simulink model "A_CT_ur10v"  (R2021b)
(part 5 of 11)

t2994 = ct{1294};
t2995 = ct{1295};
t2996 = ct{1296};
t2997 = ct{1297};
t2998 = ct{1298};
t2999 = ct{1299};
t2d = ct{1300};
t2dd = ct{1301};
t30 = ct{1302};
t3004 = ct{1303};
t3005 = ct{1304};
t3007 = ct{1305};
t3008 = ct{1306};
t3009 = ct{1307};
t301 = ct{1308};
t3010 = ct{1309};
t3011 = ct{1310};
t3012 = ct{1311};
t3013 = ct{1312};
t3014 = ct{1313};
t3016 = ct{1314};
t3017 = ct{1315};
t3018 = ct{1316};
t3019 = ct{1317};
t3020 = ct{1318};
t3021 = ct{1319};
t3024 = ct{1320};
t3025 = ct{1321};
t3027 = ct{1322};
t3028 = ct{1323};
t3029 = ct{1324};
t3031 = ct{1325};
t3032 = ct{1326};
t3035 = ct{1327};
t3036 = ct{1328};
t3037 = ct{1329};
t3040 = ct{1330};
t3041 = ct{1331};
t3042 = ct{1332};
t3043 = ct{1333};
t3044 = ct{1334};
t3047 = ct{1335};
t3049 = ct{1336};
t3055 = ct{1337};
t3056 = ct{1338};
t3058 = ct{1339};
t3059 = ct{1340};
t3061 = ct{1341};
t3064 = ct{1342};
t3065 = ct{1343};
t3066 = ct{1344};
t3067 = ct{1345};
t3068 = ct{1346};
t3069 = ct{1347};
t3073 = ct{1348};
t3074 = ct{1349};
t3076 = ct{1350};
t3078 = ct{1351};
t3079 = ct{1352};
t308 = ct{1353};
t3080 = ct{1354};
t3081 = ct{1355};
t3082 = ct{1356};
t3083 = ct{1357};
t3086 = ct{1358};
t3087 = ct{1359};
t3088 = ct{1360};
t3090 = ct{1361};
t3091 = ct{1362};
t3095 = ct{1363};
t3096 = ct{1364};
t3097 = ct{1365};
t3098 = ct{1366};
t3099 = ct{1367};
t31 = ct{1368};
t3100 = ct{1369};
t3101 = ct{1370};
t3104 = ct{1371};
t3106 = ct{1372};
t3107 = ct{1373};
t3110 = ct{1374};
t3111 = ct{1375};
t3112 = ct{1376};
t3121 = ct{1377};
t3123 = ct{1378};
t3124 = ct{1379};
t3125 = ct{1380};
t3129 = ct{1381};
t3130 = ct{1382};
t3134 = ct{1383};
t3136 = ct{1384};
t3137 = ct{1385};
t3140 = ct{1386};
t3143 = ct{1387};
t3146 = ct{1388};
t315 = ct{1389};
t3150 = ct{1390};
t3151 = ct{1391};
t3152 = ct{1392};
t3153 = ct{1393};
t3156 = ct{1394};
t3158 = ct{1395};
t3159 = ct{1396};
t3162 = ct{1397};
t3163 = ct{1398};
t3165 = ct{1399};
t3166 = ct{1400};
t3168 = ct{1401};
t3169 = ct{1402};
t317 = ct{1403};
t3174 = ct{1404};
t3175 = ct{1405};
t3176 = ct{1406};
t3177 = ct{1407};
t3179 = ct{1408};
t318 = ct{1409};
t3182 = ct{1410};
t3183 = ct{1411};
t3185 = ct{1412};
t3187 = ct{1413};
t319 = ct{1414};
t3204 = ct{1415};
t321 = ct{1416};
t3214 = ct{1417};
t3220 = ct{1418};
t3230 = ct{1419};
t3231 = ct{1420};
t3232 = ct{1421};
t3234 = ct{1422};
t3235 = ct{1423};
t3236 = ct{1424};
t3237 = ct{1425};
t3238 = ct{1426};
t3240 = ct{1427};
t3246 = ct{1428};
t325 = ct{1429};
t3250 = ct{1430};
t3251 = ct{1431};
t3259 = ct{1432};
t3260 = ct{1433};
t3272 = ct{1434};
t3283 = ct{1435};
t3285 = ct{1436};
t3288 = ct{1437};
t3289 = ct{1438};
t329 = ct{1439};
t3291 = ct{1440};
t3292 = ct{1441};
t3298 = ct{1442};
t330 = ct{1443};
t3306 = ct{1444};
t3308 = ct{1445};
t331 = ct{1446};
t3318 = ct{1447};
t332 = ct{1448};
t3321 = ct{1449};
t3326 = ct{1450};
t333 = ct{1451};
t3330 = ct{1452};
t3331 = ct{1453};
t3332 = ct{1454};
t3335 = ct{1455};
t3340 = ct{1456};
t3348 = ct{1457};
t3349 = ct{1458};
t3351 = ct{1459};
t3354 = ct{1460};
t3355 = ct{1461};
t3357 = ct{1462};
t3358 = ct{1463};
t3359 = ct{1464};
t3360 = ct{1465};
t3377 = ct{1466};
t3380 = ct{1467};
t3381 = ct{1468};
t3383 = ct{1469};
t3384 = ct{1470};
t3388 = ct{1471};
t3390 = ct{1472};
t3391 = ct{1473};
t3399 = ct{1474};
t34 = ct{1475};
t3400 = ct{1476};
t3401 = ct{1477};
t3404 = ct{1478};
t3405 = ct{1479};
t341 = ct{1480};
t3414 = ct{1481};
t3415 = ct{1482};
t3416 = ct{1483};
t342 = ct{1484};
t3421 = ct{1485};
t3428 = ct{1486};
t3429 = ct{1487};
t343 = ct{1488};
t3431 = ct{1489};
t3432 = ct{1490};
t3439 = ct{1491};
t344 = ct{1492};
t3440 = ct{1493};
t3445 = ct{1494};
t345 = ct{1495};
t3452 = ct{1496};
t3456 = ct{1497};
t3457 = ct{1498};
t3458 = ct{1499};
t3459 = ct{1500};
t346 = ct{1501};
t3460 = ct{1502};
t3461 = ct{1503};
t3464 = ct{1504};
t3468 = ct{1505};
t3469 = ct{1506};
t347 = ct{1507};
t3472 = ct{1508};
t3473 = ct{1509};
t3477 = ct{1510};
t3478 = ct{1511};
t3483 = ct{1512};
t3487 = ct{1513};
t3488 = ct{1514};
t35 = ct{1515};
t3504 = ct{1516};
t3509 = ct{1517};
t3510 = ct{1518};
t3516 = ct{1519};
t3517 = ct{1520};
t3521 = ct{1521};
t3522 = ct{1522};
t3523 = ct{1523};
t3532 = ct{1524};
t354 = ct{1525};
t3543 = ct{1526};
t3544 = ct{1527};
t3546 = ct{1528};
t3555 = ct{1529};
t3556 = ct{1530};
t3557 = ct{1531};
t3562 = ct{1532};
t3567 = ct{1533};
t3568 = ct{1534};
t3574 = ct{1535};
t3575 = ct{1536};
t3577 = ct{1537};
t3578 = ct{1538};
t3579 = ct{1539};
t3580 = ct{1540};
t3582 = ct{1541};
t3590 = ct{1542};
t3598 = ct{1543};
t36 = ct{1544};
t3600 = ct{1545};
t3601 = ct{1546};
t3602 = ct{1547};
t3606 = ct{1548};
t3607 = ct{1549};
t3612 = ct{1550};
t3613 = ct{1551};
t3614 = ct{1552};
t3617 = ct{1553};
t3622 = ct{1554};
t3623 = ct{1555};
t3625 = ct{1556};
t3628 = ct{1557};
t3630 = ct{1558};
t3634 = ct{1559};
t364 = ct{1560};
t3649 = ct{1561};
t365 = ct{1562};
t3651 = ct{1563};
t3674 = ct{1564};
t3678 = ct{1565};
t368 = ct{1566};
t3683 = ct{1567};
t3685 = ct{1568};
t3686 = ct{1569};
t3687 = ct{1570};
t3688 = ct{1571};
t3697 = ct{1572};
t37 = ct{1573};
t3701 = ct{1574};
t3704 = ct{1575};
t3712 = ct{1576};
t3716 = ct{1577};
t3722 = ct{1578};
t3724 = ct{1579};
t3732 = ct{1580};
t3734 = ct{1581};
t3741 = ct{1582};
t3743 = ct{1583};
t3744 = ct{1584};
t3745 = ct{1585};
t3747 = ct{1586};
t3750 = ct{1587};
t3751 = ct{1588};
t3754 = ct{1589};
t3755 = ct{1590};
t3756 = ct{1591};
t3757 = ct{1592};
t3758 = ct{1593};
t3761 = ct{1594};
t3762 = ct{1595};
t3767 = ct{1596};
t3768 = ct{1597};
t3769 = ct{1598};
t3770 = ct{1599};
t3771 = ct{1600};
t3781 = ct{1601};
t3784 = ct{1602};
t3785 = ct{1603};
t3789 = ct{1604};
t3792 = ct{1605};
t3796 = ct{1606};
t38 = ct{1607};
t3804 = ct{1608};
t3812 = ct{1609};
t3813 = ct{1610};
t3817 = ct{1611};
t3821 = ct{1612};
t3822 = ct{1613};
t3826 = ct{1614};
t3828 = ct{1615};
t3830 = ct{1616};
t3833 = ct{1617};
t384 = ct{1618};
t3840 = ct{1619};
t3843 = ct{1620};
t3845 = ct{1621};
t3846 = ct{1622};
t3848 = ct{1623};
t3852 = ct{1624};
t3853 = ct{1625};
t3871 = ct{1626};
t3872 = ct{1627};
t3874 = ct{1628};
t3875 = ct{1629};
t3877 = ct{1630};
t3878 = ct{1631};
t3887 = ct{1632};
t3888 = ct{1633};
t3897 = ct{1634};
t39 = ct{1635};
t3903 = ct{1636};
t3906 = ct{1637};
t3917 = ct{1638};
t392 = ct{1639};
t3923 = ct{1640};
t393 = ct{1641};
t3936 = ct{1642};
t3941 = ct{1643};
t3943 = ct{1644};
t3948 = ct{1645};
t3949 = ct{1646};
t3956 = ct{1647};
t3965 = ct{1648};
t3967 = ct{1649};
t3972 = ct{1650};
t3974 = ct{1651};
t3976 = ct{1652};
t3982 = ct{1653};
t3997 = ct{1654};
t3d = ct{1655};
t3dd = ct{1656};
t4003 = ct{1657};
t4004 = ct{1658};
t4006 = ct{1659};
t4007 = ct{1660};
t401 = ct{1661};
t4012 = ct{1662};
t4018 = ct{1663};
t402 = ct{1664};
t4024 = ct{1665};
t4025 = ct{1666};
t4027 = ct{1667};
t4028 = ct{1668};
t403 = ct{1669};
t404 = ct{1670};
t4042 = ct{1671};
t4048 = ct{1672};
t4049 = ct{1673};
t4050 = ct{1674};
t4055 = ct{1675};
t4058 = ct{1676};
t4059 = ct{1677};
t4069 = ct{1678};
t4071 = ct{1679};
t4076 = ct{1680};
t4077 = ct{1681};
t4084 = ct{1682};
t4085 = ct{1683};
t4086 = ct{1684};
t4096 = ct{1685};
t4098 = ct{1686};
t41 = ct{1687};
t4102 = ct{1688};
t4109 = ct{1689};
t4112 = ct{1690};
t4115 = ct{1691};
t4118 = ct{1692};
t4125 = ct{1693};
t4126 = ct{1694};
t4128 = ct{1695};
t4129 = ct{1696};
t4130 = ct{1697};
t4131 = ct{1698};
t4133 = ct{1699};
t4134 = ct{1700};
t4136 = ct{1701};
t4139 = ct{1702};
t4140 = ct{1703};
t4142 = ct{1704};
t4143 = ct{1705};
t4144 = ct{1706};
t4146 = ct{1707};
t4147 = ct{1708};
t4149 = ct{1709};
t4150 = ct{1710};
t4151 = ct{1711};
t4152 = ct{1712};
t4157 = ct{1713};
t4158 = ct{1714};
t4159 = ct{1715};
t4160 = ct{1716};
t4162 = ct{1717};
t4164 = ct{1718};
t4166 = ct{1719};
t4170 = ct{1720};
t4171 = ct{1721};
t4172 = ct{1722};
t4173 = ct{1723};
t4175 = ct{1724};
t4176 = ct{1725};
t4178 = ct{1726};
t4179 = ct{1727};
t418 = ct{1728};
t4183 = ct{1729};
t4185 = ct{1730};
t4186 = ct{1731};
t4188 = ct{1732};
t419 = ct{1733};
t42 = ct{1734};
t420 = ct{1735};
t4203 = ct{1736};
t4204 = ct{1737};
t4212 = ct{1738};
t4221 = ct{1739};
t4226 = ct{1740};
t4230 = ct{1741};
t4231 = ct{1742};
t4233 = ct{1743};
t4236 = ct{1744};
t4237 = ct{1745};
t425 = ct{1746};
t4252 = ct{1747};
t4256 = ct{1748};
t4268 = ct{1749};
t4273 = ct{1750};
t4290 = ct{1751};
t4296 = ct{1752};
t4299 = ct{1753};
t4304 = ct{1754};
t4309 = ct{1755};
t431 = ct{1756};
t4321 = ct{1757};
t4324 = ct{1758};
t4325 = ct{1759};
t4326 = ct{1760};
t4327 = ct{1761};
t4332 = ct{1762};
t4333 = ct{1763};
t4334 = ct{1764};
t4335 = ct{1765};
t434 = ct{1766};
t4342 = ct{1767};
t4348 = ct{1768};
t4353 = ct{1769};
t4361 = ct{1770};
t4367 = ct{1771};
t437 = ct{1772};
t4381 = ct{1773};
t4386 = ct{1774};
t4394 = ct{1775};
t4395 = ct{1776};
t4397 = ct{1777};
t4403 = ct{1778};
t4406 = ct{1779};
t441 = ct{1780};
t4413 = ct{1781};
t442 = ct{1782};
t4421 = ct{1783};
t4424 = ct{1784};
t4429 = ct{1785};
t443 = ct{1786};
t4430 = ct{1787};
t4442 = ct{1788};
t4443 = ct{1789};
t4451 = ct{1790};
t446 = ct{1791};
t4468 = ct{1792};
t4469 = ct{1793};
t4470 = ct{1794};
t4471 = ct{1795};
t4475 = ct{1796};
t4483 = ct{1797};
t4486 = ct{1798};
t4487 = ct{1799};
t4491 = ct{1800};
t4494 = ct{1801};
t4499 = ct{1802};
t4513 = ct{1803};
t4528 = ct{1804};
t453 = ct{1805};
t4534 = ct{1806};
t4538 = ct{1807};
t4539 = ct{1808};
t454 = ct{1809};
t4540 = ct{1810};
t4541 = ct{1811};
t4547 = ct{1812};
t4548 = ct{1813};
t4551 = ct{1814};
t4556 = ct{1815};
t4560 = ct{1816};
t4573 = ct{1817};
t4579 = ct{1818};
t4582 = ct{1819};
t4584 = ct{1820};
t459 = ct{1821};
t4591 = ct{1822};
t4595 = ct{1823};
t4596 = ct{1824};
t4604 = ct{1825};
t4627 = ct{1826};
t4648 = ct{1827};
t4665 = ct{1828};
t4668 = ct{1829};
t4669 = ct{1830};
t4678 = ct{1831};
t4695 = ct{1832};
t470 = ct{1833};
t4704 = ct{1834};
t4705 = ct{1835};
t4707 = ct{1836};
t4747 = ct{1837};
t4759 = ct{1838};
t4776 = ct{1839};
t478 = ct{1840};
t4785 = ct{1841};
t4787 = ct{1842};
t4789 = ct{1843};
t4798 = ct{1844};
t48 = ct{1845};
t4800 = ct{1846};
t4801 = ct{1847};
t483 = ct{1848};
t4831 = ct{1849};
t4837 = ct{1850};
t4838 = ct{1851};
t484 = ct{1852};
t4853 = ct{1853};
t4856 = ct{1854};
t4858 = ct{1855};
t486 = ct{1856};
t4862 = ct{1857};
t4863 = ct{1858};
t4867 = ct{1859};
t487 = ct{1860};
t4870 = ct{1861};
t488 = ct{1862};
t4881 = ct{1863};
t4887 = ct{1864};
t4889 = ct{1865};
t4893 = ct{1866};
t4907 = ct{1867};
t4908 = ct{1868};
t4917 = ct{1869};
t492 = ct{1870};
t4921 = ct{1871};
t4923 = ct{1872};
t4924 = ct{1873};
t493 = ct{1874};
t4930 = ct{1875};
t4931 = ct{1876};
t494 = ct{1877};
t4940 = ct{1878};
t4941 = ct{1879};
t4944 = ct{1880};
t4949 = ct{1881};
t495 = ct{1882};
t4950 = ct{1883};
t4955 = ct{1884};
t4957 = ct{1885};
t496 = ct{1886};
t497 = ct{1887};
t4979 = ct{1888};
t498 = ct{1889};
t4985 = ct{1890};
t4990 = ct{1891};
t4992 = ct{1892};
t4d = ct{1893};
t4dd = ct{1894};
t50 = ct{1895};
t5006 = ct{1896};
t501 = ct{1897};
t5010 = ct{1898};
t5012 = ct{1899};
t5018 = ct{1900};
t5020 = ct{1901};
t503 = ct{1902};
t5047 = ct{1903};
t5051 = ct{1904};
t5056 = ct{1905};
t5074 = ct{1906};
t508 = ct{1907};
t5093 = ct{1908};
t51 = ct{1909};
t5106 = ct{1910};
t5114 = ct{1911};
t514 = ct{1912};
t515 = ct{1913};
t516 = ct{1914};
t519 = ct{1915};
t523 = ct{1916};
t524 = ct{1917};
t5283 = ct{1918};
t529 = ct{1919};
t5292 = ct{1920};
t53 = ct{1921};
t530 = ct{1922};
t532 = ct{1923};
t537 = ct{1924};
t543 = ct{1925};
t544 = ct{1926};
t546 = ct{1927};
t5465 = ct{1928};
t547 = ct{1929};
t548 = ct{1930};
t549 = ct{1931};
t55 = ct{1932};
t552 = ct{1933};
t553 = ct{1934};
t554 = ct{1935};
t56 = ct{1936};
t562 = ct{1937};
t569 = ct{1938};
t57 = ct{1939};
t570 = ct{1940};
t58 = ct{1941};
t582 = ct{1942};
t588 = ct{1943};
t589 = ct{1944};
t591 = ct{1945};
t593 = ct{1946};
t596 = ct{1947};
t598 = ct{1948};
t5d = ct{1949};
t5dd = ct{1950};
t601 = ct{1951};
t602 = ct{1952};
t604 = ct{1953};
t608 = ct{1954};
t609 = ct{1955};
t61 = ct{1956};
t612 = ct{1957};
t614 = ct{1958};
t615 = ct{1959};
t616 = ct{1960};
t617 = ct{1961};
t623 = ct{1962};
t627 = ct{1963};
t63 = ct{1964};
t632 = ct{1965};
t633 = ct{1966};
t634 = ct{1967};
t635 = ct{1968};
t636 = ct{1969};
t637 = ct{1970};
t639 = ct{1971};
t641 = ct{1972};
t642 = ct{1973};
t643 = ct{1974};
t644 = ct{1975};
t645 = ct{1976};
t646 = ct{1977};
t647 = ct{1978};
t648 = ct{1979};
t649 = ct{1980};
t650 = ct{1981};
t652 = ct{1982};
t653 = ct{1983};
t655 = ct{1984};
t659 = ct{1985};
t664 = ct{1986};
t665 = ct{1987};
t667 = ct{1988};
t668 = ct{1989};
t670 = ct{1990};
t671 = ct{1991};
t675 = ct{1992};
t680 = ct{1993};
t681 = ct{1994};
t682 = ct{1995};
t684 = ct{1996};
t685 = ct{1997};
t687 = ct{1998};
t689 = ct{1999};
t69 = ct{2000};
t690 = ct{2001};
t691 = ct{2002};
t694 = ct{2003};
t695 = ct{2004};
t696 = ct{2005};
t698 = ct{2006};
t699 = ct{2007};
t6d = ct{2008};
t6dd = ct{2009};
t701 = ct{2010};
t702 = ct{2011};
t703 = ct{2012};
t705 = ct{2013};
t706 = ct{2014};
t71 = ct{2015};
t711 = ct{2016};
t712 = ct{2017};
t713 = ct{2018};
t714 = ct{2019};
t720 = ct{2020};
t721 = ct{2021};
t723 = ct{2022};
t725 = ct{2023};
t726 = ct{2024};
t729 = ct{2025};
t731 = ct{2026};
t732 = ct{2027};
t733 = ct{2028};
t735 = ct{2029};
t736 = ct{2030};
t738 = ct{2031};
t739 = ct{2032};
t745 = ct{2033};
t746 = ct{2034};
t747 = ct{2035};
t748 = ct{2036};
t75 = ct{2037};
t752 = ct{2038};
t755 = ct{2039};
t759 = ct{2040};
t760 = ct{2041};
t761 = ct{2042};
t763 = ct{2043};
t764 = ct{2044};
t772 = ct{2045};
t774 = ct{2046};
t775 = ct{2047};
t776 = ct{2048};
t781 = ct{2049};
t785 = ct{2050};
t788 = ct{2051};
t789 = ct{2052};
t793 = ct{2053};
t8 = ct{2054};
t802 = ct{2055};
t806 = ct{2056};
t82 = ct{2057};
t820 = ct{2058};
t823 = ct{2059};
t824 = ct{2060};
t825 = ct{2061};
t826 = ct{2062};
t827 = ct{2063};
t828 = ct{2064};
t831 = ct{2065};
t832 = ct{2066};
t833 = ct{2067};
t838 = ct{2068};
t842 = ct{2069};
t843 = ct{2070};
t844 = ct{2071};
t846 = ct{2072};
t848 = ct{2073};
t849 = ct{2074};
t850 = ct{2075};
t851 = ct{2076};
t852 = ct{2077};
t853 = ct{2078};
t854 = ct{2079};
t855 = ct{2080};
t859 = ct{2081};
t861 = ct{2082};
t865 = ct{2083};
t870 = ct{2084};
t871 = ct{2085};
t873 = ct{2086};
t879 = ct{2087};
t880 = ct{2088};
t884 = ct{2089};
t885 = ct{2090};
t890 = ct{2091};
t892 = ct{2092};
t896 = ct{2093};
t897 = ct{2094};
t898 = ct{2095};
t899 = ct{2096};
t9 = ct{2097};
t900 = ct{2098};
t907 = ct{2099};
t908 = ct{2100};
t909 = ct{2101};
t910 = ct{2102};
t915 = ct{2103};
t917 = ct{2104};
t919 = ct{2105};
t922 = ct{2106};
t923 = ct{2107};
t927 = ct{2108};
t928 = ct{2109};
t930 = ct{2110};
t932 = ct{2111};
t937 = ct{2112};
t943 = ct{2113};
t944 = ct{2114};
t945 = ct{2115};
t949 = ct{2116};
t952 = ct{2117};
t959 = ct{2118};
t961 = ct{2119};
t962 = ct{2120};
t963 = ct{2121};
t964 = ct{2122};
t965 = ct{2123};
t966 = ct{2124};
t967 = ct{2125};
t969 = ct{2126};
t970 = ct{2127};
t972 = ct{2128};
t973 = ct{2129};
t976 = ct{2130};
t978 = ct{2131};
t979 = ct{2132};
t981 = ct{2133};
t982 = ct{2134};
t983 = ct{2135};
t986 = ct{2136};
t987 = ct{2137};
t989 = ct{2138};
t992 = ct{2139};
t996 = ct{2140};
t999 = ct{2141};
t3192 = t3165.*(-1.0./2.0);
t3194 = t1798+t1828;
t3195 = t3152.*t2dd;
t3196 = t3152.*t3dd;
t3197 = t3152.*t4dd;
t3244 = t14.*t39.*(t1853-t908.*(t101-t401));
t3253 = t256.*t3027;
t3258 = (t1265.*t2361)./2.0;
t3267 = t3235./2.0;
t3268 = t3238./2.0;
t3275 = t330.*t3027;
t3278 = t255.*t3036;
t3302 = t329.*t3036;
t3305 = t1825+t1997;
t3313 = t1894+t1947;
t3319 = t1556+t2257;
t3322 = t1565+t2265;
t3323 = t1865+t1991;
t3339 = t255.*(t1853-t908.*(t101-t401));
t3367 = t1974+t2032;
t3378 = -t3357;
t3387 = t3359./2.0;
t3403 = t1206+t1471+t1474;
t3417 = t14.*(t1864-t2028).*(-1.0./2.0);
t3441 = -t8.*t39.*(t1864-t2028);
t3444 = t132+t345+t614+t684+t1022+t1072;
t3451 = t1602+t2440;
t3453 = t3428.*t2d;
t3454 = t3428.*t3d;
t3455 = t3428.*t4d;
t3463 = t1603+t2448;
t3474 = t8.*t39.*(t1864-t2028);
t3475 = t18.*t39.*t3377;
t3479 = t3464.*t2d;
t3480 = t3464.*t3d;
t3481 = t3464.*t4d;
t3490 = -t14.*(t1597-t2409);
t3493 = -t8.*(t1609-t2416);
t3495 = -t3478;
t3499 = t1799+t2358;
t3502 = t321+t642+t644+t1300+t1304;
t3503 = t3478./2.0;
t3506 = t8.*t3487;
t3508 = t2096+t2114;
t3515 = t14.*(t1597-t2409).*(-1.0./2.0);
t3518 = t8.*(t1609-t2416).*(-1.0./2.0);
t3527 = t1371+t1374+t1656;
t3530 = -t8.*t39.*(t1597-t2409);
t3534 = t2111+t2138;
t3536 = t3522.*t2d;
t3537 = t3522.*t3d;
t3538 = t3522.*t4d;
t3539 = -t14.*t39.*(t1609-t2416);
t3540 = -t3521;
t3547 = t3521./2.0;
t3549 = -t330.*(t1864-t2028);
t3551 = t255.*t3377;
t3558 = t14.*t39.*t3487;
t3559 = t8.*t39.*(t1597-t2409);
t3563 = t1935.*t2361;
t3565 = t1325+t1449+t1697;
t3569 = t2121+t2165;
t3571 = t14.*t39.*(t1609-t2416).*(-1.0./2.0);
t3573 = t330.*t3377;
t3586 = t3562.*t2d;
t3587 = t3562.*t3d;
t3588 = t3562.*t4d;
t3589 = t2139+t2166;
t3591 = t1916+t2376;
t3596 = t330.*(t1864-t2028).*(-1.0./2.0);
t3603 = t1536+t2681;
t3604 = t341.*t3377;
t3609 = t37.*t3532;
t3610 = (t330.*(t1864-t2028))./2.0;
t3611 = t39.*t3532;
t3615 = t2163+t2164;
t3620 = t689+t1816+t1887;
t3624 = t402.*t3377;
t3626 = -t3607;
t3627 = t2152+t2202;
t3635 = t3614.*t2dd;
t3637 = t3614.*t3dd;
t3639 = t3614.*t4dd;
t3650 = -t255.*(t1609-t2416);
t3668 = t37.*t3602;
t3670 = t39.*t3602;
t3675 = t255.*t3487;
t3682 = t255.*(t1609-t2416).*(-1.0./2.0);
t3684 = t3651./2.0;
t3690 = t2226+t2227;
t3733 = t1436+t1554+t1689;
t3739 = t609.*t3377;
t3753 = t641.*t3377;
t3763 = t2241+t2324;
t3764 = t1445+t1598+t1693;
t3766 = -t3377.*(t100-t364);
t3780 = -t3377.*(t101-t401);
t3783 = t2268+t2345;
t3787 = t3762.*t6d;
t3791 = t2095+t2488;
t3800 = t2092+t2526;
t3809 = t3781./2.0;
t3810 = -t8.*(t2068-t2488);
t3811 = t14.*t3789;
t3832 = t1723+t2823;
t3838 = t8.*(t2068-t2488).*(-1.0./2.0);
t3851 = t1801+t2782;
t3858 = t3828./2.0;
t3860 = t8.*t37.*t3789;
t3861 = t8.*t39.*t3789;
t3863 = -t14.*t37.*(t2068-t2488);
t3864 = -t14.*t39.*(t2068-t2488);
t3866 = t2135+t2590;
t3867 = t8.*t3833;
t3880 = t35.*t39.*t3789;
t3886 = -t38.*t39.*(t2068-t2488);
t3889 = t14.*t39.*(t2068-t2488);
t3890 = t3848./2.0;
t3892 = t18.*t39.*t3804;
t3893 = t2183+t2550;
t3894 = -t3874;
t3896 = t8.*(t2782-t1070.*(t101-t401));
t3900 = t14.*t37.*(t2068-t2488).*(-1.0./2.0);
t3919 = -t3888;
t3927 = t14.*t37.*t3833;
t3931 = t14.*t39.*t3833;
t3932 = t38.*t39.*(t2068-t2488).*(-1.0./2.0);
t3933 = t3887./2.0;
t3937 = t8.*(t2550-t1535.*(t101-t401));
t3950 = t18.*t39.*t3845;
t3958 = t38.*t39.*t3833;
t3959 = t14.*t37.*(t2782-t1070.*(t101-t401));
t3962 = t14.*t39.*(t2782-t1070.*(t101-t401));
t3963 = t3917./2.0;
t3978 = t3936./2.0;
t3980 = -t3965;
t3983 = t38.*t39.*(t2782-t1070.*(t101-t401));
t3989 = -t255.*(t2068-t2488);
t3990 = -t3982;
t3993 = t2451+t2452;
t3994 = t1059+t1111+t1323+t1658;
t4001 = t255.*t3804;
t4002 = t3972./2.0;
t4005 = t330.*t3789;
t4014 = t330.*t3804;
t4017 = t341.*t3804;
t4019 = t255.*t3845;
t4023 = t402.*t3804;
t4026 = -t3081.*(t745-t747);
t4030 = t330.*t3845;
t4038 = t341.*t3845;
t4041 = t3081.*(t745-t747).*(-1.0./2.0);
t4045 = t402.*t3845;
t4046 = t37.*t4018;
t4047 = (t3081.*(t745-t747))./2.0;
t4053 = t18.*t39.*t4018;
t4066 = t1173+t1212+t1448+t1718;
t4067 = t609.*t3804;
t4068 = t2580+t2582;
t4073 = -t3804.*(t100-t364);
t4074 = t641.*t3804;
t4078 = t2558+t2636;
t4081 = t609.*t3845;
t4082 = -t3804.*(t101-t401);
t4087 = t4077.*t5dd;
t4088 = -t3845.*(t100-t364);
t4090 = t641.*t3845;
t4091 = t3804.*(t101-t401);
t4095 = -t4085;
t4097 = t3845.*(t100-t364);
t4099 = -t3845.*(t101-t401);
t4101 = t4085./2.0;
t4113 = t3845.*(t101-t401);
t4117 = -t4109;
t4121 = t4109./2.0;
t4122 = -t4118;
t4137 = t4128./2.0;
t4138 = -t4136;
t4145 = t772+t1164+t1569+t2221;
t4148 = t774+t1166+t1571+t2228;
t4155 = t2687+t2713;
t4156 = t2270.*t3081;
t4167 = t2684+t2750;
t4168 = t2715+t2716;
t4174 = t4164.*t6d;
t4180 = -t4171;
t4182 = t2738+t2740;
t4187 = -t4173;
t4189 = -t4175;
t4192 = t4173./2.0;
t4193 = -t4188;
t4194 = t4175./2.0;
t4195 = t2727+t2751;
t4196 = t2717+t2768;
t4202 = t2720+t2799;
t4208 = t1343+t1389+t1546+t1859;
t4215 = t826+t1414+t1558+t2260;
t4217 = t825+t1415+t1557+t2262;
t4220 = t827+t1416+t1562+t2264;
t4222 = t1294+t1339+t1637+t1917;
t4225 = t823+t1417+t1555+t2256;
t4251 = t2529.*t3081;
t4255 = t1437+t1447+t1690+t1696;
t4267 = -t4252;
t4283 = t4252./2.0;
t4294 = t4273.*t5d;
t4302 = t4268.*t5d;
t4330 = t2836+t2916;
t4331 = t2863+t2895;
t4337 = t4324.*t6d;
t4351 = t243+t283+t685+t701+t1019+t1064+t1078+t1100;
t4371 = -t4367;
t4393 = t2020+t2250+t2291;
t4398 = t3008+t3021;
t4399 = t4397.*t5dd;
t4402 = t3016+t3041;
t4404 = t3024+t3042;
t4408 = t3020+t3061;
t4410 = t3031+t3064;
t4426 = t4421.*(-1.0./2.0);
t4428 = t3056+t3097;
t4431 = t4421./2.0;
t4440 = t4429.*(-1.0./2.0);
t4444 = t4429./2.0;
t4450 = -t4049.*(t745-t747);
t4454 = -t4442;
t4457 = -t4443;
t4459 = t4442./2.0;
t4460 = t4443./2.0;
t4461 = t3081.*(t503.*1.383e-1+t731+t981+t999);
t4467 = t4049.*(t745-t747).*(-1.0./2.0);
t4472 = t2083+t2429+t2459;
t4479 = t4471.*t6dd;
t4480 = -t6dd.*(t2057-t2429+t1858.*(t100-t364));
t4493 = (t1874.*t4049)./2.0;
t4500 = t2583+t3704;
t4503 = t1735+t1880+t1881+t1882;
t4508 = t2703+t3625;
t4512 = t3235+t3238;
t4526 = t1641+t1708+t1797+t2356;
t4529 = t2621+t3813;
t4531 = t37.*t4513;
t4533 = t3081.*t3404;
t4542 = t18.*t39.*t4513;
t4549 = t2607+t3852;
t4553 = t4534./2.0;
t4561 = t2270.*t4049;
t4563 = t2609+t3878;
t4566 = t1560+t1561+t2261+t2263;
t4592 = t14.*t4573;
t4599 = t4582./2.0;
t4607 = t8.*t4584;
t4608 = -t14.*(t3377.*(t100-t364)+t13.*t330.*(t544-t1021+t330.*(t100-t364)));
t4613 = t14.*(t1794-t1990+t2029+t1274.*(t100-t364)).*(-1.0./2.0);
t4615 = (t14.*(t1794-t1990+t2029+t1274.*(t100-t364)))./2.0;
t4620 = t8.*t39.*t4573;
t4623 = t14.*(t3377.*(t100-t364)+t13.*t330.*(t544-t1021+t330.*(t100-t364))).*(-1.0./2.0);
t4624 = -t8.*t39.*(t1794-t1990+t2029+t1274.*(t100-t364));
t4626 = t2529.*t4049;
t4629 = t8.*(t1929-t1996+t2033+t1187.*(t101-t401)).*(-1.0./2.0);
t4632 = t14.*t39.*t4584;
t4633 = t8.*t39.*(t1794-t1990+t2029+t1274.*(t100-t364));
t4642 = -t4627;
t4643 = -t14.*t39.*(t1929-t1996+t2033+t1187.*(t101-t401));
t4647 = t4627./2.0;
t4655 = t14.*t39.*(t1929-t1996+t2033+t1187.*(t101-t401));
t4664 = (t3081.*t3686)./2.0;
t4666 = t4648./2.0;
t4670 = t330.*t4573;
t4672 = t4668./2.0;
t4673 = t255.*t4584;
t4675 = -t330.*(t1794-t1990+t2029+t1274.*(t100-t364));
t4676 = (t3081.*t3734)./2.0;
t4677 = -t255.*(t1929-t1996+t2033+t1187.*(t101-t401));
t4681 = t330.*(t1794-t1990+t2029+t1274.*(t100-t364));
t4683 = t1604+t1605+t2442+t2447;
t4688 = t1600+t1601+t2441+t2449;
t4693 = t255.*(t1929-t1996+t2033+t1187.*(t101-t401)).*(-1.0./2.0);
t4694 = t4678./2.0;
t4699 = (t255.*(t1929-t1996+t2033+t1187.*(t101-t401)))./2.0;
t4703 = t3081.*t3821;
t4708 = t1779+t1845+t2067+t2525;
t4714 = t4704./2.0;
t4715 = t1806+t1907+t2064+t2489;
t4716 = t4705./2.0;
t4720 = t4707./2.0;
t4722 = t1809+t1886+t2027+t2555;
t4727 = t1781+t1834+t2091+t2592;
t4749 = t552+t961+t1283+t1314+t2200+t2208;
t4757 = t4747./2.0;
t4765 = t4759./2.0;
t4771 = t2270.*t4333;
t4775 = -t14.*(t3804.*(t100-t364)+t453.*(t544-t1021+t330.*(t100-t364)));
t4779 = t598+t962+t1329+t1360+t2207+t2271;
t4786 = t14.*(t3804.*(t100-t364)+t453.*(t544-t1021+t330.*(t100-t364)));
t4792 = t4776./2.0;
t4795 = -t8.*t39.*(t3804.*(t100-t364)+t453.*(t544-t1021+t330.*(t100-t364)));
t4799 = t3081.*t4049;
t4802 = t4789./2.0;
t4812 = t8.*t39.*(t3804.*(t100-t364)+t453.*(t544-t1021+t330.*(t100-t364))).*(-1.0./2.0);
t4813 = t4798./2.0;
t4815 = t4049.*(t503.*1.383e-1+t731+t981+t999);
t4817 = (t8.*t39.*(t3804.*(t100-t364)+t453.*(t544-t1021+t330.*(t100-t364))))./2.0;
t4836 = t14.*t1807.*t4469;
t4840 = -t4838;
t4842 = -t330.*(t3804.*(t100-t364)+t453.*(t544-t1021+t330.*(t100-t364)));
t4845 = t330.*(t3804.*(t100-t364)+t453.*(t544-t1021+t330.*(t100-t364)));
t4846 = t596+t1039+t1307+t1376+t2365+t2370;
t4855 = t3081.*t4130;
t4859 = t4853./2.0;
t4861 = t4856./2.0;
t4865 = t14.*t2113.*t4469;
t4869 = t665+t1007+t1377+t1396+t2397+t2402;
t4871 = t4863./2.0;
t4874 = -t4870;
t4878 = t3767+t3769;
t4883 = t14.*t2279.*t4469;
t4891 = -t4889;
t4896 = t4893.*t5d;
t4909 = -t4907;
t4920 = t1089+t1092+t4560;
t4922 = t3081.*t4333;
t4926 = t4923.*2.0;
t4929 = (t3686.*t4049)./2.0;
t4932 = t2654.*t4469;
t4935 = t3734.*t4049;
t4945 = -t4941;
t4946 = t3948+t3949;
t4951 = -t4949;
t4952 = t4949./2.0;
t4956 = (t3821.*t4049)./2.0;
t4958 = -t4955;
t4959 = t4955./2.0;
t4967 = t4024+t4028;
t4981 = t1316+t2245+t2679+t3477;
t4993 = -t4469.*(t910-t2473);
t4997 = t4469.*(t910-t2473);
t5001 = t1330+t1352+t4669;
t5011 = t3251.*t4469;
t5013 = -t5010;
t5019 = t4049.*t4130;
t5026 = t5020./2.0;
t5036 = t1800+t2418+t2535+t3612;
t5038 = -t37.*(t1873+t2355+t2471+t3579);
t5040 = -t18.*t39.*(t1873+t2355+t2471+t3579);
t5041 = t37.*(t1873+t2355+t2471+t3579).*(-1.0./2.0);
t5043 = t18.*t39.*(t1873+t2355+t2471+t3579).*(-1.0./2.0);
t5070 = -t1d.*(-t1842+t2432+t2548+(t18.*t39.*(-t495-t548+t650+t659+t739+t14.*t37.*(t101-t401)))./2.0);
t5081 = t2109+t2118+t3231+t3237;
t5091 = t1871+t2377+t2653+t3674;
t5092 = t4049.*t4333;
t5098 = t5093./2.0;
t5104 = -t14.*(t1862+t2375+t330.*(-t496-t547+t615+t623+t755+t8.*t37.*(t100-t364))+t2124.*(t100-t364));
t5115 = t14.*(t1862+t2375+t330.*(-t496-t547+t615+t623+t755+t8.*t37.*(t100-t364))+t2124.*(t100-t364)).*(-1.0./2.0);
t5116 = t14.*t5106;
t5117 = (t14.*(t1862+t2375+t330.*(-t496-t547+t615+t623+t755+t8.*t37.*(t100-t364))+t2124.*(t100-t364)))./2.0;
t5119 = -t8.*t39.*(t1862+t2375+t330.*(-t496-t547+t615+t623+t755+t8.*t37.*(t100-t364))+t2124.*(t100-t364));
t5123 = t8.*t5114;
t5131 = t8.*t39.*(t1862+t2375+t330.*(-t496-t547+t615+t623+t755+t8.*t37.*(t100-t364))+t2124.*(t100-t364)).*(-1.0./2.0);
t5136 = t8.*t39.*t5106;
t5140 = t668+t1429+t1815+t1884+t2857+t2891;
t5141 = t14.*t39.*t5114;
t5163 = -t330.*(t1862+t2375+t330.*(-t496-t547+t615+t623+t755+t8.*t37.*(t100-t364))+t2124.*(t100-t364));
t5171 = t330.*(t1862+t2375+t330.*(-t496-t547+t615+t623+t755+t8.*t37.*(t100-t364))+t2124.*(t100-t364)).*(-1.0./2.0);
t5175 = t330.*t5106;
t5176 = t255.*t5114;
t5212 = t4326+t4342;
t5219 = t4381+t4386;
t5223 = t643+t1038+t1383+t1411+t1948+t1951+t2420+t2424;
t5255 = t2839+t2849+t3380+t3381;
t5258 = t2543+t2611+t3724+t3758;
t5278 = t2628+t2629+t3853+t3906;
t5281 = t2631+t2632+t3877+t3941;
t5351 = t3250+t3259+t4800;
t5401 = t3678+t3688+t3974+t4004;
t5403 = t3743+t3761+t4055+t4058;
t5463 = t4179+t4921+t4940;
t5476 = t3546+t3567+t4787+t4789;
t5501 = t3796+t3846+t4853+t4863;
t5513 = t4076+t4098+t4853+t4863;
t5516 = t4129+t4150+t4853+t4863;
t1397 = -t1385;
t1479 = t1428./2.0;
t1489 = -t1464;
t1513 = t1464./2.0;
t1748 = -t1721;
t1787 = -t1764;
t1789 = t1725./2.0;
t1833 = -t1802;
t1836 = -t1803;
t1838 = t1796./2.0;
t1850 = t1802./2.0;
t1939 = t1849./2.0;
t1956 = t1883.*t2d;
t1957 = t1883.*t3d;
t1958 = t1883.*t4d;
t2002 = -t1980;
t2005 = -t1982;
t2036 = -t2014;
t2088 = -t2071;
t2115 = -t2098;
t2129 = -t2102;
t2130 = t2107.*t1dd;
t2176 = t1088+t1132;
t2182 = t1091+t1136;
t2186 = t37.*t2105;
t2187 = t37.*t2107;
t2188 = t37.*t2108;
t2191 = t39.*t2107;
t2266 = (t14.*t2154)./2.0;
t2269 = (t8.*t2157)./2.0;
t2290 = t14.*t39.*t2157;
t2310 = t8.*t39.*t2154;
t2328 = t2296.*t5d;
t2364 = -t2351;
t2386 = -t2369;
t2419 = -t2396;
t2430 = -t2392;
t2431 = -t2394;
t2445 = t2392./2.0;
t2446 = t2394./2.0;
t2510 = t1003+t1608;
t2514 = t1002+t1612;
t2528 = -t2494;
t2544 = t2492./2.0;
t2545 = t2494./2.0;
t2552 = -t2522;
t2563 = t8.*t2512;
t2568 = t14.*t2513;
t2570 = t2521.*t1d;
t2575 = -t2541;
t2591 = -t2551;
t2596 = -t2584;
t2602 = -t2588;
t2605 = -t2574;
t2614 = -t2587;
t2617 = -t2589;
t2626 = t2587./2.0;
t2627 = t2589./2.0;
t2640 = t8.*t37.*t2513;
t2641 = t14.*t37.*t2512;
t2665 = -t2656;
t2691 = -t2675;
t2732 = t331+t1313+t1363;
t2733 = t1324+t1700;
t2763 = t976+t996+t1012;
t2773 = -t2757;
t2791 = t2752.*t2d;
t2792 = t2752.*t3d;
t2793 = t2752.*t4d;
t2811 = t1402+t1744;
t2832 = t2804.*t1d;
t2845 = t18.*t2810;
t2847 = t12.*t2815;
t2851 = t18.*t2815;
t2861 = t2827.*t1d;
t2864 = t2806./2.0;
t2870 = t2810./2.0;
t2873 = t2815./2.0;
t2875 = -t2858;
t2898 = t2840./2.0;
t2902 = -t2885;
t2918 = -t2893;
t2926 = t39.*t2828;
t2930 = t1623+t1624;
t2950 = -t2933;
t2957 = t2928.*t1d;
t2972 = (t37.*t2828)./2.0;
t2981 = t2935./2.0;
t3000 = t2961./2.0;
t3003 = t2968./2.0;
t3006 = t2975./2.0;
t3048 = t8.*t3019;
t3050 = -t3040;
t3052 = t3025./2.0;
t3057 = t1725+t1775;
t3075 = t14.*t3047;
t3085 = t3049./2.0;
t3089 = t1633+t1852;
t3092 = t3067.*t5d;
t3093 = t3068.*t5d;
t3108 = t3074./2.0;
t3113 = t14.*t37.*t3019;
t3115 = t14.*t39.*t3019;
t3116 = t1646+t1913;
t3120 = -t3095;
t3126 = -t3111;
t3135 = t14.*t3091;
t3138 = t8.*t37.*t3047;
t3139 = -t3110;
t3141 = t8.*t39.*t3047;
t3142 = t38.*t39.*t3019;
t3155 = t8.*t3104;
t3157 = t3110./2.0;
t3161 = t3112./2.0;
t3170 = t3134.*t2d;
t3171 = t3134.*t3d;
t3172 = t3134.*t4d;
t3173 = t14.*(t1913-t898.*(t100-t364));
t3180 = t35.*t39.*t3047;
Y = ft_8({t100,t1004,t1007,t1009,t101,t1015,t1016,t1017,t1019,t1021,t1026,t1028,t1031,t1035,t1036,t104,t1044,t1045,t1046,t1047,t1048,t1049,t1053,t1054,t1055,t106,t1064,t1066,t1068,t1069,t107,t1070,t1071,t1079,t108,t1080,t1081,t1082,t1083,t1084,t1085,t1086,t1087,t1093,t1094,t1096,t1097,t1098,t1099,t1101,t1106,t1108,t1109,t111,t1110,t112,t1121,t1122,t1123,t1125,t1126,t1128,t1129,t113,t1133,t1134,t1135,t1137,t1138,t1139,t1140,t1143,t1147,t1148,t1152,t1155,t1156,t1158,t1160,t1162,t1171,t1172,t1174,t1181,t1182,t1183,t1184,t1185,t1186,t1187,t1189,t1191,t1193,t1196,t12,t1203,t1207,t1208,t1209,t1210,t1211,t1222,t1224,t1225,t1226,t1227,t1229,t1230,t1235,t1236,t1237,t1238,t124,t1245,t1246,t1247,t1248,t1249,t1250,t1251,t1252,t1255,t1264,t1265,t1266,t1268,t127,t1271,t1272,t1273,t128,t1281,t1282,t1284,t1285,t1286,t1287,t1288,t1289,t1292,t1297,t1298,t13,t1302,t1306,t131,t1311,t1312,t1316,t1317,t132,t1321,t1328,t1331,t1332,t1333,t1334,t1335,t1336,t1337,t134,t1341,t1346,t1347,t1348,t1350,t1353,t1355,t1356,t1357,t1358,t1359,t136,t1361,t1366,t1367,t1368,t1369,t137,t1375,t1378,t1379,t138,t1382,t1387,t1388,t1391,t1392,t1393,t1395,t1397,t1398,t1399,t14,t1400,t1403,t1406,t1408,t1410,t1412,t1413,t1418,t1419,t1420,t1423,t1425,t1427,t1428,t1430,t1434,t1435,t1438,t1440,t1451,t1457,t1458,t1461,t1464,t1465,t1468,t1470,t1472,t1473,t1475,t1476,t1477,t1478,t1479,t1480,t1483,t1484,t1485,t1486,t1489,t1491,t1492,t1493,t1496,t1497,t1499,t15,t150,t1500,t1501,t1503,t1504,t1507,t1513,t1514,t1516,t1517,t1518,t1519,t152,t1520,t1521,t1524,t1525,t1527,t1528,t1529,t1531,t1532,t1534,t1535,t1536,t1537,t1538,t1547,t1549,t155,t1553,t156,t1569,t1571,t1572,t1574,t1577,t1578,t1579,t158,t1580,t1583,t1585,t1586,t1588,t1589,t159,t1590,t1591,t1594,t1597,t1599,t1606,t1607,t1609,t1610,t1611,t1613,t1614,t1615,t1616,t1617,t1618,t1619,t162,t1620,t1621,t1622,t1625,t1627,t1628,t163,t1630,t1631,t1632,t1634,t1635,t1636,t1638,t164,t1642,t1643,t1645,t1647,t1648,t1649,t165,t1650,t1651,t1652,t1653,t1654,t1659,t1660,t1663,t1664,t1665,t1667,t1670,t1671,t1672,t1674,t1675,t1677,t1678,t1680,t1681,t1682,t1683,t1685,t1686,t1687,t1688,t1691,t1692,t1698,t1699,t1701,t1704,t1706,t1707,t1709,t171,t1710,t1713,t1714,t1715,t1717,t1719,t1722,t1724,t173,t1733,t1736,t1738,t174,t1740,t1741,t1742,t1743,t1746,t1747,t1748,t175,t1751,t1754,t1755,t1758,t1759,t1760,t1763,t1766,t1767,t177,t1776,t1780,t1782,t1783,t1784,t1786,t1787,t1789,t1790,t1792,t1796,t1797,t1799,t18,t1800,t1803,t1807,t1813,t1814,t1815,t1816,t1818,t1824,t1826,t1827,t1829,t1830,t1832,t1833,t1835,t1836,t1837,t1838,t1840,t1841,t1842,t1844,t1846,t1848,t1849,t1850,t1851,t1854,t1860,t1862,t1863,t1864,t1866,t1867,t1868,t1869,t187,t1873,t1874,t1875,t1876,t1877,t1878,t1879,t1888,t1889,t1890,t1891,t1892,t1893,t1899,t19,t1900,t1901,t1902,t1903,t1904,t1905,t191,t1911,t1912,t1913,t1915,t1916,t1918,t1919,t1920,t1921,t1923,t1925,t1926,t1927,t1929,t1930,t1933,t1934,t1935,t1936,t1938,t1939,t1940,t1941,t1944,t1945,t1948,t1949,t1951,t1952,t1956,t1957,t1958,t1959,t1960,t1961,t1962,t1963,t1964,t1965,t1966,t1967,t1968,t1969,t1970,t1971,t1972,t1973,t1975,t1976,t1977,t1978,t1979,t1981,t1983,t1984,t1985,t1988,t199,t1990,t1992,t1993,t1995,t1996,t1999,t1d,t1dd,t200,t2000,t2001,t2002,t2004,t2005,t2009,t201,t2010,t2012,t2013,t2015,t2016,t2018,t202,t2021,t2022,t2023,t2024,t2026,t2028,t2031,t2033,t2036,t2042,t2044,t2053,t2054,t2059,t206,t2060,t2061,t2062,t2065,t2068,t2069,t2070,t2072,t2074,t2075,t2079,t2080,t2081,t2085,t2086,t2087,t2088,t2090,t2093,t2098,t2099,t21,t2100,t2101,t2104,t2105,t2107,t2108,t2112,t2113,t2115,t2117,t2119,t2122,t2123,t2124,t2126,t2128,t2129,t2130,t2132,t2136,t2140,t2141,t2142,t2143,t2144,t2145,t2146,t2147,t215,t2150,t2153,t2155,t2156,t2159,t2160,t2162,t2167,t2168,t2169,t2170,t2171,t2173,t2174,t2176,t2178,t2180,t2181,t2182,t2184,t2186,t2187,t2188,t2189,t219,t2190,t2191,t2193,t2194,t2196,t2198,t22,t220,t2204,t2206,t221,t2210,t2213,t2216,t2219,t2220,t2222,t2223,t2224,t2225,t2229,t2230,t2233,t2235,t2242,t2243,t2244,t2246,t2247,t2249,t2259,t226,t2266,t2267,t2269,t2270,t2278,t2279,t2281,t2282,t2283,t2284,t2286,t2289,t229,t2290,t2292,t2293,t2294,t2295,t2296,t23,t2300,t2304,t2305,t2306,t2307,t2308,t2310,t2311,t2314,t2317,t2319,t232,t2320,t2321,t2322,t2325,t2326,t2327,t2328,t2329,t233,t2330,t2331,t2332,t2339,t2340,t2344,t2346,t2348,t2349,t2351,t2352,t2353,t2354,t2355,t2356,t2357,t2358,t2359,t2361,t2363,t2364,t2366,t2367,t2368,t2369,t2371,t2372,t2373,t2374,t2375,t2376,t2378,t2379,t2380,t2381,t2382,t2384,t2385,t2386,t2387,t2388,t2393,t2395,t2396,t2398,t2399,t24,t2400,t2401,t2402,t2403,t2405,t2406,t2407,t2409,t2411,t2412,t2414,t2415,t2416,t2419,t2421,t2423,t2427,t2428,t2430,t2431,t2433,t2434,t2438,t244,t2445,t2446,t245,t2450,t2453,t2454,t2455,t2457,t2460,t2463,t2467,t247,t2471,t2472,t2473,t2475,t2476,t2477,t2478,t2479,t248,t2484,t2486,t2488,t249,t2490,t2491,t2492,t2493,t2497,t2498,t2499,t25,t2500,t2501,t2502,t2503,t2504,t2506,t2507,t2508,t2509,t2510,t2511,t2512,t2513,t2514,t2517,t2520,t2523,t2526,t2527,t2528,t2529,t2530,t2532,t2533,t2534,t2536,t2544,t2545,t2546,t2549,t255,t2550,t2552,t2557,t2559,t256,t2562,t2563,t2566,t2568,t2569,t2570,t2573,t2574,t2575,t2576,t2578,t2583,t2585,t2586,t2587,t2588,t2589,t2591,t2593,t2595,t2596,t2599,t26,t2602,t2604,t2605,t2606,t2608,t2610,t2614,t2617,t2619,t2620,t2622,t2624,t2625,t2626,t2627,t2630,t2640,t2641,t2642,t2644,t2645,t2646,t2647,t2648,t2651,t2652,t2654,t2655,t2658,t2659,t2661,t2664,t2665,t2666,t2673,t2675,t2677,t2678,t2679,t2680,t2681,t2682,t2686,t2689,t2690,t2691,t2696,t2697,t2699,t27,t2701,t2702,t2703,t2704,t2705,t2707,t2708,t2709,t2710,t2711,t2712,t2718,t2719,t2721,t2722,t2723,t2724,t2725,t2731,t2733,t2734,t2737,t2743,t2744,t2745,t2747,t2749,t2754,t2755,t2759,t2760,t2761,t2762,t2763,t2764,t2765,t2766,t2769,t2772,t2773,t2775,t2776,t2777,t2779,t2780,t2781,t2782,t2789,t279,t2790,t2791,t2792,t2793,t2795,t2796,t2797,t2798,t2800,t2801,t2802,t2806,t2807,t2808,t2810,t2811,t2812,t2813,t2815,t2816,t2817,t2818,t2819,t2820,t2825,t2826,t2828,t2829,t2830,t2832,t2833,t2835,t2837,t2838,t2840,t2841,t2842,t2843,t2845,t2847,t2848,t2851,t2853,t2854,t2855,t2856,t2857,t2859,t2860,t2861,t2862,t2864,t2865,t2867,t2868,t2870,t2871,t2873,t2875,t2876,t2877,t2878,t2879,t2880,t2881,t2882,t2883,t2884,t2885,t2891,t2892,t2893,t2894,t2895,t2897,t2898,t2899,t29,t2900,t2901,t2902,t2910,t2911,t2912,t2913,t2914,t2915,t2917,t2918,t2919,t2925,t2926,t2927,t2929,t2930,t2933,t2934,t2935,t2936,t2937,t2940,t2942,t2944,t2946,t2947,t2948,t2949,t2950,t2951,t2953,t2954,t2956,t2957,t2959,t2961,t2966,t2967,t2968,t2970,t2971,t2972,t2974,t2975,t2978,t2979,t2981,t2982,t2983,t2985,t2988,t2989,t299,t2991,t2992,t2994,t2995,t2996,t2997,t2998,t2999,t2d,t2dd,t30,t3000,t3003,t3004,t3005,t3006,t3007,t3009,t301,t3010,t3011,t3012,t3013,t3014,t3017,t3018,t3019,t3025,t3028,t3029,t3032,t3035,t3037,t3043,t3044,t3047,t3048,t3049,t3050,t3052,t3055,t3057,t3058,t3059,t3065,t3066,t3069,t3073,t3074,t3075,t3076,t3078,t3079,t308,t3080,t3081,t3082,t3083,t3085,t3086,t3087,t3088,t3089,t3090,t3091,t3092,t3093,t3096,t3098,t3099,t31,t3100,t3101,t3104,t3106,t3107,t3108,t3112,t3113,t3115,t3120,t3121,t3123,t3124,t3125,t3126,t3129,t3130,t3135,t3136,t3137,t3138,t3139,t3140,t3141,t3142,t3143,t3146,t315,t3150,t3151,t3153,t3155,t3156,t3157,t3158,t3159,t3161,t3162,t3163,t3165,t3166,t3168,t3169,t317,t3170,t3171,t3172,t3173,t3174,t3175,t3176,t3177,t3179,t318,t3180,t3182,t3183,t3185,t3187,t319,t3192,t3194,t3195,t3196,t3197,t3204,t3214,t3220,t3230,t3231,t3232,t3234,t3236,t3237,t3240,t3244,t3246,t325,t3251,t3253,t3258,t3260,t3267,t3268,t3272,t3275,t3278,t3283,t3285,t3288,t3289,t329,t3291,t3292,t3298,t330,t3302,t3305,t3306,t3308,t3313,t3318,t3319,t332,t3321,t3322,t3323,t3326,t333,t3330,t3331,t3332,t3335,t3339,t3340,t3348,t3349,t3351,t3354,t3355,t3358,t3359,t3360,t3367,t3377,t3378,t3380,t3381,t3383,t3384,t3387,t3388,t3390,t3391,t3399,t34,t3400,t3401,t3403,t3404,t3405,t341,t3414,t3415,t3416,t3417,t342,t3421,t3429,t343,t3431,t3432,t3439,t344,t3440,t3445,t3451,t3452,t3453,t3454,t3455,t3456,t3457,t3458,t3459,t346,t3460,t3461,t3463,t3468,t3469,t347,t3472,t3473,t3474,t3475,t3477,t3478,t3479,t3480,t3481,t3483,t3488,t3490,t3493,t3495,t3499,t35,t3502,t3503,t3504,t3506,t3508,t3509,t3510,t3515,t3516,t3517,t3518,t3521,t3523,t3527,t3532,t3534,t3536,t3537,t3538,t3539,t354,t3540,t3543,t3544,t3547,t3549,t3551,t3555,t3556,t3557,t3558,t3559,t3563,t3565,t3568,t3569,t3571,t3573,t3574,t3575,t3577,t3578,t3579,t3580,t3582,t3586,t3587,t3588,t3589,t3590,t3591,t3598,t36,t3600,t3601,t3602,t3603,t3604,t3606,t3607,t3609,t3610,t3611,t3613,t3615,t3617,t3620,t3622,t3623,t3624,t3625,t3626,t3627,t3628,t3630,t3634,t3635,t3637,t3639,t364,t3649,t365,t3650,t3651,t3668,t3670,t3675,t368,t3682,t3683,t3684,t3685,t3686,t3687,t3690,t3697,t37,t3701,t3712,t3716,t3722,t3732,t3733,t3734,t3739,t3741,t3744,t3745,t3747,t3750,t3751,t3753,t3754,t3755,t3756,t3757,t3762,t3763,t3764,t3766,t3768,t3770,t3771,t3780,t3781,t3783,t3784,t3785,t3787,t3789,t3792,t38,t3800,t3804,t3809,t3810,t3811,t3812,t3817,t3821,t3822,t3826,t3828,t3830,t3832,t3833,t3838,t384,t3840,t3843,t3848,t3858,t3860,t3861,t3863,t3866,t3867,t3871,t3872,t3874,t3875,t3880,t3886,t3887,t3888,t3889,t3890,t3892,t3894,t3896,t3897,t39,t3900,t3903,t3917,t3919,t392,t3923,t3927,t393,t3931,t3932,t3933,t3936,t3937,t3943,t3950,t3956,t3958,t3959,t3962,t3963,t3965,t3967,t3972,t3976,t3978,t3982,t3983,t3989,t3990,t3993,t3994,t3997,t3d,t3dd,t4001,t4002,t4003,t4005,t4006,t4007,t401,t4012,t4014,t4017,t4018,t4019,t402,t4023,t4025,t4026,t4027,t403,t4030,t4038,t404,t4041,t4042,t4045,t4046,t4047,t4048,t4049,t4050,t4053,t4059,t4066,t4067,t4068,t4069,t4071,t4073,t4074,t4078,t4081,t4084,t4086,t4087,t4090,t4091,t4095,t4096,t4097,t41,t4101,t4102,t4112,t4113,t4115,t4117,t4118,t4121,t4122,t4125,t4126,t4128,t4130,t4131,t4133,t4134,t4136,t4137,t4139,t4140,t4142,t4143,t4144,t4145,t4146,t4147,t4148,t4149,t4151,t4152,t4155,t4156,t4157,t4158,t4159,t4160,t4162,t4164,t4166,t4167,t4168,t4170,t4171,t4172,t4174,t4176,t4178,t418,t4180,t4182,t4183,t4185,t4186,t4187,t4188,t4189,t419,t4192,t4193,t4194,t4195,t4196,t42,t420,t4202,t4203,t4204,t4208,t4212,t4215,t4217,t4220,t4221,t4222,t4225,t4226,t4230,t4231,t4233,t4236,t4237,t425,t4251,t4252,t4255,t4256,t4267,t4283,t4290,t4294,t4296,t4299,t4302,t4304,t4309,t431,t4321,t4324,t4325,t4327,t4330,t4331,t4332,t4333,t4334,t4335,t4337,t434,t4348,t4351,t4353,t4361,t4367,t437,t4371,t4393,t4394,t4395,t4399,t4402,t4403,t4404,t4406,t4408,t441,t4410,t4413,t442,t4421,t4424,t4428,t4429,t443,t4430,t4431,t4444,t4450,t4451,t4454,t4457,t4459,t446,t4460,t4461,t4467,t4468,t4470,t4475,t4479,t4480,t4483,t4486,t4487,t4491,t4493,t4494,t4499,t4500,t4503,t4508,t4512,t4513,t4526,t4528,t4529,t453,t4531,t4533,t4534,t4538,t4539,t454,t4540,t4541,t4542,t4547,t4548,t4549,t4551,t4553,t4556,t4561,t4563,t4566,t4579,t4582,t459,t4591,t4592,t4595,t4596,t4599,t4604,t4607,t4608,t4615,t4620,t4623,t4626,t4627,t4629,t4632,t4633,t4642,t4647,t4648,t4655,t4664,t4665,t4666,t4668,t4670,t4672,t4673,t4675,t4676,t4677,t4678,t4681,t4683,t4688,t4694,t4695,t4699,t470,t4703,t4704,t4705,t4707,t4708,t4714,t4715,t4716,t4720,t4722,t4727,t4747,t4757,t4759,t4765,t4771,t4776,t478,t4785,t4786,t4792,t4795,t4798,t4799,t48,t4801,t4802,t4813,t4815,t4817,t483,t4831,t4836,t4837,t4838,t484,t4840,t4845,t4846,t4855,t4856,t4858,t4859,t486,t4861,t4862,t4865,t4867,t487,t4870,t4871,t4874,t4878,t488,t4881,t4883,t4887,t4889,t4891,t4896,t4908,t4909,t4917,t492,t4920,t4922,t4923,t4924,t4926,t4929,t493,t4930,t4931,t4932,t4935,t494,t4941,t4944,t4946,t4949,t495,t4950,t4951,t4952,t4955,t4956,t4957,t4958,t4959,t496,t4967,t497,t4979,t498,t4981,t4985,t4990,t4992,t4993,t4997,t4d,t4dd,t50,t5001,t5006,t501,t5010,t5011,t5012,t5013,t5018,t5019,t5020,t5026,t503,t5036,t5038,t5040,t5041,t5043,t5047,t5051,t5056,t5070,t5074,t508,t5081,t5091,t5092,t5093,t5098,t51,t5104,t5116,t5117,t5119,t5123,t5131,t5136,t514,t5141,t515,t516,t5163,t5171,t5175,t5176,t519,t5219,t5223,t523,t524,t5255,t5258,t5278,t5281,t5283,t529,t5292,t53,t530,t532,t5351,t537,t5401,t5403,t543,t544,t546,t5465,t547,t5476,t548,t549,t55,t5501,t5513,t5516,t552,t553,t554,t56,t562,t569,t57,t570,t58,t582,t588,t589,t591,t593,t598,t5d,t5dd,t601,t602,t604,t608,t609,t61,t612,t614,t615,t616,t617,t623,t627,t63,t632,t633,t634,t635,t636,t637,t639,t641,t645,t646,t647,t648,t649,t650,t652,t653,t655,t659,t664,t667,t670,t671,t675,t680,t681,t682,t687,t69,t690,t691,t694,t695,t696,t698,t699,t6d,t6dd,t702,t703,t705,t706,t71,t711,t712,t713,t714,t720,t721,t723,t725,t726,t729,t731,t732,t733,t735,t736,t738,t739,t745,t746,t747,t748,t75,t752,t755,t759,t760,t761,t763,t764,t775,t776,t781,t785,t788,t789,t793,t8,t802,t806,t82,t820,t824,t828,t831,t832,t833,t838,t842,t843,t844,t846,t848,t849,t850,t851,t852,t853,t854,t855,t859,t861,t865,t870,t871,t873,t879,t880,t884,t885,t890,t892,t896,t897,t898,t899,t9,t900,t907,t909,t910,t915,t917,t919,t922,t923,t927,t928,t930,t932,t937,t943,t944,t945,t949,t952,t959,t961,t962,t963,t964,t965,t966,t967,t969,t970,t972,t973,t978,t979,t981,t982,t983,t986,t987,t989,t992,t999});
end
function Y = ft_8(ct)
t100 = ct{1};
t1004 = ct{2};
t1007 = ct{3};
t1009 = ct{4};
t101 = ct{5};
t1015 = ct{6};
t1016 = ct{7};
t1017 = ct{8};
t1019 = ct{9};
t1021 = ct{10};
t1026 = ct{11};
t1028 = ct{12};
t1031 = ct{13};
t1035 = ct{14};
t1036 = ct{15};
t104 = ct{16};
t1044 = ct{17};
t1045 = ct{18};
t1046 = ct{19};
t1047 = ct{20};
t1048 = ct{21};
t1049 = ct{22};
t1053 = ct{23};
t1054 = ct{24};
t1055 = ct{25};
t106 = ct{26};
t1064 = ct{27};
t1066 = ct{28};
t1068 = ct{29};
t1069 = ct{30};
t107 = ct{31};
t1070 = ct{32};
t1071 = ct{33};
t1079 = ct{34};
t108 = ct{35};
t1080 = ct{36};
t1081 = ct{37};
t1082 = ct{38};
t1083 = ct{39};
t1084 = ct{40};
t1085 = ct{41};
t1086 = ct{42};
t1087 = ct{43};
t1093 = ct{44};
t1094 = ct{45};
t1096 = ct{46};
t1097 = ct{47};
t1098 = ct{48};
t1099 = ct{49};
t1101 = ct{50};
t1106 = ct{51};
t1108 = ct{52};
t1109 = ct{53};
t111 = ct{54};
t1110 = ct{55};
t112 = ct{56};
t1121 = ct{57};
t1122 = ct{58};
t1123 = ct{59};
t1125 = ct{60};
t1126 = ct{61};
t1128 = ct{62};
t1129 = ct{63};
t113 = ct{64};
t1133 = ct{65};
t1134 = ct{66};
t1135 = ct{67};
t1137 = ct{68};
t1138 = ct{69};
t1139 = ct{70};
t1140 = ct{71};
t1143 = ct{72};
t1147 = ct{73};
t1148 = ct{74};
t1152 = ct{75};
t1155 = ct{76};
t1156 = ct{77};
t1158 = ct{78};
t1160 = ct{79};
t1162 = ct{80};
t1171 = ct{81};
t1172 = ct{82};
t1174 = ct{83};
t1181 = ct{84};
t1182 = ct{85};
t1183 = ct{86};
t1184 = ct{87};
t1185 = ct{88};
t1186 = ct{89};
t1187 = ct{90};
t1189 = ct{91};
t1191 = ct{92};
t1193 = ct{93};
t1196 = ct{94};
t12 = ct{95};
t1203 = ct{96};
t1207 = ct{97};
t1208 = ct{98};
t1209 = ct{99};
t1210 = ct{100};
t1211 = ct{101};
t1222 = ct{102};
t1224 = ct{103};
t1225 = ct{104};
t1226 = ct{105};
t1227 = ct{106};
t1229 = ct{107};
t1230 = ct{108};
t1235 = ct{109};
t1236 = ct{110};
t1237 = ct{111};
t1238 = ct{112};
t124 = ct{113};
t1245 = ct{114};
t1246 = ct{115};
t1247 = ct{116};
t1248 = ct{117};
t1249 = ct{118};
t1250 = ct{119};
t1251 = ct{120};
t1252 = ct{121};
t1255 = ct{122};
t1264 = ct{123};
t1265 = ct{124};
t1266 = ct{125};
t1268 = ct{126};
t127 = ct{127};
t1271 = ct{128};
t1272 = ct{129};
t1273 = ct{130};
t128 = ct{131};
t1281 = ct{132};
t1282 = ct{133};
t1284 = ct{134};
t1285 = ct{135};
t1286 = ct{136};
t1287 = ct{137};
t1288 = ct{138};
t1289 = ct{139};
t1292 = ct{140};
t1297 = ct{141};
t1298 = ct{142};
t13 = ct{143};
t1302 = ct{144};
t1306 = ct{145};
t131 = ct{146};
t1311 = ct{147};
t1312 = ct{148};
t1316 = ct{149};
t1317 = ct{150};
t132 = ct{151};
t1321 = ct{152};
t1328 = ct{153};
t1331 = ct{154};
t1332 = ct{155};
t1333 = ct{156};
t1334 = ct{157};
t1335 = ct{158};
t1336 = ct{159};
t1337 = ct{160};
t134 = ct{161};
t1341 = ct{162};
t1346 = ct{163};
t1347 = ct{164};
t1348 = ct{165};
t1350 = ct{166};
t1353 = ct{167};
t1355 = ct{168};
t1356 = ct{169};
t1357 = ct{170};
t1358 = ct{171};
t1359 = ct{172};
t136 = ct{173};
t1361 = ct{174};
t1366 = ct{175};
t1367 = ct{176};
t1368 = ct{177};
t1369 = ct{178};
t137 = ct{179};
t1375 = ct{180};
t1378 = ct{181};
t1379 = ct{182};
t138 = ct{183};
t1382 = ct{184};
t1387 = ct{185};
t1388 = ct{186};
t1391 = ct{187};
t1392 = ct{188};
t1393 = ct{189};
t1395 = ct{190};
t1397 = ct{191};
t1398 = ct{192};
t1399 = ct{193};
t14 = ct{194};
t1400 = ct{195};
t1403 = ct{196};
t1406 = ct{197};
t1408 = ct{198};
t1410 = ct{199};
t1412 = ct{200};
t1413 = ct{201};
t1418 = ct{202};
t1419 = ct{203};
t1420 = ct{204};
t1423 = ct{205};
t1425 = ct{206};
t1427 = ct{207};
t1428 = ct{208};
t1430 = ct{209};
t1434 = ct{210};
t1435 = ct{211};
t1438 = ct{212};
t1440 = ct{213};
t1451 = ct{214};
t1457 = ct{215};
t1458 = ct{216};
t1461 = ct{217};
t1464 = ct{218};
t1465 = ct{219};
t1468 = ct{220};
t1470 = ct{221};
t1472 = ct{222};
t1473 = ct{223};
t1475 = ct{224};
t1476 = ct{225};
t1477 = ct{226};
t1478 = ct{227};
t1479 = ct{228};
t1480 = ct{229};
t1483 = ct{230};
t1484 = ct{231};
t1485 = ct{232};
t1486 = ct{233};
t1489 = ct{234};
t1491 = ct{235};
t1492 = ct{236};
t1493 = ct{237};
t1496 = ct{238};
t1497 = ct{239};
t1499 = ct{240};
t15 = ct{241};
t150 = ct{242};
t1500 = ct{243};
t1501 = ct{244};
t1503 = ct{245};
t1504 = ct{246};
t1507 = ct{247};
t1513 = ct{248};
t1514 = ct{249};
t1516 = ct{250};
t1517 = ct{251};
t1518 = ct{252};
t1519 = ct{253};
t152 = ct{254};
t1520 = ct{255};
t1521 = ct{256};
t1524 = ct{257};
t1525 = ct{258};
t1527 = ct{259};
t1528 = ct{260};
t1529 = ct{261};
t1531 = ct{262};
t1532 = ct{263};
t1534 = ct{264};
t1535 = ct{265};
t1536 = ct{266};
t1537 = ct{267};
t1538 = ct{268};
t1547 = ct{269};
t1549 = ct{270};
t155 = ct{271};
t1553 = ct{272};
t156 = ct{273};
t1569 = ct{274};
t1571 = ct{275};
t1572 = ct{276};
t1574 = ct{277};
t1577 = ct{278};
t1578 = ct{279};
t1579 = ct{280};
t158 = ct{281};
t1580 = ct{282};
t1583 = ct{283};
t1585 = ct{284};
t1586 = ct{285};
t1588 = ct{286};
t1589 = ct{287};
t159 = ct{288};
t1590 = ct{289};
t1591 = ct{290};
t1594 = ct{291};
t1597 = ct{292};
t1599 = ct{293};
t1606 = ct{294};
t1607 = ct{295};
t1609 = ct{296};
t1610 = ct{297};
t1611 = ct{298};
t1613 = ct{299};
t1614 = ct{300};
t1615 = ct{301};
t1616 = ct{302};
t1617 = ct{303};
t1618 = ct{304};
t1619 = ct{305};
t162 = ct{306};
t1620 = ct{307};
t1621 = ct{308};
t1622 = ct{309};
t1625 = ct{310};
t1627 = ct{311};
t1628 = ct{312};
t163 = ct{313};
t1630 = ct{314};
t1631 = ct{315};
t1632 = ct{316};
t1634 = ct{317};
t1635 = ct{318};
t1636 = ct{319};
t1638 = ct{320};
t164 = ct{321};
t1642 = ct{322};
t1643 = ct{323};
t1645 = ct{324};
t1647 = ct{325};
t1648 = ct{326};
t1649 = ct{327};
t165 = ct{328};
t1650 = ct{329};
t1651 = ct{330};
t1652 = ct{331};
t1653 = ct{332};
t1654 = ct{333};
t1659 = ct{334};
t1660 = ct{335};
t1663 = ct{336};
t1664 = ct{337};
t1665 = ct{338};
t1667 = ct{339};
t1670 = ct{340};
t1671 = ct{341};
t1672 = ct{342};
t1674 = ct{343};
t1675 = ct{344};
t1677 = ct{345};
t1678 = ct{346};
t1680 = ct{347};
t1681 = ct{348};
t1682 = ct{349};
t1683 = ct{350};
t1685 = ct{351};
t1686 = ct{352};
t1687 = ct{353};
t1688 = ct{354};
t1691 = ct{355};
t1692 = ct{356};
t1698 = ct{357};
t1699 = ct{358};
t1701 = ct{359};
t1704 = ct{360};
t1706 = ct{361};
t1707 = ct{362};
t1709 = ct{363};
t171 = ct{364};
t1710 = ct{365};
t1713 = ct{366};
t1714 = ct{367};
t1715 = ct{368};
t1717 = ct{369};
t1719 = ct{370};
t1722 = ct{371};
t1724 = ct{372};
t173 = ct{373};
t1733 = ct{374};
t1736 = ct{375};
t1738 = ct{376};
t174 = ct{377};
t1740 = ct{378};
t1741 = ct{379};
t1742 = ct{380};
t1743 = ct{381};
t1746 = ct{382};
t1747 = ct{383};
t1748 = ct{384};
t175 = ct{385};
t1751 = ct{386};
t1754 = ct{387};
t1755 = ct{388};
t1758 = ct{389};
t1759 = ct{390};
t1760 = ct{391};
t1763 = ct{392};
t1766 = ct{393};
t1767 = ct{394};
t177 = ct{395};
t1776 = ct{396};
t1780 = ct{397};
t1782 = ct{398};
t1783 = ct{399};
t1784 = ct{400};
t1786 = ct{401};
t1787 = ct{402};
t1789 = ct{403};
t1790 = ct{404};
t1792 = ct{405};
t1796 = ct{406};
t1797 = ct{407};
t1799 = ct{408};
t18 = ct{409};
t1800 = ct{410};
t1803 = ct{411};
t1807 = ct{412};
t1813 = ct{413};
t1814 = ct{414};
t1815 = ct{415};
t1816 = ct{416};
t1818 = ct{417};
t1824 = ct{418};
t1826 = ct{419};
t1827 = ct{420};
t1829 = ct{421};
t1830 = ct{422};
t1832 = ct{423};
t1833 = ct{424};
t1835 = ct{425};
t1836 = ct{426};
t1837 = ct{427};
t1838 = ct{428};
t1840 = ct{429};
t1841 = ct{430};
t1842 = ct{431};
t1844 = ct{432};
t1846 = ct{433};
t1848 = ct{434};
t1849 = ct{435};
t1850 = ct{436};
t1851 = ct{437};
t1854 = ct{438};
t1860 = ct{439};
t1862 = ct{440};
t1863 = ct{441};
t1864 = ct{442};
t1866 = ct{443};
t1867 = ct{444};
t1868 = ct{445};
t1869 = ct{446};
t187 = ct{447};
t1873 = ct{448};
t1874 = ct{449};
t1875 = ct{450};
t1876 = ct{451};
t1877 = ct{452};
t1878 = ct{453};
t1879 = ct{454};
t1888 = ct{455};
t1889 = ct{456};
t1890 = ct{457};
t1891 = ct{458};
t1892 = ct{459};
t1893 = ct{460};
t1899 = ct{461};
t19 = ct{462};
t1900 = ct{463};
t1901 = ct{464};
t1902 = ct{465};
t1903 = ct{466};
t1904 = ct{467};
t1905 = ct{468};
t191 = ct{469};
t1911 = ct{470};
t1912 = ct{471};
t1913 = ct{472};
t1915 = ct{473};
t1916 = ct{474};
t1918 = ct{475};
t1919 = ct{476};
t1920 = ct{477};
t1921 = ct{478};
t1923 = ct{479};
t1925 = ct{480};
t1926 = ct{481};
t1927 = ct{482};
t1929 = ct{483};
t1930 = ct{484};
t1933 = ct{485};
t1934 = ct{486};
t1935 = ct{487};
t1936 = ct{488};
t1938 = ct{489};
t1939 = ct{490};
t1940 = ct{491};
t1941 = ct{492};
t1944 = ct{493};
t1945 = ct{494};
t1948 = ct{495};
t1949 = ct{496};
t1951 = ct{497};
t1952 = ct{498};
t1956 = ct{499};
t1957 = ct{500};
t1958 = ct{501};
t1959 = ct{502};
t1960 = ct{503};
t1961 = ct{504};
t1962 = ct{505};
t1963 = ct{506};
t1964 = ct{507};
t1965 = ct{508};
t1966 = ct{509};
t1967 = ct{510};
t1968 = ct{511};
t1969 = ct{512};
t1970 = ct{513};
t1971 = ct{514};
t1972 = ct{515};
t1973 = ct{516};
t1975 = ct{517};
t1976 = ct{518};
t1977 = ct{519};
t1978 = ct{520};
t1979 = ct{521};
t1981 = ct{522};
t1983 = ct{523};
t1984 = ct{524};
t1985 = ct{525};
t1988 = ct{526};
t199 = ct{527};
t1990 = ct{528};
t1992 = ct{529};
t1993 = ct{530};
t1995 = ct{531};
t1996 = ct{532};
t1999 = ct{533};
t1d = ct{534};
t1dd = ct{535};
t200 = ct{536};
t2000 = ct{537};
t2001 = ct{538};
t2002 = ct{539};
t2004 = ct{540};
t2005 = ct{541};
t2009 = ct{542};
t201 = ct{543};
t2010 = ct{544};
t2012 = ct{545};
t2013 = ct{546};
t2015 = ct{547};
t2016 = ct{548};
t2018 = ct{549};
t202 = ct{550};
t2021 = ct{551};
t2022 = ct{552};
t2023 = ct{553};
t2024 = ct{554};
t2026 = ct{555};
t2028 = ct{556};
t2031 = ct{557};
t2033 = ct{558};
t2036 = ct{559};
t2042 = ct{560};
t2044 = ct{561};
t2053 = ct{562};
t2054 = ct{563};
t2059 = ct{564};
t206 = ct{565};
t2060 = ct{566};
t2061 = ct{567};
t2062 = ct{568};
t2065 = ct{569};
t2068 = ct{570};
t2069 = ct{571};
t2070 = ct{572};
t2072 = ct{573};
t2074 = ct{574};
t2075 = ct{575};
t2079 = ct{576};
t2080 = ct{577};
t2081 = ct{578};
t2085 = ct{579};
t2086 = ct{580};
t2087 = ct{581};
t2088 = ct{582};
t2090 = ct{583};
t2093 = ct{584};
t2098 = ct{585};
t2099 = ct{586};
t21 = ct{587};
t2100 = ct{588};
t2101 = ct{589};
t2104 = ct{590};
t2105 = ct{591};
t2107 = ct{592};
t2108 = ct{593};
t2112 = ct{594};
t2113 = ct{595};
t2115 = ct{596};
t2117 = ct{597};
t2119 = ct{598};
t2122 = ct{599};
t2123 = ct{600};
t2124 = ct{601};
t2126 = ct{602};
t2128 = ct{603};
t2129 = ct{604};
t2130 = ct{605};
t2132 = ct{606};
t2136 = ct{607};
t2140 = ct{608};
t2141 = ct{609};
t2142 = ct{610};
t2143 = ct{611};
t2144 = ct{612};
t2145 = ct{613};
t2146 = ct{614};
t2147 = ct{615};
t215 = ct{616};
t2150 = ct{617};
t2153 = ct{618};
t2155 = ct{619};
t2156 = ct{620};
t2159 = ct{621};
t2160 = ct{622};
t2162 = ct{623};
t2167 = ct{624};
t2168 = ct{625};
t2169 = ct{626};
t2170 = ct{627};
t2171 = ct{628};
t2173 = ct{629};
t2174 = ct{630};
t2176 = ct{631};
t2178 = ct{632};
t2180 = ct{633};
t2181 = ct{634};
t2182 = ct{635};
t2184 = ct{636};
t2186 = ct{637};
t2187 = ct{638};
t2188 = ct{639};
t2189 = ct{640};
t219 = ct{641};
t2190 = ct{642};
t2191 = ct{643};
t2193 = ct{644};
t2194 = ct{645};
t2196 = ct{646};
t2198 = ct{647};
t22 = ct{648};
t220 = ct{649};
t2204 = ct{650};
t2206 = ct{651};
t221 = ct{652};
t2210 = ct{653};
t2213 = ct{654};
t2216 = ct{655};
t2219 = ct{656};
t2220 = ct{657};
t2222 = ct{658};
t2223 = ct{659};
t2224 = ct{660};
t2225 = ct{661};
t2229 = ct{662};
t2230 = ct{663};
t2233 = ct{664};
t2235 = ct{665};
t2242 = ct{666};
t2243 = ct{667};
t2244 = ct{668};
t2246 = ct{669};
t2247 = ct{670};
t2249 = ct{671};
t2259 = ct{672};
t226 = ct{673};
t2266 = ct{674};
t2267 = ct{675};
t2269 = ct{676};
t2270 = ct{677};
t2278 = ct{678};
t2279 = ct{679};
t2281 = ct{680};
t2282 = ct{681};
t2283 = ct{682};
t2284 = ct{683};
t2286 = ct{684};
t2289 = ct{685};
t229 = ct{686};
t2290 = ct{687};
t2292 = ct{688};
t2293 = ct{689};
t2294 = ct{690};
t2295 = ct{691};
t2296 = ct{692};
t23 = ct{693};
t2300 = ct{694};
t2304 = ct{695};
t2305 = ct{696};
t2306 = ct{697};
t2307 = ct{698};
t2308 = ct{699};
t2310 = ct{700};
t2311 = ct{701};
t2314 = ct{702};
t2317 = ct{703};
t2319 = ct{704};
t232 = ct{705};
t2320 = ct{706};
t2321 = ct{707};
t2322 = ct{708};
t2325 = ct{709};
t2326 = ct{710};
t2327 = ct{711};
t2328 = ct{712};
t2329 = ct{713};
t233 = ct{714};
t2330 = ct{715};
t2331 = ct{716};
t2332 = ct{717};
t2339 = ct{718};
t2340 = ct{719};
t2344 = ct{720};
t2346 = ct{721};
t2348 = ct{722};
t2349 = ct{723};
t2351 = ct{724};
t2352 = ct{725};
t2353 = ct{726};
t2354 = ct{727};
t2355 = ct{728};
t2356 = ct{729};
t2357 = ct{730};
t2358 = ct{731};
t2359 = ct{732};
t2361 = ct{733};
t2363 = ct{734};
t2364 = ct{735};
t2366 = ct{736};
t2367 = ct{737};
t2368 = ct{738};
t2369 = ct{739};
t2371 = ct{740};
t2372 = ct{741};
t2373 = ct{742};
t2374 = ct{743};
t2375 = ct{744};
t2376 = ct{745};
t2378 = ct{746};
t2379 = ct{747};
t2380 = ct{748};
t2381 = ct{749};
t2382 = ct{750};
t2384 = ct{751};
t2385 = ct{752};
t2386 = ct{753};
t2387 = ct{754};
t2388 = ct{755};
t2393 = ct{756};
t2395 = ct{757};
t2396 = ct{758};
t2398 = ct{759};
t2399 = ct{760};
t24 = ct{761};
t2400 = ct{762};
t2401 = ct{763};
t2402 = ct{764};
t2403 = ct{765};
t2405 = ct{766};
t2406 = ct{767};
t2407 = ct{768};
t2409 = ct{769};
t2411 = ct{770};
t2412 = ct{771};
t2414 = ct{772};
t2415 = ct{773};
t2416 = ct{774};
t2419 = ct{775};
t2421 = ct{776};
t2423 = ct{777};
t2427 = ct{778};
t2428 = ct{779};
t2430 = ct{780};
t2431 = ct{781};
t2433 = ct{782};
t2434 = ct{783};
t2438 = ct{784};
t244 = ct{785};
t2445 = ct{786};
t2446 = ct{787};
t245 = ct{788};
t2450 = ct{789};
t2453 = ct{790};
t2454 = ct{791};
t2455 = ct{792};
t2457 = ct{793};
t2460 = ct{794};
t2463 = ct{795};
t2467 = ct{796};
t247 = ct{797};
t2471 = ct{798};
t2472 = ct{799};
t2473 = ct{800};
t2475 = ct{801};
t2476 = ct{802};
t2477 = ct{803};
t2478 = ct{804};
t2479 = ct{805};
t248 = ct{806};
t2484 = ct{807};
t2486 = ct{808};
t2488 = ct{809};
t249 = ct{810};
t2490 = ct{811};
t2491 = ct{812};
t2492 = ct{813};
t2493 = ct{814};
t2497 = ct{815};
t2498 = ct{816};
t2499 = ct{817};
t25 = ct{818};
t2500 = ct{819};
t2501 = ct{820};
t2502 = ct{821};
t2503 = ct{822};
t2504 = ct{823};
t2506 = ct{824};
t2507 = ct{825};
t2508 = ct{826};
t2509 = ct{827};
t2510 = ct{828};
t2511 = ct{829};
t2512 = ct{830};
t2513 = ct{831};
t2514 = ct{832};
t2517 = ct{833};
t2520 = ct{834};
t2523 = ct{835};
t2526 = ct{836};
t2527 = ct{837};
t2528 = ct{838};
t2529 = ct{839};
t2530 = ct{840};
t2532 = ct{841};
t2533 = ct{842};
t2534 = ct{843};
t2536 = ct{844};
t2544 = ct{845};
t2545 = ct{846};
t2546 = ct{847};
t2549 = ct{848};
t255 = ct{849};
t2550 = ct{850};
t2552 = ct{851};
t2557 = ct{852};
t2559 = ct{853};
t256 = ct{854};
t2562 = ct{855};
t2563 = ct{856};
t2566 = ct{857};
t2568 = ct{858};
t2569 = ct{859};
t2570 = ct{860};
t2573 = ct{861};
t2574 = ct{862};
t2575 = ct{863};
t2576 = ct{864};
t2578 = ct{865};
t2583 = ct{866};
t2585 = ct{867};
t2586 = ct{868};
t2587 = ct{869};
t2588 = ct{870};
t2589 = ct{871};
t2591 = ct{872};
t2593 = ct{873};
t2595 = ct{874};
t2596 = ct{875};
t2599 = ct{876};
t26 = ct{877};
t2602 = ct{878};
t2604 = ct{879};
t2605 = ct{880};
t2606 = ct{881};
t2608 = ct{882};
t2610 = ct{883};
t2614 = ct{884};
t2617 = ct{885};
t2619 = ct{886};
t2620 = ct{887};
t2622 = ct{888};
t2624 = ct{889};
t2625 = ct{890};
t2626 = ct{891};
t2627 = ct{892};
t2630 = ct{893};
t2640 = ct{894};
t2641 = ct{895};
t2642 = ct{896};
t2644 = ct{897};
t2645 = ct{898};
t2646 = ct{899};
t2647 = ct{900};
t2648 = ct{901};
t2651 = ct{902};
t2652 = ct{903};
t2654 = ct{904};
t2655 = ct{905};
t2658 = ct{906};
t2659 = ct{907};
t2661 = ct{908};
t2664 = ct{909};
t2665 = ct{910};
t2666 = ct{911};
t2673 = ct{912};
t2675 = ct{913};
t2677 = ct{914};
t2678 = ct{915};
t2679 = ct{916};
t2680 = ct{917};
t2681 = ct{918};
t2682 = ct{919};
t2686 = ct{920};
t2689 = ct{921};
t2690 = ct{922};
t2691 = ct{923};
t2696 = ct{924};
t2697 = ct{925};
t2699 = ct{926};
t27 = ct{927};
t2701 = ct{928};
t2702 = ct{929};
t2703 = ct{930};
t2704 = ct{931};
t2705 = ct{932};
t2707 = ct{933};
t2708 = ct{934};
t2709 = ct{935};
t2710 = ct{936};
t2711 = ct{937};
t2712 = ct{938};
t2718 = ct{939};
t2719 = ct{940};
t2721 = ct{941};
t2722 = ct{942};
t2723 = ct{943};
t2724 = ct{944};
t2725 = ct{945};
t2731 = ct{946};
t2733 = ct{947};
t2734 = ct{948};
t2737 = ct{949};
t2743 = ct{950};
t2744 = ct{951};
t2745 = ct{952};
t2747 = ct{953};
t2749 = ct{954};
t2754 = ct{955};
t2755 = ct{956};
t2759 = ct{957};
t2760 = ct{958};
t2761 = ct{959};
t2762 = ct{960};
t2763 = ct{961};
t2764 = ct{962};
t2765 = ct{963};
t2766 = ct{964};
t2769 = ct{965};
t2772 = ct{966};
t2773 = ct{967};
t2775 = ct{968};
t2776 = ct{969};
t2777 = ct{970};
t2779 = ct{971};
t2780 = ct{972};
t2781 = ct{973};
t2782 = ct{974};
t2789 = ct{975};
t279 = ct{976};
t2790 = ct{977};
t2791 = ct{978};
t2792 = ct{979};
t2793 = ct{980};
t2795 = ct{981};
t2796 = ct{982};
t2797 = ct{983};
t2798 = ct{984};
t2800 = ct{985};
t2801 = ct{986};
t2802 = ct{987};
t2806 = ct{988};
t2807 = ct{989};
t2808 = ct{990};
t2810 = ct{991};
t2811 = ct{992};
t2812 = ct{993};
t2813 = ct{994};
t2815 = ct{995};
t2816 = ct{996};
t2817 = ct{997};
t2818 = ct{998};
t2819 = ct{999};
t2820 = ct{1000};
t2825 = ct{1001};
t2826 = ct{1002};
t2828 = ct{1003};
t2829 = ct{1004};
t2830 = ct{1005};
t2832 = ct{1006};
t2833 = ct{1007};
t2835 = ct{1008};
t2837 = ct{1009};
t2838 = ct{1010};
t2840 = ct{1011};
t2841 = ct{1012};
t2842 = ct{1013};
t2843 = ct{1014};
t2845 = ct{1015};
t2847 = ct{1016};
t2848 = ct{1017};
t2851 = ct{1018};
t2853 = ct{1019};
t2854 = ct{1020};
t2855 = ct{1021};
t2856 = ct{1022};
t2857 = ct{1023};
t2859 = ct{1024};
t2860 = ct{1025};
t2861 = ct{1026};
t2862 = ct{1027};
t2864 = ct{1028};
t2865 = ct{1029};
t2867 = ct{1030};
t2868 = ct{1031};
t2870 = ct{1032};
t2871 = ct{1033};
t2873 = ct{1034};
t2875 = ct{1035};
t2876 = ct{1036};
t2877 = ct{1037};
t2878 = ct{1038};
t2879 = ct{1039};
t2880 = ct{1040};
t2881 = ct{1041};
t2882 = ct{1042};
t2883 = ct{1043};
t2884 = ct{1044};
t2885 = ct{1045};
t2891 = ct{1046};
t2892 = ct{1047};
t2893 = ct{1048};
t2894 = ct{1049};
t2895 = ct{1050};
t2897 = ct{1051};
t2898 = ct{1052};
t2899 = ct{1053};
t29 = ct{1054};
t2900 = ct{1055};
t2901 = ct{1056};
t2902 = ct{1057};
t2910 = ct{1058};
t2911 = ct{1059};
t2912 = ct{1060};
t2913 = ct{1061};
t2914 = ct{1062};
t2915 = ct{1063};
t2917 = ct{1064};
t2918 = ct{1065};
t2919 = ct{1066};
t2925 = ct{1067};
t2926 = ct{1068};
t2927 = ct{1069};
t2929 = ct{1070};
t2930 = ct{1071};
t2933 = ct{1072};
t2934 = ct{1073};
t2935 = ct{1074};
t2936 = ct{1075};
t2937 = ct{1076};
t2940 = ct{1077};
t2942 = ct{1078};
t2944 = ct{1079};
t2946 = ct{1080};
t2947 = ct{1081};
t2948 = ct{1082};
t2949 = ct{1083};
t2950 = ct{1084};
t2951 = ct{1085};
t2953 = ct{1086};
t2954 = ct{1087};
t2956 = ct{1088};
t2957 = ct{1089};
t2959 = ct{1090};
t2961 = ct{1091};
t2966 = ct{1092};
t2967 = ct{1093};
t2968 = ct{1094};
t2970 = ct{1095};
t2971 = ct{1096};
t2972 = ct{1097};
t2974 = ct{1098};
t2975 = ct{1099};
t2978 = ct{1100};
t2979 = ct{1101};
t2981 = ct{1102};
t2982 = ct{1103};
t2983 = ct{1104};
t2985 = ct{1105};
t2988 = ct{1106};
t2989 = ct{1107};
t299 = ct{1108};
t2991 = ct{1109};
t2992 = ct{1110};
t2994 = ct{1111};
t2995 = ct{1112};
t2996 = ct{1113};
t2997 = ct{1114};
t2998 = ct{1115};
t2999 = ct{1116};
t2d = ct{1117};
t2dd = ct{1118};
t30 = ct{1119};
t3000 = ct{1120};
t3003 = ct{1121};
t3004 = ct{1122};
t3005 = ct{1123};
t3006 = ct{1124};
t3007 = ct{1125};
t3009 = ct{1126};
t301 = ct{1127};
t3010 = ct{1128};
t3011 = ct{1129};
t3012 = ct{1130};
t3013 = ct{1131};
t3014 = ct{1132};
t3017 = ct{1133};
t3018 = ct{1134};
t3019 = ct{1135};
t3025 = ct{1136};
t3028 = ct{1137};
t3029 = ct{1138};
t3032 = ct{1139};
t3035 = ct{1140};
t3037 = ct{1141};
t3043 = ct{1142};
t3044 = ct{1143};
t3047 = ct{1144};
t3048 = ct{1145};
t3049 = ct{1146};
t3050 = ct{1147};
t3052 = ct{1148};
t3055 = ct{1149};
t3057 = ct{1150};
t3058 = ct{1151};
t3059 = ct{1152};
t3065 = ct{1153};
t3066 = ct{1154};
t3069 = ct{1155};
t3073 = ct{1156};
t3074 = ct{1157};
t3075 = ct{1158};
t3076 = ct{1159};
t3078 = ct{1160};
t3079 = ct{1161};
t308 = ct{1162};
t3080 = ct{1163};
t3081 = ct{1164};
t3082 = ct{1165};
t3083 = ct{1166};
t3085 = ct{1167};
t3086 = ct{1168};
t3087 = ct{1169};
t3088 = ct{1170};
t3089 = ct{1171};
t3090 = ct{1172};
t3091 = ct{1173};
t3092 = ct{1174};
t3093 = ct{1175};
t3096 = ct{1176};
t3098 = ct{1177};
t3099 = ct{1178};
t31 = ct{1179};
t3100 = ct{1180};
t3101 = ct{1181};
t3104 = ct{1182};
t3106 = ct{1183};
t3107 = ct{1184};
t3108 = ct{1185};
t3112 = ct{1186};
t3113 = ct{1187};
t3115 = ct{1188};
t3120 = ct{1189};
t3121 = ct{1190};
t3123 = ct{1191};
t3124 = ct{1192};
t3125 = ct{1193};
t3126 = ct{1194};
t3129 = ct{1195};
t3130 = ct{1196};
t3135 = ct{1197};
t3136 = ct{1198};
t3137 = ct{1199};
t3138 = ct{1200};
t3139 = ct{1201};
t3140 = ct{1202};
t3141 = ct{1203};
t3142 = ct{1204};
t3143 = ct{1205};
t3146 = ct{1206};
t315 = ct{1207};
t3150 = ct{1208};
t3151 = ct{1209};
t3153 = ct{1210};
t3155 = ct{1211};
t3156 = ct{1212};
t3157 = ct{1213};
t3158 = ct{1214};
t3159 = ct{1215};
t3161 = ct{1216};
t3162 = ct{1217};
t3163 = ct{1218};
t3165 = ct{1219};
t3166 = ct{1220};
t3168 = ct{1221};
t3169 = ct{1222};
t317 = ct{1223};
t3170 = ct{1224};
t3171 = ct{1225};
t3172 = ct{1226};
t3173 = ct{1227};
t3174 = ct{1228};
t3175 = ct{1229};
t3176 = ct{1230};
t3177 = ct{1231};
t3179 = ct{1232};
t318 = ct{1233};
t3180 = ct{1234};
t3182 = ct{1235};
t3183 = ct{1236};
t3185 = ct{1237};
t3187 = ct{1238};
t319 = ct{1239};
t3192 = ct{1240};
t3194 = ct{1241};
t3195 = ct{1242};
t3196 = ct{1243};
t3197 = ct{1244};
t3204 = ct{1245};
t3214 = ct{1246};
t3220 = ct{1247};
t3230 = ct{1248};
t3231 = ct{1249};
t3232 = ct{1250};
t3234 = ct{1251};
t3236 = ct{1252};
t3237 = ct{1253};
t3240 = ct{1254};
t3244 = ct{1255};
t3246 = ct{1256};
t325 = ct{1257};
t3251 = ct{1258};
t3253 = ct{1259};
t3258 = ct{1260};
t3260 = ct{1261};
t3267 = ct{1262};
t3268 = ct{1263};
t3272 = ct{1264};
t3275 = ct{1265};
t3278 = ct{1266};
t3283 = ct{1267};
t3285 = ct{1268};
t3288 = ct{1269};
t3289 = ct{1270};
t329 = ct{1271};
t3291 = ct{1272};
t3292 = ct{1273};
t3298 = ct{1274};
t330 = ct{1275};
t3302 = ct{1276};
t3305 = ct{1277};
t3306 = ct{1278};
t3308 = ct{1279};
t3313 = ct{1280};
t3318 = ct{1281};
t3319 = ct{1282};
t332 = ct{1283};
t3321 = ct{1284};
t3322 = ct{1285};
t3323 = ct{1286};
t3326 = ct{1287};
t333 = ct{1288};
t3330 = ct{1289};
t3331 = ct{1290};
t3332 = ct{1291};
t3335 = ct{1292};
t3339 = ct{1293};
t3340 = ct{1294};
t3348 = ct{1295};
t3349 = ct{1296};
t3351 = ct{1297};
t3354 = ct{1298};
t3355 = ct{1299};
t3358 = ct{1300};
t3359 = ct{1301};
t3360 = ct{1302};
t3367 = ct{1303};
t3377 = ct{1304};
t3378 = ct{1305};
t3380 = ct{1306};
t3381 = ct{1307};
t3383 = ct{1308};
t3384 = ct{1309};
t3387 = ct{1310};
t3388 = ct{1311};
t3390 = ct{1312};
t3391 = ct{1313};
t3399 = ct{1314};
t34 = ct{1315};
t3400 = ct{1316};
t3401 = ct{1317};
t3403 = ct{1318};
t3404 = ct{1319};
t3405 = ct{1320};
t341 = ct{1321};
t3414 = ct{1322};
t3415 = ct{1323};
t3416 = ct{1324};
t3417 = ct{1325};
t342 = ct{1326};
t3421 = ct{1327};
t3429 = ct{1328};
t343 = ct{1329};
t3431 = ct{1330};
t3432 = ct{1331};
t3439 = ct{1332};
t344 = ct{1333};
t3440 = ct{1334};
t3445 = ct{1335};
t3451 = ct{1336};
t3452 = ct{1337};
t3453 = ct{1338};
t3454 = ct{1339};
t3455 = ct{1340};
t3456 = ct{1341};
t3457 = ct{1342};
t3458 = ct{1343};
t3459 = ct{1344};
t346 = ct{1345};
t3460 = ct{1346};
t3461 = ct{1347};
t3463 = ct{1348};
t3468 = ct{1349};
t3469 = ct{1350};
t347 = ct{1351};
t3472 = ct{1352};
t3473 = ct{1353};
t3474 = ct{1354};
t3475 = ct{1355};
t3477 = ct{1356};
t3478 = ct{1357};
t3479 = ct{1358};
t3480 = ct{1359};
t3481 = ct{1360};
t3483 = ct{1361};
t3488 = ct{1362};
t3490 = ct{1363};
t3493 = ct{1364};
t3495 = ct{1365};
t3499 = ct{1366};
t35 = ct{1367};
t3502 = ct{1368};
t3503 = ct{1369};
t3504 = ct{1370};
t3506 = ct{1371};
t3508 = ct{1372};
t3509 = ct{1373};
t3510 = ct{1374};
t3515 = ct{1375};
t3516 = ct{1376};
t3517 = ct{1377};
t3518 = ct{1378};
t3521 = ct{1379};
t3523 = ct{1380};
t3527 = ct{1381};
t3532 = ct{1382};
t3534 = ct{1383};
t3536 = ct{1384};
t3537 = ct{1385};
t3538 = ct{1386};
t3539 = ct{1387};
t354 = ct{1388};
t3540 = ct{1389};
t3543 = ct{1390};
t3544 = ct{1391};
t3547 = ct{1392};
t3549 = ct{1393};
t3551 = ct{1394};
t3555 = ct{1395};
t3556 = ct{1396};
t3557 = ct{1397};
t3558 = ct{1398};
t3559 = ct{1399};
t3563 = ct{1400};
t3565 = ct{1401};
t3568 = ct{1402};
t3569 = ct{1403};
t3571 = ct{1404};
t3573 = ct{1405};
t3574 = ct{1406};
t3575 = ct{1407};
t3577 = ct{1408};
t3578 = ct{1409};
t3579 = ct{1410};
t3580 = ct{1411};
t3582 = ct{1412};
t3586 = ct{1413};
t3587 = ct{1414};
t3588 = ct{1415};
t3589 = ct{1416};
t3590 = ct{1417};
t3591 = ct{1418};
t3598 = ct{1419};
t36 = ct{1420};
t3600 = ct{1421};
t3601 = ct{1422};
t3602 = ct{1423};
t3603 = ct{1424};
t3604 = ct{1425};
t3606 = ct{1426};
t3607 = ct{1427};
t3609 = ct{1428};
t3610 = ct{1429};
t3611 = ct{1430};
t3613 = ct{1431};
t3615 = ct{1432};
t3617 = ct{1433};
t3620 = ct{1434};
t3622 = ct{1435};
t3623 = ct{1436};
t3624 = ct{1437};
t3625 = ct{1438};
t3626 = ct{1439};
t3627 = ct{1440};
t3628 = ct{1441};
t3630 = ct{1442};
t3634 = ct{1443};
t3635 = ct{1444};
t3637 = ct{1445};
t3639 = ct{1446};
t364 = ct{1447};
t3649 = ct{1448};
t365 = ct{1449};
t3650 = ct{1450};
t3651 = ct{1451};
t3668 = ct{1452};
t3670 = ct{1453};
t3675 = ct{1454};
t368 = ct{1455};
t3682 = ct{1456};
t3683 = ct{1457};
t3684 = ct{1458};
t3685 = ct{1459};
t3686 = ct{1460};
t3687 = ct{1461};
t3690 = ct{1462};
t3697 = ct{1463};
t37 = ct{1464};
t3701 = ct{1465};
t3712 = ct{1466};
t3716 = ct{1467};
t3722 = ct{1468};
t3732 = ct{1469};
t3733 = ct{1470};
t3734 = ct{1471};
t3739 = ct{1472};
t3741 = ct{1473};
t3744 = ct{1474};
t3745 = ct{1475};
t3747 = ct{1476};
t3750 = ct{1477};
t3751 = ct{1478};
t3753 = ct{1479};
t3754 = ct{1480};
t3755 = ct{1481};
t3756 = ct{1482};
t3757 = ct{1483};
t3762 = ct{1484};
t3763 = ct{1485};
t3764 = ct{1486};
t3766 = ct{1487};
t3768 = ct{1488};
t3770 = ct{1489};
t3771 = ct{1490};
t3780 = ct{1491};
t3781 = ct{1492};
t3783 = ct{1493};
t3784 = ct{1494};
t3785 = ct{1495};
t3787 = ct{1496};
t3789 = ct{1497};
t3792 = ct{1498};
t38 = ct{1499};
t3800 = ct{1500};
t3804 = ct{1501};
t3809 = ct{1502};
t3810 = ct{1503};
t3811 = ct{1504};
t3812 = ct{1505};
t3817 = ct{1506};
t3821 = ct{1507};
t3822 = ct{1508};
t3826 = ct{1509};
t3828 = ct{1510};
t3830 = ct{1511};
t3832 = ct{1512};
t3833 = ct{1513};
t3838 = ct{1514};
t384 = ct{1515};
t3840 = ct{1516};
t3843 = ct{1517};
t3848 = ct{1518};
t3858 = ct{1519};
t3860 = ct{1520};
t3861 = ct{1521};
t3863 = ct{1522};
t3866 = ct{1523};
t3867 = ct{1524};
t3871 = ct{1525};
t3872 = ct{1526};
t3874 = ct{1527};
t3875 = ct{1528};
t3880 = ct{1529};
t3886 = ct{1530};
t3887 = ct{1531};
t3888 = ct{1532};
t3889 = ct{1533};
t3890 = ct{1534};
t3892 = ct{1535};
t3894 = ct{1536};
t3896 = ct{1537};
t3897 = ct{1538};
t39 = ct{1539};
t3900 = ct{1540};
t3903 = ct{1541};
t3917 = ct{1542};
t3919 = ct{1543};
t392 = ct{1544};
t3923 = ct{1545};
t3927 = ct{1546};
t393 = ct{1547};
t3931 = ct{1548};
t3932 = ct{1549};
t3933 = ct{1550};
t3936 = ct{1551};
t3937 = ct{1552};
t3943 = ct{1553};
t3950 = ct{1554};
t3956 = ct{1555};
t3958 = ct{1556};
t3959 = ct{1557};
t3962 = ct{1558};
t3963 = ct{1559};
t3965 = ct{1560};
t3967 = ct{1561};
t3972 = ct{1562};
t3976 = ct{1563};
t3978 = ct{1564};
t3982 = ct{1565};
t3983 = ct{1566};
t3989 = ct{1567};
t3990 = ct{1568};
t3993 = ct{1569};
t3994 = ct{1570};
t3997 = ct{1571};
t3d = ct{1572};
t3dd = ct{1573};
t4001 = ct{1574};
t4002 = ct{1575};
t4003 = ct{1576};
t4005 = ct{1577};
t4006 = ct{1578};
t4007 = ct{1579};
t401 = ct{1580};
t4012 = ct{1581};
t4014 = ct{1582};
t4017 = ct{1583};
t4018 = ct{1584};
t4019 = ct{1585};
t402 = ct{1586};
t4023 = ct{1587};
t4025 = ct{1588};
t4026 = ct{1589};
t4027 = ct{1590};
t403 = ct{1591};
t4030 = ct{1592};
t4038 = ct{1593};
t404 = ct{1594};
t4041 = ct{1595};
t4042 = ct{1596};
t4045 = ct{1597};
t4046 = ct{1598};
t4047 = ct{1599};
t4048 = ct{1600};
t4049 = ct{1601};
t4050 = ct{1602};
t4053 = ct{1603};
t4059 = ct{1604};
t4066 = ct{1605};
t4067 = ct{1606};
t4068 = ct{1607};
t4069 = ct{1608};
t4071 = ct{1609};
t4073 = ct{1610};
t4074 = ct{1611};
t4078 = ct{1612};
t4081 = ct{1613};
t4084 = ct{1614};
t4086 = ct{1615};
t4087 = ct{1616};
t4090 = ct{1617};
t4091 = ct{1618};
t4095 = ct{1619};
t4096 = ct{1620};
t4097 = ct{1621};
t41 = ct{1622};
t4101 = ct{1623};
t4102 = ct{1624};
t4112 = ct{1625};
t4113 = ct{1626};
t4115 = ct{1627};
t4117 = ct{1628};
t4118 = ct{1629};
t4121 = ct{1630};
t4122 = ct{1631};
t4125 = ct{1632};
t4126 = ct{1633};
t4128 = ct{1634};
t4130 = ct{1635};
t4131 = ct{1636};
t4133 = ct{1637};
t4134 = ct{1638};
t4136 = ct{1639};
t4137 = ct{1640};
t4139 = ct{1641};
t4140 = ct{1642};
t4142 = ct{1643};
t4143 = ct{1644};
t4144 = ct{1645};
t4145 = ct{1646};
t4146 = ct{1647};
t4147 = ct{1648};
t4148 = ct{1649};
t4149 = ct{1650};
t4151 = ct{1651};
t4152 = ct{1652};
t4155 = ct{1653};
t4156 = ct{1654};
t4157 = ct{1655};
t4158 = ct{1656};
t4159 = ct{1657};
t4160 = ct{1658};
t4162 = ct{1659};
t4164 = ct{1660};
t4166 = ct{1661};
t4167 = ct{1662};
t4168 = ct{1663};
t4170 = ct{1664};
t4171 = ct{1665};
t4172 = ct{1666};
t4174 = ct{1667};
t4176 = ct{1668};
t4178 = ct{1669};
t418 = ct{1670};
t4180 = ct{1671};
t4182 = ct{1672};
t4183 = ct{1673};
t4185 = ct{1674};
t4186 = ct{1675};
t4187 = ct{1676};
t4188 = ct{1677};
t4189 = ct{1678};
t419 = ct{1679};
t4192 = ct{1680};
t4193 = ct{1681};
t4194 = ct{1682};
t4195 = ct{1683};
t4196 = ct{1684};
t42 = ct{1685};
t420 = ct{1686};
t4202 = ct{1687};
t4203 = ct{1688};
t4204 = ct{1689};
t4208 = ct{1690};
t4212 = ct{1691};
t4215 = ct{1692};
t4217 = ct{1693};
t4220 = ct{1694};
t4221 = ct{1695};
t4222 = ct{1696};
t4225 = ct{1697};
t4226 = ct{1698};
t4230 = ct{1699};
t4231 = ct{1700};
t4233 = ct{1701};
t4236 = ct{1702};
t4237 = ct{1703};
t425 = ct{1704};
t4251 = ct{1705};
t4252 = ct{1706};
t4255 = ct{1707};
t4256 = ct{1708};
t4267 = ct{1709};
t4283 = ct{1710};
t4290 = ct{1711};
t4294 = ct{1712};
t4296 = ct{1713};
t4299 = ct{1714};
t4302 = ct{1715};
t4304 = ct{1716};
t4309 = ct{1717};
t431 = ct{1718};
t4321 = ct{1719};
t4324 = ct{1720};
t4325 = ct{1721};
t4327 = ct{1722};
t4330 = ct{1723};
t4331 = ct{1724};
t4332 = ct{1725};
t4333 = ct{1726};
t4334 = ct{1727};
t4335 = ct{1728};
t4337 = ct{1729};
t434 = ct{1730};
t4348 = ct{1731};
t4351 = ct{1732};
t4353 = ct{1733};
t4361 = ct{1734};
t4367 = ct{1735};
t437 = ct{1736};
t4371 = ct{1737};
t4393 = ct{1738};
t4394 = ct{1739};
t4395 = ct{1740};
t4399 = ct{1741};
t4402 = ct{1742};
t4403 = ct{1743};
t4404 = ct{1744};
t4406 = ct{1745};
t4408 = ct{1746};
t441 = ct{1747};
t4410 = ct{1748};
t4413 = ct{1749};
t442 = ct{1750};
t4421 = ct{1751};
t4424 = ct{1752};
t4428 = ct{1753};
t4429 = ct{1754};
t443 = ct{1755};
t4430 = ct{1756};
t4431 = ct{1757};
t4444 = ct{1758};
t4450 = ct{1759};
t4451 = ct{1760};
t4454 = ct{1761};
t4457 = ct{1762};
t4459 = ct{1763};
t446 = ct{1764};
t4460 = ct{1765};
t4461 = ct{1766};
t4467 = ct{1767};
t4468 = ct{1768};
t4470 = ct{1769};
t4475 = ct{1770};
t4479 = ct{1771};
t4480 = ct{1772};
t4483 = ct{1773};
t4486 = ct{1774};
t4487 = ct{1775};
t4491 = ct{1776};
t4493 = ct{1777};
t4494 = ct{1778};
t4499 = ct{1779};
t4500 = ct{1780};
t4503 = ct{1781};
t4508 = ct{1782};
t4512 = ct{1783};
t4513 = ct{1784};
t4526 = ct{1785};
t4528 = ct{1786};
t4529 = ct{1787};
t453 = ct{1788};
t4531 = ct{1789};
t4533 = ct{1790};
t4534 = ct{1791};
t4538 = ct{1792};
t4539 = ct{1793};
t454 = ct{1794};
t4540 = ct{1795};
t4541 = ct{1796};
t4542 = ct{1797};
t4547 = ct{1798};
t4548 = ct{1799};
t4549 = ct{1800};
t4551 = ct{1801};
t4553 = ct{1802};
t4556 = ct{1803};
t4561 = ct{1804};
t4563 = ct{1805};
t4566 = ct{1806};
t4579 = ct{1807};
t4582 = ct{1808};
t459 = ct{1809};
t4591 = ct{1810};
t4592 = ct{1811};
t4595 = ct{1812};
t4596 = ct{1813};
t4599 = ct{1814};
t4604 = ct{1815};
t4607 = ct{1816};
t4608 = ct{1817};
t4615 = ct{1818};
t4620 = ct{1819};
t4623 = ct{1820};
t4626 = ct{1821};
t4627 = ct{1822};
t4629 = ct{1823};
t4632 = ct{1824};
t4633 = ct{1825};
t4642 = ct{1826};
t4647 = ct{1827};
t4648 = ct{1828};
t4655 = ct{1829};
t4664 = ct{1830};
t4665 = ct{1831};
t4666 = ct{1832};
t4668 = ct{1833};
t4670 = ct{1834};
t4672 = ct{1835};
t4673 = ct{1836};
t4675 = ct{1837};
t4676 = ct{1838};
t4677 = ct{1839};
t4678 = ct{1840};
t4681 = ct{1841};
t4683 = ct{1842};
t4688 = ct{1843};
t4694 = ct{1844};
t4695 = ct{1845};
t4699 = ct{1846};
t470 = ct{1847};
t4703 = ct{1848};
t4704 = ct{1849};
t4705 = ct{1850};
t4707 = ct{1851};
t4708 = ct{1852};
t4714 = ct{1853};
t4715 = ct{1854};
t4716 = ct{1855};
t4720 = ct{1856};
t4722 = ct{1857};
t4727 = ct{1858};
t4747 = ct{1859};
t4757 = ct{1860};
t4759 = ct{1861};
t4765 = ct{1862};
t4771 = ct{1863};
t4776 = ct{1864};
t478 = ct{1865};
t4785 = ct{1866};
t4786 = ct{1867};
t4792 = ct{1868};
t4795 = ct{1869};
t4798 = ct{1870};
t4799 = ct{1871};
t48 = ct{1872};
t4801 = ct{1873};
t4802 = ct{1874};
t4813 = ct{1875};
t4815 = ct{1876};
t4817 = ct{1877};
t483 = ct{1878};
t4831 = ct{1879};
t4836 = ct{1880};
t4837 = ct{1881};
t4838 = ct{1882};
t484 = ct{1883};
t4840 = ct{1884};
t4845 = ct{1885};
t4846 = ct{1886};
t4855 = ct{1887};
t4856 = ct{1888};
t4858 = ct{1889};
t4859 = ct{1890};
t486 = ct{1891};
t4861 = ct{1892};
t4862 = ct{1893};
t4865 = ct{1894};
t4867 = ct{1895};
t487 = ct{1896};
t4870 = ct{1897};
t4871 = ct{1898};
t4874 = ct{1899};
t4878 = ct{1900};
t488 = ct{1901};
t4881 = ct{1902};
t4883 = ct{1903};
t4887 = ct{1904};
t4889 = ct{1905};
t4891 = ct{1906};
t4896 = ct{1907};
t4908 = ct{1908};
t4909 = ct{1909};
t4917 = ct{1910};
t492 = ct{1911};
t4920 = ct{1912};
t4922 = ct{1913};
t4923 = ct{1914};
t4924 = ct{1915};
t4926 = ct{1916};
t4929 = ct{1917};
t493 = ct{1918};
t4930 = ct{1919};
t4931 = ct{1920};
t4932 = ct{1921};
t4935 = ct{1922};
t494 = ct{1923};
t4941 = ct{1924};
t4944 = ct{1925};
t4946 = ct{1926};
t4949 = ct{1927};
t495 = ct{1928};
t4950 = ct{1929};
t4951 = ct{1930};
t4952 = ct{1931};
t4955 = ct{1932};
t4956 = ct{1933};
t4957 = ct{1934};
t4958 = ct{1935};
t4959 = ct{1936};
t496 = ct{1937};
t4967 = ct{1938};
t497 = ct{1939};
t4979 = ct{1940};
t498 = ct{1941};
t4981 = ct{1942};
t4985 = ct{1943};
t4990 = ct{1944};
t4992 = ct{1945};
t4993 = ct{1946};
t4997 = ct{1947};
t4d = ct{1948};
t4dd = ct{1949};
t50 = ct{1950};
t5001 = ct{1951};
t5006 = ct{1952};
t501 = ct{1953};
t5010 = ct{1954};
t5011 = ct{1955};
t5012 = ct{1956};
t5013 = ct{1957};
t5018 = ct{1958};
t5019 = ct{1959};
t5020 = ct{1960};
t5026 = ct{1961};
t503 = ct{1962};
t5036 = ct{1963};
t5038 = ct{1964};
t5040 = ct{1965};
t5041 = ct{1966};
t5043 = ct{1967};
t5047 = ct{1968};
t5051 = ct{1969};
t5056 = ct{1970};
t5070 = ct{1971};
t5074 = ct{1972};
t508 = ct{1973};
t5081 = ct{1974};
t5091 = ct{1975};
t5092 = ct{1976};
t5093 = ct{1977};
t5098 = ct{1978};
t51 = ct{1979};
t5104 = ct{1980};
t5116 = ct{1981};
t5117 = ct{1982};
t5119 = ct{1983};
t5123 = ct{1984};
t5131 = ct{1985};
t5136 = ct{1986};
t514 = ct{1987};
t5141 = ct{1988};
t515 = ct{1989};
t516 = ct{1990};
t5163 = ct{1991};
t5171 = ct{1992};
t5175 = ct{1993};
t5176 = ct{1994};
t519 = ct{1995};
t5219 = ct{1996};
t5223 = ct{1997};
t523 = ct{1998};
t524 = ct{1999};
t5255 = ct{2000};
t5258 = ct{2001};
t5278 = ct{2002};
t5281 = ct{2003};
t5283 = ct{2004};
t529 = ct{2005};
t5292 = ct{2006};
t53 = ct{2007};
t530 = ct{2008};
t532 = ct{2009};
t5351 = ct{2010};
t537 = ct{2011};
t5401 = ct{2012};
t5403 = ct{2013};
t543 = ct{2014};
t544 = ct{2015};
t546 = ct{2016};
t5465 = ct{2017};
t547 = ct{2018};
t5476 = ct{2019};
t548 = ct{2020};
t549 = ct{2021};
t55 = ct{2022};
t5501 = ct{2023};
t5513 = ct{2024};
t5516 = ct{2025};
t552 = ct{2026};
t553 = ct{2027};
t554 = ct{2028};
t56 = ct{2029};
t562 = ct{2030};
t569 = ct{2031};
t57 = ct{2032};
t570 = ct{2033};
t58 = ct{2034};
t582 = ct{2035};
t588 = ct{2036};
t589 = ct{2037};
t591 = ct{2038};
t593 = ct{2039};
t598 = ct{2040};
t5d = ct{2041};
t5dd = ct{2042};
t601 = ct{2043};
t602 = ct{2044};
t604 = ct{2045};
t608 = ct{2046};
t609 = ct{2047};
t61 = ct{2048};
t612 = ct{2049};
t614 = ct{2050};
t615 = ct{2051};
t616 = ct{2052};
t617 = ct{2053};
t623 = ct{2054};
t627 = ct{2055};
t63 = ct{2056};
t632 = ct{2057};
t633 = ct{2058};
t634 = ct{2059};
t635 = ct{2060};
t636 = ct{2061};
t637 = ct{2062};
t639 = ct{2063};
t641 = ct{2064};
t645 = ct{2065};
t646 = ct{2066};
t647 = ct{2067};
t648 = ct{2068};
t649 = ct{2069};
t650 = ct{2070};
t652 = ct{2071};
t653 = ct{2072};
t655 = ct{2073};
t659 = ct{2074};
t664 = ct{2075};
t667 = ct{2076};
t670 = ct{2077};
t671 = ct{2078};
t675 = ct{2079};
t680 = ct{2080};
t681 = ct{2081};
t682 = ct{2082};
t687 = ct{2083};
t69 = ct{2084};
t690 = ct{2085};
t691 = ct{2086};
t694 = ct{2087};
t695 = ct{2088};
t696 = ct{2089};
t698 = ct{2090};
t699 = ct{2091};
t6d = ct{2092};
t6dd = ct{2093};
t702 = ct{2094};
t703 = ct{2095};
t705 = ct{2096};
t706 = ct{2097};
t71 = ct{2098};
t711 = ct{2099};
t712 = ct{2100};
t713 = ct{2101};
t714 = ct{2102};
t720 = ct{2103};
t721 = ct{2104};
t723 = ct{2105};
t725 = ct{2106};
t726 = ct{2107};
t729 = ct{2108};
t731 = ct{2109};
t732 = ct{2110};
t733 = ct{2111};
t735 = ct{2112};
t736 = ct{2113};
t738 = ct{2114};
t739 = ct{2115};
t745 = ct{2116};
t746 = ct{2117};
t747 = ct{2118};
t748 = ct{2119};
t75 = ct{2120};
t752 = ct{2121};
t755 = ct{2122};
t759 = ct{2123};
t760 = ct{2124};
t761 = ct{2125};
t763 = ct{2126};
t764 = ct{2127};
t775 = ct{2128};
t776 = ct{2129};
t781 = ct{2130};
t785 = ct{2131};
t788 = ct{2132};
t789 = ct{2133};
t793 = ct{2134};
t8 = ct{2135};
t802 = ct{2136};
t806 = ct{2137};
t82 = ct{2138};
t820 = ct{2139};
t824 = ct{2140};
t828 = ct{2141};
t831 = ct{2142};
t832 = ct{2143};
t833 = ct{2144};
t838 = ct{2145};
t842 = ct{2146};
t843 = ct{2147};
t844 = ct{2148};
t846 = ct{2149};
t848 = ct{2150};
t849 = ct{2151};
t850 = ct{2152};
t851 = ct{2153};
t852 = ct{2154};
t853 = ct{2155};
t854 = ct{2156};
t855 = ct{2157};
t859 = ct{2158};
t861 = ct{2159};
t865 = ct{2160};
t870 = ct{2161};
t871 = ct{2162};
t873 = ct{2163};
t879 = ct{2164};
t880 = ct{2165};
t884 = ct{2166};
t885 = ct{2167};
t890 = ct{2168};
t892 = ct{2169};
t896 = ct{2170};
t897 = ct{2171};
t898 = ct{2172};
t899 = ct{2173};
t9 = ct{2174};
t900 = ct{2175};
t907 = ct{2176};
t909 = ct{2177};
t910 = ct{2178};
t915 = ct{2179};
t917 = ct{2180};
t919 = ct{2181};
t922 = ct{2182};
t923 = ct{2183};
t927 = ct{2184};
t928 = ct{2185};
t930 = ct{2186};
t932 = ct{2187};
t937 = ct{2188};
t943 = ct{2189};
t944 = ct{2190};
t945 = ct{2191};
t949 = ct{2192};
t952 = ct{2193};
t959 = ct{2194};
t961 = ct{2195};
t962 = ct{2196};
t963 = ct{2197};
t964 = ct{2198};
t965 = ct{2199};
t966 = ct{2200};
t967 = ct{2201};
t969 = ct{2202};
t970 = ct{2203};
t972 = ct{2204};
t973 = ct{2205};
t978 = ct{2206};
t979 = ct{2207};
t981 = ct{2208};
t982 = ct{2209};
t983 = ct{2210};
t986 = ct{2211};
t987 = ct{2212};
t989 = ct{2213};
t992 = ct{2214};
t999 = ct{2215};
t3181 = -t3136;
t3191 = t1796+t1826;
t3193 = -t3146;
t3200 = t3136./2.0;
t3205 = t3143./2.0;
t3206 = t3146./2.0;
t3208 = t1665+t2016;
t3212 = t8.*t39.*t3091;
t3213 = t3153./2.0;
t3215 = -t37.*(t1580+t2001);
t3219 = t3156./2.0;
t3221 = t3159./2.0;
t3226 = t3194.*t5d;
t3228 = t3174./2.0;
t3239 = t3187./2.0;
t3241 = -t1d.*(t1643-t2016);
t3242 = -t18.*t39.*(t1580+t2001);
t3243 = t37.*t3150;
t3247 = t14.*t37.*t3104;
t3249 = t1767+t1979;
t3252 = t8.*t39.*(t1913-t898.*(t100-t364));
t3255 = t255.*t3019;
t3256 = t37.*(t1580+t2001).*(-1.0./2.0);
t3257 = t1d.*(t1643-t2016);
t3263 = t18.*t39.*t3150;
t3264 = t18.*t39.*(t1580+t2001);
t3265 = (t37.*(t1580+t2001))./2.0;
t3266 = -t3244;
t3271 = -t3258;
t3274 = t256.*t3047;
t3276 = -t3253;
t3277 = t329.*t3019;
t3282 = t3244./2.0;
t3286 = (t14.*t39.*t3104)./2.0;
t3290 = t3253./2.0;
t3300 = t330.*t3047;
t3310 = t3275./2.0;
t3312 = t3278./2.0;
t3316 = -t3302;
t3325 = t3302./2.0;
t3327 = t3313.*t1d;
t3328 = t1893+t2000;
t3329 = t1934+t1981;
t3338 = t330.*t3091;
t3350 = (t8.*t3305)./2.0;
t3352 = t330.*(t1913-t898.*(t100-t364));
t3356 = t1927+t2028;
t3365 = t3339./2.0;
t3369 = (t14.*t3323)./2.0;
t3370 = t37.*t3322;
t3371 = t1619+t2319;
t3374 = t14.*t39.*t3305;
t3375 = t1622+t2326;
t3376 = t37.*t3319;
t3392 = t18.*t39.*t3322;
t3395 = t8.*t39.*t3323;
t3426 = t3403.*t6d;
t3442 = (t8.*t3367)./2.0;
t3450 = t128+t1346+t1347+t1348;
t3465 = t1642+t2416;
t3471 = t1638+t2409;
t3476 = t14.*t39.*t3367;
t3482 = t255.*t3305;
t3484 = t3474.*(-1.0./2.0);
t3489 = t8.*t3451;
t3491 = t3474./2.0;
t3494 = t14.*t3463;
t3512 = t330.*t3323;
t3524 = t3508.*t2d;
t3525 = t3508.*t3d;
t3526 = t3508.*t4d;
t3529 = t3506./2.0;
t3533 = t14.*t39.*t3451;
t3535 = t8.*t39.*t3463;
t3548 = t37.*t3499;
t3552 = t39.*t3499;
t3554 = t255.*t3367;
t3564 = t3559.*(-1.0./2.0);
t3572 = t14.*t3534;
t3581 = -t3558;
t3583 = t3559./2.0;
t3605 = t3558./2.0;
t3608 = t37.*t3527;
t3619 = t14.*t3569;
t3621 = t8.*t3589;
t3631 = t18.*t39.*t3527;
t3632 = t8.*t37.*t3534;
t3633 = t8.*t39.*t3534;
t3636 = t3615.*t2dd;
t3638 = t3615.*t3dd;
t3640 = t3615.*t4dd;
t3641 = t1423+t1430+t1717;
t3642 = t384+t681+t690+t1350+t1367;
t3643 = t18.*t3609;
t3647 = t18.*t3611;
t3648 = t3611./2.0;
t3653 = t37.*t3565;
t3655 = t8.*t3627;
t3662 = t35.*t39.*t3534;
t3665 = t8.*t39.*t3569;
t3666 = t1393+t1496+t1747;
t3667 = t330.*t3463;
t3669 = t37.*t3603;
t3671 = t39.*t3603;
t3673 = t18.*t39.*t3565;
t3679 = t14.*t37.*t3589;
t3680 = t14.*t39.*t3589;
t3693 = -t3684;
t3694 = t18.*t3668;
t3699 = -t3675;
t3702 = t38.*t39.*t3589;
t3708 = t3690.*t5d;
t3709 = t1406+t1524+t1746;
t3710 = t3670./2.0;
t3715 = t3675./2.0;
t3719 = t14.*t39.*t3627;
t3749 = t256.*t3534;
t3772 = t330.*t3534;
t3788 = t3763.*t6d;
t3795 = t255.*t3589;
t3799 = t1435+t1681+t1688;
t3802 = t330.*t3569;
t3805 = t3783.*t5d;
t3807 = (t14.*t3733)./2.0;
t3808 = t636+t2022+t2086;
t3815 = t329.*t3589;
t3818 = t8.*t39.*t3733;
t3819 = (t8.*t3764)./2.0;
t3825 = t255.*t3627;
t3829 = t14.*t3800;
t3839 = t3811./2.0;
t3841 = t14.*t39.*t3764;
t3868 = t14.*t3832;
t3882 = t8.*t37.*t3800;
t3883 = -t3860;
t3885 = t8.*t39.*t3800;
t3899 = t3860./2.0;
t3901 = -t3890;
t3904 = t14.*t3866;
t3908 = t3867./2.0;
t3912 = t35.*t39.*t3800;
t3913 = -t3880;
t3921 = -t3892;
t3924 = -t3896;
t3928 = t3880./2.0;
t3934 = t3892./2.0;
t3935 = -t14.*(t2574+t1532.*(t100-t364));
t3938 = t3896./2.0;
t3942 = t8.*t37.*t3832;
t3944 = t8.*t39.*t3832;
t3960 = -t3927;
t3964 = t330.*t3733;
t3966 = t35.*t39.*t3832;
t3969 = t255.*t3764;
t3971 = t3927./2.0;
t3975 = -t3963;
t3977 = t14.*(t2574+t1532.*(t100-t364)).*(-1.0./2.0);
t3979 = t3937./2.0;
t3984 = -t3959;
t3986 = t3950./2.0;
t3991 = t3958./2.0;
t3992 = t3959./2.0;
t3999 = -t3983;
t4008 = t3983./2.0;
t4009 = t3993.*t2dd;
t4010 = t3993.*t3dd;
t4011 = t3993.*t4dd;
t4016 = t330.*t3800;
t4020 = t1549+t1577+t2105;
t4022 = t37.*t3994;
t4034 = t4017./2.0;
t4036 = t18.*t39.*t3994;
t4040 = t4023./2.0;
t4052 = t4038./2.0;
t4054 = t1171+t1207+t1391+t1719;
t4056 = t4045./2.0;
t4057 = t4046./2.0;
t4065 = t4053./2.0;
t4070 = t4066.*t1d;
t4083 = -t4074;
t4092 = t2620+t2622;
t4093 = t37.*t4068;
t4094 = t39.*t4068;
t4108 = -t4101;
t4127 = -t4121;
t4154 = t2686+t2712;
t4161 = t37.*t4145;
t4163 = t37.*t4148;
t4190 = t14.*t4167;
t4191 = t14.*t4168;
t4197 = t852+t1229+t1613+t2278;
t4198 = t854+t1235+t1614+t2284;
t4200 = -t4192;
t4201 = -t4194;
t4206 = t1292+t1337+t1594+t1918;
t4213 = t8.*t4195;
t4214 = t8.*t4196;
t4218 = t1341+t1387+t1591+t1860;
t4223 = t8.*t37.*t4167;
t4224 = t8.*t39.*t4167;
t4227 = t4202.*t2d;
t4228 = t4202.*t3d;
t4229 = t4202.*t4d;
t4235 = t14.*t4208;
t4238 = t35.*t39.*t4167;
t4241 = t14.*t4225;
t4242 = t8.*t4215;
t4243 = t14.*t4217;
t4246 = t8.*t4220;
t4249 = t8.*t4222;
t4253 = t14.*t39.*t4195;
t4254 = t2769+t2833;
t4258 = t354+t1388+t1398+t2828;
t4260 = t14.*t37.*t4195;
t4266 = -t4251;
t4282 = t4251./2.0;
t4284 = t38.*t39.*t4195;
t4285 = t8.*t39.*t4208;
t4292 = t14.*t39.*t4222;
t4293 = t8.*t39.*t4225;
t4295 = t14.*t39.*t4215;
t4298 = t8.*t39.*t4217;
t4301 = t899+t907+t3563;
t4303 = t14.*t39.*t4220;
t4311 = t37.*t4255;
t4312 = -t4302;
t4317 = t1281+t1285+t3319;
t4319 = t330.*t4167;
t4328 = t18.*t39.*t4255;
t4336 = t255.*t4195;
t4341 = t1477+t1484+t1763+t1766;
t4346 = t1281+t1285+t1611+t2307;
t4349 = t202+t333+t1306+t1359+t1599+t1607;
t4355 = -t2d.*(-t1281+t3322+(t14.*(t478-t519))./2.0);
t4356 = -t3d.*(-t1281+t3322+(t14.*(t478-t519))./2.0);
t4357 = -t4d.*(-t1281+t3322+(t14.*(t478-t519))./2.0);
t4358 = t330.*t4208;
t4359 = t255.*t4222;
t4360 = t2892+t2949;
t4362 = t221+t344+t671+t714+t1019+t1064+t1099+t1143;
t4363 = t37.*t4330;
t4364 = t39.*t4330;
t4366 = t4351.*t5d;
t4372 = -t5d.*(-t221+t279-t671+t702+t1101+t2107+(t8.*t39.*(t206-t470))./2.0);
t4388 = t2974+t2975;
t4396 = t4393.*t5dd;
t4407 = t14.*t4402;
t4411 = t8.*t4404;
t4420 = t8.*t4410;
t4423 = t3049+t3074;
t4427 = t3055+t3096;
t4432 = t14.*t37.*t4404;
t4433 = t14.*t39.*t4404;
t4445 = t38.*t39.*t4404;
t4452 = t1616+t1634+t1912+t1915;
t4453 = t1635+t1675+t1851+t1854;
t4464 = -t4459;
t4473 = -t4461;
t4474 = t1625+t1664+t1949+t1952;
t4476 = t4461./2.0;
t4488 = (t255.*t4404)./2.0;
t4506 = t2724+t3604;
t4509 = t1782+t1876+t1877+t1878;
t4514 = t2624+t3744;
t4515 = t37.*t4500;
t4517 = t4512.*t5d;
t4519 = t18.*t39.*t4500;
t4532 = t850+t851+t4145;
t4536 = -t4155.*(t746-t748);
t4537 = t848+t849+t4148;
t4543 = t4529.*t1d;
t4546 = t4155.*(t746-t748);
t4550 = t4531./2.0;
t4552 = t4533./2.0;
t4562 = t4542./2.0;
t4565 = t14.*t4549;
t4568 = t8.*t4563;
t4572 = (t1875.*t4155)./2.0;
t4574 = t1824+t1926+t1990+t2065;
t4575 = t2817+t3753;
t4576 = t8.*t39.*t4549;
t4578 = t2855+t3722;
t4583 = t37.*t4566;
t4585 = t2854+t3766;
t4587 = t2818+t3784;
t4588 = t14.*t39.*t4563;
t4600 = t1869+t1975+t1996+t2069;
t4606 = -t4592;
t4611 = t1580+t2001+t2146+t2181;
t4612 = t4592./2.0;
t4621 = t4607./2.0;
t4622 = t1620+t1621+t2320+t2325;
t4631 = -t4620;
t4634 = t330.*t4549;
t4635 = t255.*t4563;
t4636 = t4620./2.0;
t4640 = t4633.*(-1.0./2.0);
t4641 = -t4626;
t4645 = -t4632;
t4646 = t4626./2.0;
t4650 = t4632./2.0;
t4652 = -t4647;
t4654 = t2194+t2230+t3150;
t4659 = t4655.*(-1.0./2.0);
t4679 = -t4670;
t4684 = t4670./2.0;
t4685 = t4673./2.0;
t4686 = t4681.*(-1.0./2.0);
t4700 = -t4694;
t4701 = t14.*t4688;
t4702 = t8.*t4683;
t4710 = t2879+t4017;
t4713 = t4703./2.0;
t4717 = t8.*t4708;
t4721 = -t4716;
t4723 = t8.*t39.*t4688;
t4724 = t14.*t39.*t4683;
t4725 = t14.*t4715;
t4728 = t3495+t3506;
t4730 = t14.*t4722;
t4732 = t2881+t4045;
t4737 = -t2d.*(t3478-t3506);
t4738 = -t3d.*(t3478-t3506);
t4739 = -t4d.*(t3478-t3506);
t4741 = t2530.*t4155;
t4744 = t8.*t4727;
t4758 = -t37.*(t2837-t4045);
t4760 = -t4757;
t4762 = -t18.*t39.*(t2837-t4045);
t4763 = t2912+t4073;
t4764 = t37.*(t2837-t4045).*(-1.0./2.0);
t4766 = t18.*t39.*(t2837-t4045);
t4767 = (t37.*(t2837-t4045))./2.0;
t4768 = -t4765;
t4770 = -t4428.*(t746-t748);
t4777 = t2942+t4081;
t4778 = -t4771;
t4780 = -t8.*(t4074+t459.*(t544-t1021+t330.*(t100-t364)));
t4783 = t4428.*(t746-t748).*(-1.0./2.0);
t4784 = t4771./2.0;
t4790 = t4786.*(-1.0./2.0);
t4794 = t4786./2.0;
t4796 = t8.*(t4074+t459.*(t544-t1021+t330.*(t100-t364))).*(-1.0./2.0);
t4807 = -t14.*t39.*(t4074+t459.*(t544-t1021+t330.*(t100-t364)));
t4810 = t2944+t4113;
t4822 = t1963+t1972+t2412+t2415;
t4825 = (t1875.*t4428)./2.0;
t4827 = t14.*t39.*(t4074+t459.*(t544-t1021+t330.*(t100-t364))).*(-1.0./2.0);
t4828 = -t4815;
t4829 = (t14.*t39.*(t4074+t459.*(t544-t1021+t330.*(t100-t364))))./2.0;
t4830 = t4815./2.0;
t4841 = t4836./2.0;
t4843 = -t255.*(t4074+t459.*(t544-t1021+t330.*(t100-t364)));
t4848 = t4845.*(-1.0./2.0);
t4849 = t255.*(t4074+t459.*(t544-t1021+t330.*(t100-t364))).*(-1.0./2.0);
t4851 = t4845./2.0;
t4860 = t4855./2.0;
t4873 = t3082.*t4155;
t4875 = t4865./2.0;
t4888 = -t4883;
t4890 = t4883./2.0;
t4895 = t3811+t3828;
t4898 = t2530.*t4428;
t4915 = t3867+t3897;
t4925 = t4922.*2.0;
t4934 = (t3405.*t4155)./2.0;
t4938 = -t4932;
t4939 = -t4935;
t4942 = t4932./2.0;
t4943 = t4935./2.0;
t4953 = t1282+t1286+t4566;
t4954 = -t4952;
t4960 = -t4959;
t4970 = t3082.*t4428;
t4975 = t1311+t2184+t2680+t3475;
t4984 = t3822.*t4155;
t5000 = t4997.*(-1.0./2.0);
t5002 = t4997./2.0;
t5014 = t5011.*2.0;
t5022 = t3405.*t4428;
t5025 = t5019./2.0;
t5030 = t1841+t1902+t4513;
t5032 = t4050.*t4155;
t5035 = t1830+t2381+t2498+t3556;
t5039 = t1538+t2023+t2677+t3950;
t5044 = -t1d.*(-t1904+t2396+t2517+t3579./2.0);
t5045 = t1491+t2457+t2860+t3551;
t5046 = t1531+t2423+t2825+t3577;
t5048 = -t37.*(-t1537+t1983+t3892+t18.*t37.*(t544-t1021+t330.*(t100-t364)));
t5049 = t1527+t2454+t2826+t3573;
t5050 = t1493+t2484+t2859+t3555;
t5052 = -t18.*t39.*(-t1537+t1983+t3892+t18.*t37.*(t544-t1021+t330.*(t100-t364)));
t5057 = t37.*(-t1537+t1983+t3892+t18.*t37.*(t544-t1021+t330.*(t100-t364))).*(-1.0./2.0);
t5059 = t1842+t2450+t2569+t3649;
t5062 = t18.*t39.*(-t1537+t1983+t3892+t18.*t37.*(t544-t1021+t330.*(t100-t364)));
t5069 = (t3687.*t4428)./2.0;
t5078 = (t4131.*t4155)./2.0;
t5096 = t8.*t5091;
t5097 = t5092./2.0;
t5099 = t1923+t2411+t2651+t3697;
t5102 = t14.*t39.*t5091;
t5103 = t612+t944+t1353+t1361+t1438+t1691+t2242+t2244;
t5108 = t1632+t2220+t2702+t4001;
t5111 = t1583+t2216+t2723+t4014;
t5112 = t1628+t2153+t2697+t4030;
t5118 = -t8.*(t1585+t2193-t4001+t38.*t39.*(t544-t1021+t330.*(t100-t364)));
t5120 = -t5116;
t5124 = t8.*(t1585+t2193-t4001+t38.*t39.*(t544-t1021+t330.*(t100-t364)));
t5126 = t5116./2.0;
t5130 = t255.*t5091;
t5132 = -t14.*t39.*(t1585+t2193-t4001+t38.*t39.*(t544-t1021+t330.*(t100-t364)));
t5133 = t1672+t2219+t2725+t4019;
t5137 = t5123./2.0;
t5138 = t646+t945+t1379+t1418+t2267+t2314+t2820;
t5144 = -t5136;
t5148 = t14.*t39.*(t1585+t2193-t4001+t38.*t39.*(t544-t1021+t330.*(t100-t364))).*(-1.0./2.0);
t5149 = t5136./2.0;
t5150 = -t8.*(t1631+t2701-t4019+t1553.*(t101-t401));
t5151 = -t5141;
t5155 = t5141./2.0;
t5158 = t8.*(t1631+t2701-t4019+t1553.*(t101-t401));
t5165 = t4155.*t4334;
t5166 = -t14.*t39.*(t1631+t2701-t4019+t1553.*(t101-t401));
t5167 = -t255.*(t1585+t2193-t4001+t38.*t39.*(t544-t1021+t330.*(t100-t364)));
t5170 = t14.*t39.*(t1631+t2701-t4019+t1553.*(t101-t401));
t5180 = t4050.*t4428;
t5181 = t255.*(t1585+t2193-t4001+t38.*t39.*(t544-t1021+t330.*(t100-t364))).*(-1.0./2.0);
t5182 = -t5175;
t5185 = (t255.*(t1585+t2193-t4001+t38.*t39.*(t544-t1021+t330.*(t100-t364))))./2.0;
t5186 = t5175./2.0;
t5188 = t5176./2.0;
t5200 = -t255.*(t1631+t2701-t4019+t1553.*(t101-t401));
t5201 = t255.*(t1631+t2701-t4019+t1553.*(t101-t401)).*(-1.0./2.0);
t5202 = t3479+t3480+t3481;
t5203 = t1158+t1182+t1252+t1255+t1476+t1483+t3993;
t5206 = t1152+t1181+t1250+t1251+t1473+t1486+t3993;
t5210 = t987+t2559+t2599+t2877+t2880;
t5211 = t725+t1465+t1844+t1960+t3011+t3029;
t5213 = -t6d.*(-t2559+t4330+(t255.*(t1155+t341.*(t101-t401)))./2.0+t402.*t593);
t5215 = t4155.*t4428;
t5224 = t5223.*t6d;
t5226 = t4334.*t4428;
t5229 = t691+t989+t1412+t1451+t1948+t1951+t2453+t2455;
t5256 = t1366+t1627+t1630+t2806+t3025+t3044;
t5257 = t2699+t2704+t3624+t3626;
t5259 = t37.*t5258;
t5260 = t18.*t39.*t5258;
t5267 = t1425+t1667+t1670+t2840+t3121+t3153;
t5269 = t2595+t2646+t3768+t3792;
t5279 = t2754+t3453+t3454+t3455;
t5280 = t14.*t5278;
t5286 = t8.*t5281;
t5287 = t8.*t39.*t5278;
t5289 = t2853+t2856+t3739+t3755;
t5290 = t2816+t2819+t3757+t3780;
t5295 = t14.*t39.*t5281;
t5296 = t14.*(t2853+t3739+t3755-t19.*t330.*(t544-t1021+t330.*(t100-t364)));
t5297 = t8.*(t2816+t3757+t3780-t19.*t255.*(t544-t1021+t330.*(t100-t364)));
t5305 = t330.*t5278;
t5306 = t255.*t5281;
t5312 = t549+t2760+t2761+t2762+t4294;
t5315 = t1873+t2282+t2283+t2355+t2471+t3579;
t5323 = -t1d.*(-t501+t4302+t2d.*(-t917+t979+(t14.*(t248-t484))./2.0)+t3d.*(-t917+t979+(t14.*(t248-t484))./2.0)+t4d.*(-t917+t979+(t14.*(t248-t484))./2.0));
t5324 = -t1d.*(t498-t4294+t2d.*(-t915+t978+(t8.*(t249-t483))./2.0)+t3d.*(-t915+t978+(t8.*(t249-t483))./2.0)+t4d.*(-t915+t978+(t8.*(t249-t483))./2.0));
t5327 = t2897+t2919+t3809+t3812;
t5328 = t4615+t4629;
t5348 = -t1d.*(-t245+t5d.*(-t221+t279-t671+t702+t1101+t2107+(t8.*t39.*(t206-t470))./2.0)+t2d.*(-t967+t1009+(t14.*(t206-t470))./2.0)+t3d.*(-t967+t1009+(t14.*(t206-t470))./2.0)+t4d.*(-t967+t1009+(t14.*(t206-t470))./2.0));
t5349 = t1d.*(-t245+t5d.*(-t221+t279-t671+t702+t1101+t2107+(t8.*t39.*(t206-t470))./2.0)+t2d.*(-t967+t1009+(t14.*(t206-t470))./2.0)+t3d.*(-t967+t1009+(t14.*(t206-t470))./2.0)+t4d.*(-t967+t1009+(t14.*(t206-t470))./2.0));
t5350 = t2327+t2388+t5036;
t5353 = t2838+t2917+t4023+t4038;
t5354 = -t37.*(t2878-t4023-t4038+t342.*(t544-t1021+t330.*(t100-t364)));
t5355 = -t18.*t39.*(t2878-t4023-t4038+t342.*(t544-t1021+t330.*(t100-t364)));
t5356 = t37.*(t2878-t4023-t4038+t342.*(t544-t1021+t330.*(t100-t364)));
t5359 = t18.*t39.*(t2878-t4023-t4038+t342.*(t544-t1021+t330.*(t100-t364))).*(-1.0./2.0);
t5368 = t2911+t2978+t4067+t4097;
t5370 = t2913+t2979+t4090+t4091;
t5372 = t667+t1125+t1191+t1369+t1480+t1698+t1879+t1941+t2910+t2948;
t5375 = -t5d.*(t633-t1879+t1911-t2910-t2948+t4018+(t37.*(t569-t604))./2.0);
t5397 = t3488+t3504+t4002+t4003;
t5400 = t4126+t4134+t4561;
t5409 = t4156+t4486+t4499;
t5413 = t4160+t4162+t4799;
t5438 = t3168+t3169+t5258;
t5464 = t4180+t4924+t4944;
t5478 = t5476.*t5d;
t5482 = t3568+t3606+t4801+t4802;
t5503 = t5501.*t4d;
t5505 = t3830+t3871+t4859+t4871;
t5514 = t5513.*t3d;
t5515 = t4086+t4112+t4859+t4871;
t5517 = t5516.*t2d;
t5523 = t4144+t4158+t4859+t4871;
t5619 = t3523+t4140+t4142+t4676+t4908+t4909;
t1526 = -t1513;
t1872 = -t1838;
t1885 = -t1850;
t2203 = t2176.*t1d;
t2205 = t2182.*t1d;
t2214 = t18.*t2191;
t2215 = -t2191;
Y = ft_9({t100,t1004,t1007,t101,t1015,t1016,t1017,t1021,t1026,t1028,t1031,t1035,t1036,t104,t1044,t1045,t1046,t1047,t1048,t1049,t1053,t1054,t1055,t106,t1066,t1068,t1069,t107,t1070,t1071,t1079,t108,t1080,t1081,t1082,t1083,t1084,t1085,t1086,t1087,t1093,t1094,t1096,t1097,t1098,t1106,t1108,t1109,t111,t1110,t112,t1121,t1122,t1123,t1126,t1128,t1129,t113,t1133,t1134,t1135,t1137,t1138,t1139,t1140,t1147,t1148,t1155,t1156,t1160,t1162,t1172,t1174,t1183,t1184,t1185,t1186,t1187,t1189,t1193,t1196,t12,t1203,t1208,t1209,t1210,t1211,t1222,t1224,t1225,t1226,t1227,t1230,t1236,t1237,t1238,t124,t1245,t1246,t1247,t1248,t1249,t1264,t1265,t1266,t1268,t127,t1271,t1272,t1273,t128,t1281,t1284,t1287,t1288,t1289,t1297,t1298,t13,t1302,t131,t1311,t1312,t1316,t1317,t132,t1321,t1328,t1331,t1332,t1333,t1334,t1335,t1336,t134,t1355,t1356,t1357,t1358,t136,t1368,t137,t1375,t1378,t138,t1382,t1392,t1395,t1397,t1399,t14,t1400,t1403,t1408,t1410,t1413,t1419,t1420,t1427,t1428,t1434,t1440,t1457,t1458,t1461,t1464,t1465,t1468,t1470,t1472,t1475,t1478,t1479,t1485,t1489,t1492,t1497,t1499,t15,t150,t1500,t1501,t1503,t1504,t1507,t1513,t1514,t1516,t1517,t1518,t1519,t152,t1520,t1521,t1525,t1526,t1528,t1529,t1532,t1534,t1535,t1536,t1537,t1547,t155,t156,t1569,t1571,t1572,t1574,t1578,t1579,t158,t1580,t1585,t1586,t1588,t1589,t159,t1590,t1597,t1599,t1606,t1607,t1609,t1610,t1615,t1617,t1618,t162,t163,t1636,t164,t1645,t1647,t1648,t1649,t165,t1650,t1651,t1652,t1653,t1654,t1659,t1660,t1663,t1671,t1674,t1677,t1678,t1680,t1682,t1683,t1685,t1686,t1687,t1692,t1699,t1701,t1704,t1706,t1707,t1709,t171,t1710,t1713,t1714,t1715,t1722,t1724,t173,t1733,t1736,t1738,t174,t1740,t1741,t1742,t1743,t1748,t175,t1751,t1754,t1755,t1758,t1759,t1760,t177,t1776,t1780,t1783,t1784,t1786,t1787,t1789,t1790,t1792,t1797,t1799,t18,t1800,t1803,t1807,t1813,t1814,t1815,t1816,t1818,t1827,t1829,t1832,t1833,t1835,t1836,t1837,t1838,t1840,t1844,t1846,t1848,t1849,t1862,t1863,t1864,t1866,t1867,t1868,t187,t1872,t1873,t1874,t1875,t1885,t1888,t1889,t1890,t1891,t1892,t1899,t19,t1900,t1901,t1903,t1904,t1905,t191,t1916,t1919,t1920,t1921,t1925,t1929,t1930,t1933,t1935,t1936,t1938,t1939,t1940,t1944,t1945,t1956,t1957,t1958,t1959,t1960,t1961,t1962,t1963,t1964,t1965,t1966,t1967,t1968,t1969,t1970,t1971,t1973,t1976,t1977,t1978,t1983,t1984,t1985,t1988,t199,t1992,t1993,t1995,t1996,t1999,t1d,t1dd,t200,t2001,t2002,t2004,t2005,t2009,t201,t2010,t2012,t2013,t2015,t2018,t2021,t2022,t2024,t2026,t2028,t2031,t2033,t2036,t2042,t2044,t2053,t2054,t2059,t206,t2060,t2061,t2062,t2068,t2070,t2072,t2074,t2075,t2079,t2080,t2081,t2085,t2086,t2087,t2088,t2090,t2093,t2098,t2099,t21,t2100,t2101,t2104,t2108,t2112,t2113,t2115,t2117,t2119,t2122,t2123,t2124,t2126,t2128,t2129,t2130,t2132,t2136,t2140,t2141,t2142,t2143,t2144,t2145,t2147,t215,t2150,t2155,t2156,t2159,t2160,t2162,t2167,t2168,t2169,t2170,t2171,t2173,t2174,t2178,t2180,t2184,t2186,t2187,t2188,t2189,t219,t2190,t2191,t2193,t2196,t2198,t22,t220,t2203,t2204,t2205,t2206,t2210,t2213,t2214,t2215,t2222,t2223,t2224,t2225,t2229,t2233,t2235,t2243,t2246,t2247,t2249,t2259,t226,t2266,t2269,t2270,t2279,t2281,t2286,t2289,t229,t2290,t2292,t2293,t2294,t2295,t2296,t23,t2300,t2304,t2305,t2306,t2308,t2310,t2311,t2317,t232,t2321,t2322,t2327,t2328,t2329,t233,t2330,t2331,t2332,t2339,t2340,t2344,t2346,t2348,t2349,t2351,t2352,t2353,t2354,t2355,t2356,t2357,t2358,t2359,t2361,t2363,t2364,t2366,t2367,t2368,t2369,t2371,t2372,t2373,t2374,t2375,t2376,t2378,t2379,t2380,t2382,t2384,t2385,t2386,t2387,t2393,t2395,t2398,t2399,t24,t2400,t2401,t2402,t2403,t2405,t2406,t2407,t2409,t2412,t2414,t2416,t2419,t2421,t2427,t2428,t2430,t2431,t2433,t2434,t2438,t244,t2445,t2446,t245,t2455,t2460,t2463,t2467,t247,t2471,t2472,t2473,t2475,t2476,t2477,t2478,t2479,t2486,t2488,t2490,t2491,t2492,t2493,t2497,t2499,t25,t2500,t2501,t2502,t2503,t2504,t2506,t2507,t2508,t2509,t2510,t2511,t2512,t2513,t2514,t2520,t2523,t2526,t2527,t2528,t2529,t2532,t2533,t2534,t2536,t2544,t2545,t2546,t2549,t255,t2550,t2552,t2557,t256,t2562,t2563,t2566,t2568,t2570,t2573,t2574,t2575,t2576,t2578,t2583,t2585,t2586,t2587,t2588,t2589,t2591,t2593,t2596,t26,t2602,t2604,t2605,t2606,t2608,t2610,t2614,t2617,t2619,t2625,t2626,t2627,t2630,t2640,t2641,t2642,t2644,t2645,t2647,t2648,t2652,t2654,t2655,t2658,t2659,t2661,t2664,t2665,t2666,t2673,t2675,t2678,t2679,t2681,t2682,t2689,t2690,t2691,t2696,t2699,t27,t2703,t2705,t2707,t2708,t2709,t2710,t2711,t2718,t2719,t2721,t2722,t2724,t2731,t2733,t2734,t2737,t2743,t2744,t2745,t2747,t2749,t2755,t2759,t2763,t2764,t2765,t2766,t2772,t2773,t2775,t2776,t2777,t2779,t2780,t2781,t2782,t2789,t2790,t2791,t2792,t2793,t2795,t2796,t2797,t2798,t2800,t2801,t2802,t2807,t2808,t2810,t2811,t2812,t2813,t2815,t2816,t2828,t2829,t2830,t2832,t2835,t2841,t2842,t2843,t2845,t2847,t2848,t2851,t2853,t2857,t2861,t2862,t2864,t2865,t2867,t2868,t2870,t2871,t2873,t2875,t2876,t2878,t2882,t2883,t2884,t2885,t2891,t2893,t2894,t2895,t2898,t2899,t29,t2900,t2901,t2902,t2914,t2915,t2918,t2925,t2926,t2927,t2929,t2930,t2933,t2934,t2935,t2936,t2937,t2940,t2946,t2947,t2950,t2951,t2953,t2954,t2956,t2957,t2959,t2961,t2966,t2967,t2968,t2970,t2971,t2972,t2981,t2982,t2983,t2985,t2988,t2989,t299,t2991,t2992,t2994,t2995,t2996,t2997,t2998,t2999,t2d,t2dd,t30,t3000,t3003,t3004,t3005,t3006,t3007,t3009,t301,t3010,t3011,t3012,t3013,t3014,t3017,t3018,t3028,t3029,t3032,t3035,t3037,t3043,t3048,t3050,t3052,t3057,t3058,t3059,t3065,t3066,t3069,t3073,t3075,t3076,t3078,t3079,t308,t3080,t3081,t3082,t3083,t3085,t3086,t3087,t3088,t3089,t3090,t3092,t3093,t3098,t3099,t31,t3100,t3101,t3104,t3106,t3107,t3108,t3112,t3113,t3115,t3120,t3123,t3124,t3125,t3126,t3129,t3130,t3135,t3136,t3137,t3138,t3139,t3140,t3141,t3142,t3143,t3146,t315,t3151,t3155,t3156,t3157,t3158,t3159,t3161,t3162,t3163,t3165,t3166,t317,t3170,t3171,t3172,t3173,t3174,t3175,t3176,t3177,t3179,t318,t3180,t3181,t3182,t3183,t3185,t3187,t319,t3191,t3192,t3193,t3195,t3196,t3197,t3200,t3204,t3205,t3206,t3212,t3213,t3214,t3215,t3219,t3220,t3221,t3226,t3228,t3230,t3231,t3232,t3234,t3236,t3237,t3239,t3240,t3241,t3243,t3244,t3246,t3247,t3249,t325,t3251,t3252,t3255,t3257,t3258,t3260,t3263,t3264,t3265,t3266,t3267,t3268,t3271,t3272,t3274,t3275,t3276,t3277,t3278,t3282,t3283,t3285,t3286,t3288,t3289,t329,t3290,t3291,t3292,t3298,t330,t3300,t3306,t3308,t3310,t3312,t3316,t3318,t332,t3321,t3322,t3325,t3326,t3327,t3328,t3329,t333,t3330,t3331,t3332,t3335,t3338,t3339,t3340,t3348,t3349,t3350,t3351,t3352,t3354,t3355,t3358,t3359,t3360,t3365,t3369,t3370,t3371,t3374,t3375,t3376,t3377,t3378,t3380,t3381,t3383,t3384,t3387,t3388,t3390,t3391,t3392,t3395,t3399,t34,t3400,t3401,t3404,t3405,t341,t3414,t3415,t3416,t3417,t342,t3421,t3426,t3429,t343,t3431,t3432,t3439,t3440,t3442,t3445,t3450,t3452,t3456,t3457,t3458,t3459,t346,t3460,t3461,t3468,t3469,t347,t3472,t3473,t3474,t3475,t3476,t3477,t3478,t3482,t3483,t3489,t3490,t3491,t3493,t3494,t3499,t3502,t3503,t3506,t3509,t3510,t3512,t3515,t3516,t3517,t3518,t3521,t3524,t3525,t3526,t3527,t3529,t3532,t3533,t3535,t3536,t3537,t3538,t3539,t3540,t3543,t3544,t3547,t3548,t3549,t3552,t3554,t3557,t3558,t3559,t3565,t3571,t3572,t3574,t3575,t3578,t3579,t3580,t3581,t3582,t3583,t3586,t3587,t3588,t3590,t3591,t3598,t36,t3600,t3601,t3602,t3603,t3604,t3605,t3607,t3608,t3609,t3610,t3611,t3613,t3617,t3619,t3620,t3621,t3622,t3623,t3624,t3625,t3628,t3630,t3631,t3632,t3633,t3634,t3635,t3636,t3637,t3638,t3639,t364,t3640,t3641,t3642,t3643,t3647,t3648,t365,t3650,t3651,t3653,t3655,t3662,t3665,t3666,t3667,t3668,t3669,t3670,t3671,t3673,t3679,t368,t3680,t3682,t3683,t3684,t3685,t3686,t3687,t3693,t3694,t3699,t37,t3701,t3702,t3708,t3709,t3710,t3712,t3715,t3716,t3719,t3732,t3734,t3739,t3741,t3745,t3747,t3749,t3750,t3751,t3754,t3755,t3756,t3757,t3762,t3770,t3771,t3772,t3780,t3781,t3785,t3787,t3788,t3789,t3795,t3799,t38,t3800,t3802,t3804,t3805,t3807,t3808,t3809,t3810,t3812,t3815,t3817,t3818,t3819,t3821,t3822,t3825,t3826,t3829,t3832,t3833,t3838,t3839,t3840,t3841,t3843,t3848,t3858,t3861,t3863,t3866,t3867,t3868,t3872,t3874,t3875,t3880,t3882,t3883,t3885,t3886,t3887,t3888,t3889,t3890,t3892,t3894,t3896,t3899,t39,t3900,t3901,t3903,t3904,t3908,t3912,t3913,t3917,t3919,t392,t3921,t3923,t3924,t3927,t3928,t393,t3931,t3932,t3933,t3934,t3935,t3936,t3937,t3938,t3942,t3943,t3944,t3956,t3958,t3960,t3962,t3964,t3965,t3966,t3967,t3969,t3971,t3972,t3975,t3976,t3977,t3978,t3979,t3982,t3984,t3986,t3989,t3990,t3991,t3992,t3994,t3997,t3999,t3d,t3dd,t4001,t4002,t4003,t4005,t4006,t4007,t4008,t4009,t401,t4010,t4011,t4012,t4016,t4017,t402,t4020,t4022,t4023,t4025,t4026,t4027,t403,t4034,t4036,t4038,t404,t4040,t4041,t4042,t4046,t4047,t4048,t4049,t4050,t4052,t4053,t4054,t4056,t4057,t4059,t4065,t4068,t4069,t4070,t4071,t4074,t4078,t4083,t4084,t4087,t4092,t4093,t4094,t4095,t4096,t41,t4101,t4102,t4108,t4115,t4117,t4118,t4121,t4122,t4125,t4127,t4128,t4130,t4131,t4133,t4136,t4137,t4139,t4143,t4146,t4147,t4149,t4151,t4152,t4154,t4155,t4156,t4157,t4159,t4161,t4163,t4164,t4166,t4167,t4168,t4170,t4171,t4172,t4174,t4176,t4178,t418,t4182,t4183,t4185,t4186,t4187,t4188,t4189,t419,t4190,t4191,t4192,t4193,t4195,t4196,t4197,t4198,t42,t420,t4200,t4201,t4203,t4204,t4206,t4212,t4213,t4214,t4218,t4221,t4223,t4224,t4226,t4227,t4228,t4229,t4230,t4231,t4233,t4235,t4236,t4237,t4238,t4241,t4242,t4243,t4246,t4249,t425,t4251,t4252,t4253,t4254,t4255,t4256,t4258,t4260,t4266,t4267,t4282,t4283,t4284,t4285,t4290,t4292,t4293,t4295,t4296,t4298,t4299,t4301,t4303,t4304,t4309,t431,t4311,t4312,t4317,t4319,t4321,t4324,t4325,t4327,t4328,t4330,t4331,t4332,t4333,t4335,t4336,t4337,t434,t4341,t4348,t4353,t4358,t4359,t4360,t4361,t4363,t4364,t4366,t4367,t437,t4371,t4372,t4388,t4394,t4395,t4396,t4399,t4402,t4403,t4404,t4406,t4407,t4408,t441,t4410,t4411,t4413,t442,t4420,t4421,t4423,t4424,t4427,t4428,t4429,t443,t4430,t4431,t4432,t4433,t4444,t4445,t4450,t4451,t4452,t4453,t4454,t4457,t4459,t446,t4460,t4461,t4464,t4467,t4468,t4470,t4473,t4474,t4475,t4476,t4479,t4480,t4483,t4487,t4488,t4491,t4493,t4494,t4500,t4503,t4506,t4508,t4509,t4514,t4515,t4517,t4519,t4526,t4528,t453,t4531,t4532,t4533,t4534,t4537,t4538,t4539,t454,t4540,t4541,t4542,t4543,t4546,t4547,t4548,t4550,t4551,t4552,t4553,t4556,t4561,t4562,t4565,t4568,t4572,t4575,t4576,t4578,t4579,t4582,t4583,t4587,t4588,t459,t4591,t4595,t4596,t4599,t4604,t4606,t4607,t4608,t4611,t4612,t4621,t4622,t4623,t4626,t4627,t4631,t4633,t4634,t4635,t4636,t4640,t4641,t4642,t4645,t4646,t4647,t4648,t4650,t4652,t4654,t4655,t4659,t4664,t4665,t4666,t4668,t4670,t4672,t4673,t4675,t4677,t4678,t4679,t4681,t4684,t4685,t4686,t4694,t4695,t4699,t470,t4700,t4701,t4702,t4703,t4704,t4705,t4707,t4708,t4710,t4713,t4714,t4715,t4716,t4717,t4720,t4721,t4722,t4723,t4724,t4725,t4727,t4730,t4732,t4737,t4738,t4739,t4741,t4744,t4747,t4757,t4758,t4759,t4760,t4762,t4765,t4766,t4767,t4768,t4770,t4771,t4776,t4777,t4778,t478,t4780,t4783,t4784,t4785,t4786,t4792,t4794,t4795,t4796,t4798,t48,t4807,t4810,t4813,t4815,t4817,t4822,t4825,t4828,t4829,t4830,t4831,t4836,t4837,t4838,t4840,t4841,t4843,t4845,t4846,t4849,t4851,t4855,t4856,t4858,t486,t4860,t4861,t4862,t4865,t4867,t487,t4870,t4873,t4874,t4875,t4878,t488,t4881,t4883,t4887,t4888,t4889,t4890,t4891,t4895,t4896,t4898,t4915,t4917,t492,t4920,t4922,t4923,t4925,t4926,t4929,t493,t4930,t4931,t4934,t4935,t4938,t494,t4941,t4942,t4943,t4946,t4949,t495,t4950,t4951,t4952,t4953,t4954,t4955,t4956,t4957,t4958,t4959,t496,t4960,t4967,t497,t4970,t4975,t4979,t4981,t4984,t4985,t4990,t4992,t4993,t4997,t4d,t4dd,t50,t5000,t5001,t5002,t5006,t501,t5010,t5011,t5012,t5013,t5014,t5018,t5019,t5020,t5022,t5025,t5026,t503,t5030,t5032,t5038,t5039,t5040,t5041,t5043,t5044,t5045,t5046,t5047,t5048,t5049,t5050,t5051,t5056,t5057,t5062,t5069,t5070,t5074,t5078,t508,t5081,t5092,t5093,t5096,t5097,t5098,t51,t5102,t5104,t5111,t5112,t5117,t5119,t5120,t5123,t5124,t5126,t5130,t5131,t5132,t5137,t5138,t514,t5144,t5148,t5149,t515,t5151,t5155,t5158,t516,t5163,t5165,t5167,t5170,t5171,t5175,t5176,t5180,t5181,t5182,t5185,t5186,t5188,t519,t5200,t5201,t5202,t5203,t5206,t5213,t5215,t5219,t5224,t5226,t523,t524,t5255,t5256,t5257,t5259,t5260,t5267,t5269,t5279,t5280,t5283,t5286,t5287,t529,t5292,t5295,t5296,t5297,t53,t530,t5305,t5306,t5315,t532,t5323,t5324,t5327,t5328,t5349,t5351,t5353,t5355,t5356,t5359,t5368,t537,t5370,t5375,t5397,t5401,t5403,t5413,t543,t5438,t544,t546,t5465,t547,t5478,t548,t5482,t55,t5503,t5505,t5514,t5515,t5517,t552,t5523,t553,t554,t56,t5619,t562,t569,t57,t570,t58,t582,t588,t589,t591,t593,t598,t5d,t5dd,t601,t602,t604,t608,t609,t61,t612,t614,t615,t616,t617,t623,t627,t63,t632,t634,t635,t637,t639,t641,t645,t646,t647,t648,t649,t650,t652,t653,t655,t659,t664,t670,t675,t680,t682,t687,t69,t694,t695,t696,t698,t699,t6d,t6dd,t703,t705,t706,t71,t711,t712,t713,t720,t721,t723,t726,t729,t731,t732,t733,t735,t736,t738,t739,t745,t746,t747,t748,t75,t752,t755,t759,t760,t761,t763,t764,t775,t776,t781,t785,t788,t789,t793,t8,t802,t806,t82,t820,t824,t828,t831,t832,t833,t838,t842,t843,t844,t846,t853,t855,t859,t861,t865,t870,t871,t873,t879,t880,t884,t885,t890,t892,t896,t897,t9,t900,t909,t910,t919,t922,t923,t927,t928,t930,t932,t937,t943,t944,t949,t952,t959,t961,t962,t963,t964,t965,t966,t969,t970,t972,t973,t981,t982,t983,t986,t989,t992,t999});
end
function Y = ft_9(ct)
t100 = ct{1};
t1004 = ct{2};
t1007 = ct{3};
t101 = ct{4};
t1015 = ct{5};
t1016 = ct{6};
t1017 = ct{7};
t1021 = ct{8};
t1026 = ct{9};
t1028 = ct{10};
t1031 = ct{11};
t1035 = ct{12};
t1036 = ct{13};
t104 = ct{14};
t1044 = ct{15};
t1045 = ct{16};
t1046 = ct{17};
t1047 = ct{18};
t1048 = ct{19};
t1049 = ct{20};
t1053 = ct{21};
t1054 = ct{22};
t1055 = ct{23};
t106 = ct{24};
t1066 = ct{25};
t1068 = ct{26};
t1069 = ct{27};
t107 = ct{28};
t1070 = ct{29};
t1071 = ct{30};
t1079 = ct{31};
t108 = ct{32};
t1080 = ct{33};
t1081 = ct{34};
t1082 = ct{35};
t1083 = ct{36};
t1084 = ct{37};
t1085 = ct{38};
t1086 = ct{39};
t1087 = ct{40};
t1093 = ct{41};
t1094 = ct{42};
t1096 = ct{43};
t1097 = ct{44};
t1098 = ct{45};
t1106 = ct{46};
t1108 = ct{47};
t1109 = ct{48};
t111 = ct{49};
t1110 = ct{50};
t112 = ct{51};
t1121 = ct{52};
t1122 = ct{53};
t1123 = ct{54};
t1126 = ct{55};
t1128 = ct{56};
t1129 = ct{57};
t113 = ct{58};
t1133 = ct{59};
t1134 = ct{60};
t1135 = ct{61};
t1137 = ct{62};
t1138 = ct{63};
t1139 = ct{64};
t1140 = ct{65};
t1147 = ct{66};
t1148 = ct{67};
t1155 = ct{68};
t1156 = ct{69};
t1160 = ct{70};
t1162 = ct{71};
t1172 = ct{72};
t1174 = ct{73};
t1183 = ct{74};
t1184 = ct{75};
t1185 = ct{76};
t1186 = ct{77};
t1187 = ct{78};
t1189 = ct{79};
t1193 = ct{80};
t1196 = ct{81};
t12 = ct{82};
t1203 = ct{83};
t1208 = ct{84};
t1209 = ct{85};
t1210 = ct{86};
t1211 = ct{87};
t1222 = ct{88};
t1224 = ct{89};
t1225 = ct{90};
t1226 = ct{91};
t1227 = ct{92};
t1230 = ct{93};
t1236 = ct{94};
t1237 = ct{95};
t1238 = ct{96};
t124 = ct{97};
t1245 = ct{98};
t1246 = ct{99};
t1247 = ct{100};
t1248 = ct{101};
t1249 = ct{102};
t1264 = ct{103};
t1265 = ct{104};
t1266 = ct{105};
t1268 = ct{106};
t127 = ct{107};
t1271 = ct{108};
t1272 = ct{109};
t1273 = ct{110};
t128 = ct{111};
t1281 = ct{112};
t1284 = ct{113};
t1287 = ct{114};
t1288 = ct{115};
t1289 = ct{116};
t1297 = ct{117};
t1298 = ct{118};
t13 = ct{119};
t1302 = ct{120};
t131 = ct{121};
t1311 = ct{122};
t1312 = ct{123};
t1316 = ct{124};
t1317 = ct{125};
t132 = ct{126};
t1321 = ct{127};
t1328 = ct{128};
t1331 = ct{129};
t1332 = ct{130};
t1333 = ct{131};
t1334 = ct{132};
t1335 = ct{133};
t1336 = ct{134};
t134 = ct{135};
t1355 = ct{136};
t1356 = ct{137};
t1357 = ct{138};
t1358 = ct{139};
t136 = ct{140};
t1368 = ct{141};
t137 = ct{142};
t1375 = ct{143};
t1378 = ct{144};
t138 = ct{145};
t1382 = ct{146};
t1392 = ct{147};
t1395 = ct{148};
t1397 = ct{149};
t1399 = ct{150};
t14 = ct{151};
t1400 = ct{152};
t1403 = ct{153};
t1408 = ct{154};
t1410 = ct{155};
t1413 = ct{156};
t1419 = ct{157};
t1420 = ct{158};
t1427 = ct{159};
t1428 = ct{160};
t1434 = ct{161};
t1440 = ct{162};
t1457 = ct{163};
t1458 = ct{164};
t1461 = ct{165};
t1464 = ct{166};
t1465 = ct{167};
t1468 = ct{168};
t1470 = ct{169};
t1472 = ct{170};
t1475 = ct{171};
t1478 = ct{172};
t1479 = ct{173};
t1485 = ct{174};
t1489 = ct{175};
t1492 = ct{176};
t1497 = ct{177};
t1499 = ct{178};
t15 = ct{179};
t150 = ct{180};
t1500 = ct{181};
t1501 = ct{182};
t1503 = ct{183};
t1504 = ct{184};
t1507 = ct{185};
t1513 = ct{186};
t1514 = ct{187};
t1516 = ct{188};
t1517 = ct{189};
t1518 = ct{190};
t1519 = ct{191};
t152 = ct{192};
t1520 = ct{193};
t1521 = ct{194};
t1525 = ct{195};
t1526 = ct{196};
t1528 = ct{197};
t1529 = ct{198};
t1532 = ct{199};
t1534 = ct{200};
t1535 = ct{201};
t1536 = ct{202};
t1537 = ct{203};
t1547 = ct{204};
t155 = ct{205};
t156 = ct{206};
t1569 = ct{207};
t1571 = ct{208};
t1572 = ct{209};
t1574 = ct{210};
t1578 = ct{211};
t1579 = ct{212};
t158 = ct{213};
t1580 = ct{214};
t1585 = ct{215};
t1586 = ct{216};
t1588 = ct{217};
t1589 = ct{218};
t159 = ct{219};
t1590 = ct{220};
t1597 = ct{221};
t1599 = ct{222};
t1606 = ct{223};
t1607 = ct{224};
t1609 = ct{225};
t1610 = ct{226};
t1615 = ct{227};
t1617 = ct{228};
t1618 = ct{229};
t162 = ct{230};
t163 = ct{231};
t1636 = ct{232};
t164 = ct{233};
t1645 = ct{234};
t1647 = ct{235};
t1648 = ct{236};
t1649 = ct{237};
t165 = ct{238};
t1650 = ct{239};
t1651 = ct{240};
t1652 = ct{241};
t1653 = ct{242};
t1654 = ct{243};
t1659 = ct{244};
t1660 = ct{245};
t1663 = ct{246};
t1671 = ct{247};
t1674 = ct{248};
t1677 = ct{249};
t1678 = ct{250};
t1680 = ct{251};
t1682 = ct{252};
t1683 = ct{253};
t1685 = ct{254};
t1686 = ct{255};
t1687 = ct{256};
t1692 = ct{257};
t1699 = ct{258};
t1701 = ct{259};
t1704 = ct{260};
t1706 = ct{261};
t1707 = ct{262};
t1709 = ct{263};
t171 = ct{264};
t1710 = ct{265};
t1713 = ct{266};
t1714 = ct{267};
t1715 = ct{268};
t1722 = ct{269};
t1724 = ct{270};
t173 = ct{271};
t1733 = ct{272};
t1736 = ct{273};
t1738 = ct{274};
t174 = ct{275};
t1740 = ct{276};
t1741 = ct{277};
t1742 = ct{278};
t1743 = ct{279};
t1748 = ct{280};
t175 = ct{281};
t1751 = ct{282};
t1754 = ct{283};
t1755 = ct{284};
t1758 = ct{285};
t1759 = ct{286};
t1760 = ct{287};
t177 = ct{288};
t1776 = ct{289};
t1780 = ct{290};
t1783 = ct{291};
t1784 = ct{292};
t1786 = ct{293};
t1787 = ct{294};
t1789 = ct{295};
t1790 = ct{296};
t1792 = ct{297};
t1797 = ct{298};
t1799 = ct{299};
t18 = ct{300};
t1800 = ct{301};
t1803 = ct{302};
t1807 = ct{303};
t1813 = ct{304};
t1814 = ct{305};
t1815 = ct{306};
t1816 = ct{307};
t1818 = ct{308};
t1827 = ct{309};
t1829 = ct{310};
t1832 = ct{311};
t1833 = ct{312};
t1835 = ct{313};
t1836 = ct{314};
t1837 = ct{315};
t1838 = ct{316};
t1840 = ct{317};
t1844 = ct{318};
t1846 = ct{319};
t1848 = ct{320};
t1849 = ct{321};
t1862 = ct{322};
t1863 = ct{323};
t1864 = ct{324};
t1866 = ct{325};
t1867 = ct{326};
t1868 = ct{327};
t187 = ct{328};
t1872 = ct{329};
t1873 = ct{330};
t1874 = ct{331};
t1875 = ct{332};
t1885 = ct{333};
t1888 = ct{334};
t1889 = ct{335};
t1890 = ct{336};
t1891 = ct{337};
t1892 = ct{338};
t1899 = ct{339};
t19 = ct{340};
t1900 = ct{341};
t1901 = ct{342};
t1903 = ct{343};
t1904 = ct{344};
t1905 = ct{345};
t191 = ct{346};
t1916 = ct{347};
t1919 = ct{348};
t1920 = ct{349};
t1921 = ct{350};
t1925 = ct{351};
t1929 = ct{352};
t1930 = ct{353};
t1933 = ct{354};
t1935 = ct{355};
t1936 = ct{356};
t1938 = ct{357};
t1939 = ct{358};
t1940 = ct{359};
t1944 = ct{360};
t1945 = ct{361};
t1956 = ct{362};
t1957 = ct{363};
t1958 = ct{364};
t1959 = ct{365};
t1960 = ct{366};
t1961 = ct{367};
t1962 = ct{368};
t1963 = ct{369};
t1964 = ct{370};
t1965 = ct{371};
t1966 = ct{372};
t1967 = ct{373};
t1968 = ct{374};
t1969 = ct{375};
t1970 = ct{376};
t1971 = ct{377};
t1973 = ct{378};
t1976 = ct{379};
t1977 = ct{380};
t1978 = ct{381};
t1983 = ct{382};
t1984 = ct{383};
t1985 = ct{384};
t1988 = ct{385};
t199 = ct{386};
t1992 = ct{387};
t1993 = ct{388};
t1995 = ct{389};
t1996 = ct{390};
t1999 = ct{391};
t1d = ct{392};
t1dd = ct{393};
t200 = ct{394};
t2001 = ct{395};
t2002 = ct{396};
t2004 = ct{397};
t2005 = ct{398};
t2009 = ct{399};
t201 = ct{400};
t2010 = ct{401};
t2012 = ct{402};
t2013 = ct{403};
t2015 = ct{404};
t2018 = ct{405};
t2021 = ct{406};
t2022 = ct{407};
t2024 = ct{408};
t2026 = ct{409};
t2028 = ct{410};
t2031 = ct{411};
t2033 = ct{412};
t2036 = ct{413};
t2042 = ct{414};
t2044 = ct{415};
t2053 = ct{416};
t2054 = ct{417};
t2059 = ct{418};
t206 = ct{419};
t2060 = ct{420};
t2061 = ct{421};
t2062 = ct{422};
t2068 = ct{423};
t2070 = ct{424};
t2072 = ct{425};
t2074 = ct{426};
t2075 = ct{427};
t2079 = ct{428};
t2080 = ct{429};
t2081 = ct{430};
t2085 = ct{431};
t2086 = ct{432};
t2087 = ct{433};
t2088 = ct{434};
t2090 = ct{435};
t2093 = ct{436};
t2098 = ct{437};
t2099 = ct{438};
t21 = ct{439};
t2100 = ct{440};
t2101 = ct{441};
t2104 = ct{442};
t2108 = ct{443};
t2112 = ct{444};
t2113 = ct{445};
t2115 = ct{446};
t2117 = ct{447};
t2119 = ct{448};
t2122 = ct{449};
t2123 = ct{450};
t2124 = ct{451};
t2126 = ct{452};
t2128 = ct{453};
t2129 = ct{454};
t2130 = ct{455};
t2132 = ct{456};
t2136 = ct{457};
t2140 = ct{458};
t2141 = ct{459};
t2142 = ct{460};
t2143 = ct{461};
t2144 = ct{462};
t2145 = ct{463};
t2147 = ct{464};
t215 = ct{465};
t2150 = ct{466};
t2155 = ct{467};
t2156 = ct{468};
t2159 = ct{469};
t2160 = ct{470};
t2162 = ct{471};
t2167 = ct{472};
t2168 = ct{473};
t2169 = ct{474};
t2170 = ct{475};
t2171 = ct{476};
t2173 = ct{477};
t2174 = ct{478};
t2178 = ct{479};
t2180 = ct{480};
t2184 = ct{481};
t2186 = ct{482};
t2187 = ct{483};
t2188 = ct{484};
t2189 = ct{485};
t219 = ct{486};
t2190 = ct{487};
t2191 = ct{488};
t2193 = ct{489};
t2196 = ct{490};
t2198 = ct{491};
t22 = ct{492};
t220 = ct{493};
t2203 = ct{494};
t2204 = ct{495};
t2205 = ct{496};
t2206 = ct{497};
t2210 = ct{498};
t2213 = ct{499};
t2214 = ct{500};
t2215 = ct{501};
t2222 = ct{502};
t2223 = ct{503};
t2224 = ct{504};
t2225 = ct{505};
t2229 = ct{506};
t2233 = ct{507};
t2235 = ct{508};
t2243 = ct{509};
t2246 = ct{510};
t2247 = ct{511};
t2249 = ct{512};
t2259 = ct{513};
t226 = ct{514};
t2266 = ct{515};
t2269 = ct{516};
t2270 = ct{517};
t2279 = ct{518};
t2281 = ct{519};
t2286 = ct{520};
t2289 = ct{521};
t229 = ct{522};
t2290 = ct{523};
t2292 = ct{524};
t2293 = ct{525};
t2294 = ct{526};
t2295 = ct{527};
t2296 = ct{528};
t23 = ct{529};
t2300 = ct{530};
t2304 = ct{531};
t2305 = ct{532};
t2306 = ct{533};
t2308 = ct{534};
t2310 = ct{535};
t2311 = ct{536};
t2317 = ct{537};
t232 = ct{538};
t2321 = ct{539};
t2322 = ct{540};
t2327 = ct{541};
t2328 = ct{542};
t2329 = ct{543};
t233 = ct{544};
t2330 = ct{545};
t2331 = ct{546};
t2332 = ct{547};
t2339 = ct{548};
t2340 = ct{549};
t2344 = ct{550};
t2346 = ct{551};
t2348 = ct{552};
t2349 = ct{553};
t2351 = ct{554};
t2352 = ct{555};
t2353 = ct{556};
t2354 = ct{557};
t2355 = ct{558};
t2356 = ct{559};
t2357 = ct{560};
t2358 = ct{561};
t2359 = ct{562};
t2361 = ct{563};
t2363 = ct{564};
t2364 = ct{565};
t2366 = ct{566};
t2367 = ct{567};
t2368 = ct{568};
t2369 = ct{569};
t2371 = ct{570};
t2372 = ct{571};
t2373 = ct{572};
t2374 = ct{573};
t2375 = ct{574};
t2376 = ct{575};
t2378 = ct{576};
t2379 = ct{577};
t2380 = ct{578};
t2382 = ct{579};
t2384 = ct{580};
t2385 = ct{581};
t2386 = ct{582};
t2387 = ct{583};
t2393 = ct{584};
t2395 = ct{585};
t2398 = ct{586};
t2399 = ct{587};
t24 = ct{588};
t2400 = ct{589};
t2401 = ct{590};
t2402 = ct{591};
t2403 = ct{592};
t2405 = ct{593};
t2406 = ct{594};
t2407 = ct{595};
t2409 = ct{596};
t2412 = ct{597};
t2414 = ct{598};
t2416 = ct{599};
t2419 = ct{600};
t2421 = ct{601};
t2427 = ct{602};
t2428 = ct{603};
t2430 = ct{604};
t2431 = ct{605};
t2433 = ct{606};
t2434 = ct{607};
t2438 = ct{608};
t244 = ct{609};
t2445 = ct{610};
t2446 = ct{611};
t245 = ct{612};
t2455 = ct{613};
t2460 = ct{614};
t2463 = ct{615};
t2467 = ct{616};
t247 = ct{617};
t2471 = ct{618};
t2472 = ct{619};
t2473 = ct{620};
t2475 = ct{621};
t2476 = ct{622};
t2477 = ct{623};
t2478 = ct{624};
t2479 = ct{625};
t2486 = ct{626};
t2488 = ct{627};
t2490 = ct{628};
t2491 = ct{629};
t2492 = ct{630};
t2493 = ct{631};
t2497 = ct{632};
t2499 = ct{633};
t25 = ct{634};
t2500 = ct{635};
t2501 = ct{636};
t2502 = ct{637};
t2503 = ct{638};
t2504 = ct{639};
t2506 = ct{640};
t2507 = ct{641};
t2508 = ct{642};
t2509 = ct{643};
t2510 = ct{644};
t2511 = ct{645};
t2512 = ct{646};
t2513 = ct{647};
t2514 = ct{648};
t2520 = ct{649};
t2523 = ct{650};
t2526 = ct{651};
t2527 = ct{652};
t2528 = ct{653};
t2529 = ct{654};
t2532 = ct{655};
t2533 = ct{656};
t2534 = ct{657};
t2536 = ct{658};
t2544 = ct{659};
t2545 = ct{660};
t2546 = ct{661};
t2549 = ct{662};
t255 = ct{663};
t2550 = ct{664};
t2552 = ct{665};
t2557 = ct{666};
t256 = ct{667};
t2562 = ct{668};
t2563 = ct{669};
t2566 = ct{670};
t2568 = ct{671};
t2570 = ct{672};
t2573 = ct{673};
t2574 = ct{674};
t2575 = ct{675};
t2576 = ct{676};
t2578 = ct{677};
t2583 = ct{678};
t2585 = ct{679};
t2586 = ct{680};
t2587 = ct{681};
t2588 = ct{682};
t2589 = ct{683};
t2591 = ct{684};
t2593 = ct{685};
t2596 = ct{686};
t26 = ct{687};
t2602 = ct{688};
t2604 = ct{689};
t2605 = ct{690};
t2606 = ct{691};
t2608 = ct{692};
t2610 = ct{693};
t2614 = ct{694};
t2617 = ct{695};
t2619 = ct{696};
t2625 = ct{697};
t2626 = ct{698};
t2627 = ct{699};
t2630 = ct{700};
t2640 = ct{701};
t2641 = ct{702};
t2642 = ct{703};
t2644 = ct{704};
t2645 = ct{705};
t2647 = ct{706};
t2648 = ct{707};
t2652 = ct{708};
t2654 = ct{709};
t2655 = ct{710};
t2658 = ct{711};
t2659 = ct{712};
t2661 = ct{713};
t2664 = ct{714};
t2665 = ct{715};
t2666 = ct{716};
t2673 = ct{717};
t2675 = ct{718};
t2678 = ct{719};
t2679 = ct{720};
t2681 = ct{721};
t2682 = ct{722};
t2689 = ct{723};
t2690 = ct{724};
t2691 = ct{725};
t2696 = ct{726};
t2699 = ct{727};
t27 = ct{728};
t2703 = ct{729};
t2705 = ct{730};
t2707 = ct{731};
t2708 = ct{732};
t2709 = ct{733};
t2710 = ct{734};
t2711 = ct{735};
t2718 = ct{736};
t2719 = ct{737};
t2721 = ct{738};
t2722 = ct{739};
t2724 = ct{740};
t2731 = ct{741};
t2733 = ct{742};
t2734 = ct{743};
t2737 = ct{744};
t2743 = ct{745};
t2744 = ct{746};
t2745 = ct{747};
t2747 = ct{748};
t2749 = ct{749};
t2755 = ct{750};
t2759 = ct{751};
t2763 = ct{752};
t2764 = ct{753};
t2765 = ct{754};
t2766 = ct{755};
t2772 = ct{756};
t2773 = ct{757};
t2775 = ct{758};
t2776 = ct{759};
t2777 = ct{760};
t2779 = ct{761};
t2780 = ct{762};
t2781 = ct{763};
t2782 = ct{764};
t2789 = ct{765};
t2790 = ct{766};
t2791 = ct{767};
t2792 = ct{768};
t2793 = ct{769};
t2795 = ct{770};
t2796 = ct{771};
t2797 = ct{772};
t2798 = ct{773};
t2800 = ct{774};
t2801 = ct{775};
t2802 = ct{776};
t2807 = ct{777};
t2808 = ct{778};
t2810 = ct{779};
t2811 = ct{780};
t2812 = ct{781};
t2813 = ct{782};
t2815 = ct{783};
t2816 = ct{784};
t2828 = ct{785};
t2829 = ct{786};
t2830 = ct{787};
t2832 = ct{788};
t2835 = ct{789};
t2841 = ct{790};
t2842 = ct{791};
t2843 = ct{792};
t2845 = ct{793};
t2847 = ct{794};
t2848 = ct{795};
t2851 = ct{796};
t2853 = ct{797};
t2857 = ct{798};
t2861 = ct{799};
t2862 = ct{800};
t2864 = ct{801};
t2865 = ct{802};
t2867 = ct{803};
t2868 = ct{804};
t2870 = ct{805};
t2871 = ct{806};
t2873 = ct{807};
t2875 = ct{808};
t2876 = ct{809};
t2878 = ct{810};
t2882 = ct{811};
t2883 = ct{812};
t2884 = ct{813};
t2885 = ct{814};
t2891 = ct{815};
t2893 = ct{816};
t2894 = ct{817};
t2895 = ct{818};
t2898 = ct{819};
t2899 = ct{820};
t29 = ct{821};
t2900 = ct{822};
t2901 = ct{823};
t2902 = ct{824};
t2914 = ct{825};
t2915 = ct{826};
t2918 = ct{827};
t2925 = ct{828};
t2926 = ct{829};
t2927 = ct{830};
t2929 = ct{831};
t2930 = ct{832};
t2933 = ct{833};
t2934 = ct{834};
t2935 = ct{835};
t2936 = ct{836};
t2937 = ct{837};
t2940 = ct{838};
t2946 = ct{839};
t2947 = ct{840};
t2950 = ct{841};
t2951 = ct{842};
t2953 = ct{843};
t2954 = ct{844};
t2956 = ct{845};
t2957 = ct{846};
t2959 = ct{847};
t2961 = ct{848};
t2966 = ct{849};
t2967 = ct{850};
t2968 = ct{851};
t2970 = ct{852};
t2971 = ct{853};
t2972 = ct{854};
t2981 = ct{855};
t2982 = ct{856};
t2983 = ct{857};
t2985 = ct{858};
t2988 = ct{859};
t2989 = ct{860};
t299 = ct{861};
t2991 = ct{862};
t2992 = ct{863};
t2994 = ct{864};
t2995 = ct{865};
t2996 = ct{866};
t2997 = ct{867};
t2998 = ct{868};
t2999 = ct{869};
t2d = ct{870};
t2dd = ct{871};
t30 = ct{872};
t3000 = ct{873};
t3003 = ct{874};
t3004 = ct{875};
t3005 = ct{876};
t3006 = ct{877};
t3007 = ct{878};
t3009 = ct{879};
t301 = ct{880};
t3010 = ct{881};
t3011 = ct{882};
t3012 = ct{883};
t3013 = ct{884};
t3014 = ct{885};
t3017 = ct{886};
t3018 = ct{887};
t3028 = ct{888};
t3029 = ct{889};
t3032 = ct{890};
t3035 = ct{891};
t3037 = ct{892};
t3043 = ct{893};
t3048 = ct{894};
t3050 = ct{895};
t3052 = ct{896};
t3057 = ct{897};
t3058 = ct{898};
t3059 = ct{899};
t3065 = ct{900};
t3066 = ct{901};
t3069 = ct{902};
t3073 = ct{903};
t3075 = ct{904};
t3076 = ct{905};
t3078 = ct{906};
t3079 = ct{907};
t308 = ct{908};
t3080 = ct{909};
t3081 = ct{910};
t3082 = ct{911};
t3083 = ct{912};
t3085 = ct{913};
t3086 = ct{914};
t3087 = ct{915};
t3088 = ct{916};
t3089 = ct{917};
t3090 = ct{918};
t3092 = ct{919};
t3093 = ct{920};
t3098 = ct{921};
t3099 = ct{922};
t31 = ct{923};
t3100 = ct{924};
t3101 = ct{925};
t3104 = ct{926};
t3106 = ct{927};
t3107 = ct{928};
t3108 = ct{929};
t3112 = ct{930};
t3113 = ct{931};
t3115 = ct{932};
t3120 = ct{933};
t3123 = ct{934};
t3124 = ct{935};
t3125 = ct{936};
t3126 = ct{937};
t3129 = ct{938};
t3130 = ct{939};
t3135 = ct{940};
t3136 = ct{941};
t3137 = ct{942};
t3138 = ct{943};
t3139 = ct{944};
t3140 = ct{945};
t3141 = ct{946};
t3142 = ct{947};
t3143 = ct{948};
t3146 = ct{949};
t315 = ct{950};
t3151 = ct{951};
t3155 = ct{952};
t3156 = ct{953};
t3157 = ct{954};
t3158 = ct{955};
t3159 = ct{956};
t3161 = ct{957};
t3162 = ct{958};
t3163 = ct{959};
t3165 = ct{960};
t3166 = ct{961};
t317 = ct{962};
t3170 = ct{963};
t3171 = ct{964};
t3172 = ct{965};
t3173 = ct{966};
t3174 = ct{967};
t3175 = ct{968};
t3176 = ct{969};
t3177 = ct{970};
t3179 = ct{971};
t318 = ct{972};
t3180 = ct{973};
t3181 = ct{974};
t3182 = ct{975};
t3183 = ct{976};
t3185 = ct{977};
t3187 = ct{978};
t319 = ct{979};
t3191 = ct{980};
t3192 = ct{981};
t3193 = ct{982};
t3195 = ct{983};
t3196 = ct{984};
t3197 = ct{985};
t3200 = ct{986};
t3204 = ct{987};
t3205 = ct{988};
t3206 = ct{989};
t3212 = ct{990};
t3213 = ct{991};
t3214 = ct{992};
t3215 = ct{993};
t3219 = ct{994};
t3220 = ct{995};
t3221 = ct{996};
t3226 = ct{997};
t3228 = ct{998};
t3230 = ct{999};
t3231 = ct{1000};
t3232 = ct{1001};
t3234 = ct{1002};
t3236 = ct{1003};
t3237 = ct{1004};
t3239 = ct{1005};
t3240 = ct{1006};
t3241 = ct{1007};
t3243 = ct{1008};
t3244 = ct{1009};
t3246 = ct{1010};
t3247 = ct{1011};
t3249 = ct{1012};
t325 = ct{1013};
t3251 = ct{1014};
t3252 = ct{1015};
t3255 = ct{1016};
t3257 = ct{1017};
t3258 = ct{1018};
t3260 = ct{1019};
t3263 = ct{1020};
t3264 = ct{1021};
t3265 = ct{1022};
t3266 = ct{1023};
t3267 = ct{1024};
t3268 = ct{1025};
t3271 = ct{1026};
t3272 = ct{1027};
t3274 = ct{1028};
t3275 = ct{1029};
t3276 = ct{1030};
t3277 = ct{1031};
t3278 = ct{1032};
t3282 = ct{1033};
t3283 = ct{1034};
t3285 = ct{1035};
t3286 = ct{1036};
t3288 = ct{1037};
t3289 = ct{1038};
t329 = ct{1039};
t3290 = ct{1040};
t3291 = ct{1041};
t3292 = ct{1042};
t3298 = ct{1043};
t330 = ct{1044};
t3300 = ct{1045};
t3306 = ct{1046};
t3308 = ct{1047};
t3310 = ct{1048};
t3312 = ct{1049};
t3316 = ct{1050};
t3318 = ct{1051};
t332 = ct{1052};
t3321 = ct{1053};
t3322 = ct{1054};
t3325 = ct{1055};
t3326 = ct{1056};
t3327 = ct{1057};
t3328 = ct{1058};
t3329 = ct{1059};
t333 = ct{1060};
t3330 = ct{1061};
t3331 = ct{1062};
t3332 = ct{1063};
t3335 = ct{1064};
t3338 = ct{1065};
t3339 = ct{1066};
t3340 = ct{1067};
t3348 = ct{1068};
t3349 = ct{1069};
t3350 = ct{1070};
t3351 = ct{1071};
t3352 = ct{1072};
t3354 = ct{1073};
t3355 = ct{1074};
t3358 = ct{1075};
t3359 = ct{1076};
t3360 = ct{1077};
t3365 = ct{1078};
t3369 = ct{1079};
t3370 = ct{1080};
t3371 = ct{1081};
t3374 = ct{1082};
t3375 = ct{1083};
t3376 = ct{1084};
t3377 = ct{1085};
t3378 = ct{1086};
t3380 = ct{1087};
t3381 = ct{1088};
t3383 = ct{1089};
t3384 = ct{1090};
t3387 = ct{1091};
t3388 = ct{1092};
t3390 = ct{1093};
t3391 = ct{1094};
t3392 = ct{1095};
t3395 = ct{1096};
t3399 = ct{1097};
t34 = ct{1098};
t3400 = ct{1099};
t3401 = ct{1100};
t3404 = ct{1101};
t3405 = ct{1102};
t341 = ct{1103};
t3414 = ct{1104};
t3415 = ct{1105};
t3416 = ct{1106};
t3417 = ct{1107};
t342 = ct{1108};
t3421 = ct{1109};
t3426 = ct{1110};
t3429 = ct{1111};
t343 = ct{1112};
t3431 = ct{1113};
t3432 = ct{1114};
t3439 = ct{1115};
t3440 = ct{1116};
t3442 = ct{1117};
t3445 = ct{1118};
t3450 = ct{1119};
t3452 = ct{1120};
t3456 = ct{1121};
t3457 = ct{1122};
t3458 = ct{1123};
t3459 = ct{1124};
t346 = ct{1125};
t3460 = ct{1126};
t3461 = ct{1127};
t3468 = ct{1128};
t3469 = ct{1129};
t347 = ct{1130};
t3472 = ct{1131};
t3473 = ct{1132};
t3474 = ct{1133};
t3475 = ct{1134};
t3476 = ct{1135};
t3477 = ct{1136};
t3478 = ct{1137};
t3482 = ct{1138};
t3483 = ct{1139};
t3489 = ct{1140};
t3490 = ct{1141};
t3491 = ct{1142};
t3493 = ct{1143};
t3494 = ct{1144};
t3499 = ct{1145};
t3502 = ct{1146};
t3503 = ct{1147};
t3506 = ct{1148};
t3509 = ct{1149};
t3510 = ct{1150};
t3512 = ct{1151};
t3515 = ct{1152};
t3516 = ct{1153};
t3517 = ct{1154};
t3518 = ct{1155};
t3521 = ct{1156};
t3524 = ct{1157};
t3525 = ct{1158};
t3526 = ct{1159};
t3527 = ct{1160};
t3529 = ct{1161};
t3532 = ct{1162};
t3533 = ct{1163};
t3535 = ct{1164};
t3536 = ct{1165};
t3537 = ct{1166};
t3538 = ct{1167};
t3539 = ct{1168};
t3540 = ct{1169};
t3543 = ct{1170};
t3544 = ct{1171};
t3547 = ct{1172};
t3548 = ct{1173};
t3549 = ct{1174};
t3552 = ct{1175};
t3554 = ct{1176};
t3557 = ct{1177};
t3558 = ct{1178};
t3559 = ct{1179};
t3565 = ct{1180};
t3571 = ct{1181};
t3572 = ct{1182};
t3574 = ct{1183};
t3575 = ct{1184};
t3578 = ct{1185};
t3579 = ct{1186};
t3580 = ct{1187};
t3581 = ct{1188};
t3582 = ct{1189};
t3583 = ct{1190};
t3586 = ct{1191};
t3587 = ct{1192};
t3588 = ct{1193};
t3590 = ct{1194};
t3591 = ct{1195};
t3598 = ct{1196};
t36 = ct{1197};
t3600 = ct{1198};
t3601 = ct{1199};
t3602 = ct{1200};
t3603 = ct{1201};
t3604 = ct{1202};
t3605 = ct{1203};
t3607 = ct{1204};
t3608 = ct{1205};
t3609 = ct{1206};
t3610 = ct{1207};
t3611 = ct{1208};
t3613 = ct{1209};
t3617 = ct{1210};
t3619 = ct{1211};
t3620 = ct{1212};
t3621 = ct{1213};
t3622 = ct{1214};
t3623 = ct{1215};
t3624 = ct{1216};
t3625 = ct{1217};
t3628 = ct{1218};
t3630 = ct{1219};
t3631 = ct{1220};
t3632 = ct{1221};
t3633 = ct{1222};
t3634 = ct{1223};
t3635 = ct{1224};
t3636 = ct{1225};
t3637 = ct{1226};
t3638 = ct{1227};
t3639 = ct{1228};
t364 = ct{1229};
t3640 = ct{1230};
t3641 = ct{1231};
t3642 = ct{1232};
t3643 = ct{1233};
t3647 = ct{1234};
t3648 = ct{1235};
t365 = ct{1236};
t3650 = ct{1237};
t3651 = ct{1238};
t3653 = ct{1239};
t3655 = ct{1240};
t3662 = ct{1241};
t3665 = ct{1242};
t3666 = ct{1243};
t3667 = ct{1244};
t3668 = ct{1245};
t3669 = ct{1246};
t3670 = ct{1247};
t3671 = ct{1248};
t3673 = ct{1249};
t3679 = ct{1250};
t368 = ct{1251};
t3680 = ct{1252};
t3682 = ct{1253};
t3683 = ct{1254};
t3684 = ct{1255};
t3685 = ct{1256};
t3686 = ct{1257};
t3687 = ct{1258};
t3693 = ct{1259};
t3694 = ct{1260};
t3699 = ct{1261};
t37 = ct{1262};
t3701 = ct{1263};
t3702 = ct{1264};
t3708 = ct{1265};
t3709 = ct{1266};
t3710 = ct{1267};
t3712 = ct{1268};
t3715 = ct{1269};
t3716 = ct{1270};
t3719 = ct{1271};
t3732 = ct{1272};
t3734 = ct{1273};
t3739 = ct{1274};
t3741 = ct{1275};
t3745 = ct{1276};
t3747 = ct{1277};
t3749 = ct{1278};
t3750 = ct{1279};
t3751 = ct{1280};
t3754 = ct{1281};
t3755 = ct{1282};
t3756 = ct{1283};
t3757 = ct{1284};
t3762 = ct{1285};
t3770 = ct{1286};
t3771 = ct{1287};
t3772 = ct{1288};
t3780 = ct{1289};
t3781 = ct{1290};
t3785 = ct{1291};
t3787 = ct{1292};
t3788 = ct{1293};
t3789 = ct{1294};
t3795 = ct{1295};
t3799 = ct{1296};
t38 = ct{1297};
t3800 = ct{1298};
t3802 = ct{1299};
t3804 = ct{1300};
t3805 = ct{1301};
t3807 = ct{1302};
t3808 = ct{1303};
t3809 = ct{1304};
t3810 = ct{1305};
t3812 = ct{1306};
t3815 = ct{1307};
t3817 = ct{1308};
t3818 = ct{1309};
t3819 = ct{1310};
t3821 = ct{1311};
t3822 = ct{1312};
t3825 = ct{1313};
t3826 = ct{1314};
t3829 = ct{1315};
t3832 = ct{1316};
t3833 = ct{1317};
t3838 = ct{1318};
t3839 = ct{1319};
t3840 = ct{1320};
t3841 = ct{1321};
t3843 = ct{1322};
t3848 = ct{1323};
t3858 = ct{1324};
t3861 = ct{1325};
t3863 = ct{1326};
t3866 = ct{1327};
t3867 = ct{1328};
t3868 = ct{1329};
t3872 = ct{1330};
t3874 = ct{1331};
t3875 = ct{1332};
t3880 = ct{1333};
t3882 = ct{1334};
t3883 = ct{1335};
t3885 = ct{1336};
t3886 = ct{1337};
t3887 = ct{1338};
t3888 = ct{1339};
t3889 = ct{1340};
t3890 = ct{1341};
t3892 = ct{1342};
t3894 = ct{1343};
t3896 = ct{1344};
t3899 = ct{1345};
t39 = ct{1346};
t3900 = ct{1347};
t3901 = ct{1348};
t3903 = ct{1349};
t3904 = ct{1350};
t3908 = ct{1351};
t3912 = ct{1352};
t3913 = ct{1353};
t3917 = ct{1354};
t3919 = ct{1355};
t392 = ct{1356};
t3921 = ct{1357};
t3923 = ct{1358};
t3924 = ct{1359};
t3927 = ct{1360};
t3928 = ct{1361};
t393 = ct{1362};
t3931 = ct{1363};
t3932 = ct{1364};
t3933 = ct{1365};
t3934 = ct{1366};
t3935 = ct{1367};
t3936 = ct{1368};
t3937 = ct{1369};
t3938 = ct{1370};
t3942 = ct{1371};
t3943 = ct{1372};
t3944 = ct{1373};
t3956 = ct{1374};
t3958 = ct{1375};
t3960 = ct{1376};
t3962 = ct{1377};
t3964 = ct{1378};
t3965 = ct{1379};
t3966 = ct{1380};
t3967 = ct{1381};
t3969 = ct{1382};
t3971 = ct{1383};
t3972 = ct{1384};
t3975 = ct{1385};
t3976 = ct{1386};
t3977 = ct{1387};
t3978 = ct{1388};
t3979 = ct{1389};
t3982 = ct{1390};
t3984 = ct{1391};
t3986 = ct{1392};
t3989 = ct{1393};
t3990 = ct{1394};
t3991 = ct{1395};
t3992 = ct{1396};
t3994 = ct{1397};
t3997 = ct{1398};
t3999 = ct{1399};
t3d = ct{1400};
t3dd = ct{1401};
t4001 = ct{1402};
t4002 = ct{1403};
t4003 = ct{1404};
t4005 = ct{1405};
t4006 = ct{1406};
t4007 = ct{1407};
t4008 = ct{1408};
t4009 = ct{1409};
t401 = ct{1410};
t4010 = ct{1411};
t4011 = ct{1412};
t4012 = ct{1413};
t4016 = ct{1414};
t4017 = ct{1415};
t402 = ct{1416};
t4020 = ct{1417};
t4022 = ct{1418};
t4023 = ct{1419};
t4025 = ct{1420};
t4026 = ct{1421};
t4027 = ct{1422};
t403 = ct{1423};
t4034 = ct{1424};
t4036 = ct{1425};
t4038 = ct{1426};
t404 = ct{1427};
t4040 = ct{1428};
t4041 = ct{1429};
t4042 = ct{1430};
t4046 = ct{1431};
t4047 = ct{1432};
t4048 = ct{1433};
t4049 = ct{1434};
t4050 = ct{1435};
t4052 = ct{1436};
t4053 = ct{1437};
t4054 = ct{1438};
t4056 = ct{1439};
t4057 = ct{1440};
t4059 = ct{1441};
t4065 = ct{1442};
t4068 = ct{1443};
t4069 = ct{1444};
t4070 = ct{1445};
t4071 = ct{1446};
t4074 = ct{1447};
t4078 = ct{1448};
t4083 = ct{1449};
t4084 = ct{1450};
t4087 = ct{1451};
t4092 = ct{1452};
t4093 = ct{1453};
t4094 = ct{1454};
t4095 = ct{1455};
t4096 = ct{1456};
t41 = ct{1457};
t4101 = ct{1458};
t4102 = ct{1459};
t4108 = ct{1460};
t4115 = ct{1461};
t4117 = ct{1462};
t4118 = ct{1463};
t4121 = ct{1464};
t4122 = ct{1465};
t4125 = ct{1466};
t4127 = ct{1467};
t4128 = ct{1468};
t4130 = ct{1469};
t4131 = ct{1470};
t4133 = ct{1471};
t4136 = ct{1472};
t4137 = ct{1473};
t4139 = ct{1474};
t4143 = ct{1475};
t4146 = ct{1476};
t4147 = ct{1477};
t4149 = ct{1478};
t4151 = ct{1479};
t4152 = ct{1480};
t4154 = ct{1481};
t4155 = ct{1482};
t4156 = ct{1483};
t4157 = ct{1484};
t4159 = ct{1485};
t4161 = ct{1486};
t4163 = ct{1487};
t4164 = ct{1488};
t4166 = ct{1489};
t4167 = ct{1490};
t4168 = ct{1491};
t4170 = ct{1492};
t4171 = ct{1493};
t4172 = ct{1494};
t4174 = ct{1495};
t4176 = ct{1496};
t4178 = ct{1497};
t418 = ct{1498};
t4182 = ct{1499};
t4183 = ct{1500};
t4185 = ct{1501};
t4186 = ct{1502};
t4187 = ct{1503};
t4188 = ct{1504};
t4189 = ct{1505};
t419 = ct{1506};
t4190 = ct{1507};
t4191 = ct{1508};
t4192 = ct{1509};
t4193 = ct{1510};
t4195 = ct{1511};
t4196 = ct{1512};
t4197 = ct{1513};
t4198 = ct{1514};
t42 = ct{1515};
t420 = ct{1516};
t4200 = ct{1517};
t4201 = ct{1518};
t4203 = ct{1519};
t4204 = ct{1520};
t4206 = ct{1521};
t4212 = ct{1522};
t4213 = ct{1523};
t4214 = ct{1524};
t4218 = ct{1525};
t4221 = ct{1526};
t4223 = ct{1527};
t4224 = ct{1528};
t4226 = ct{1529};
t4227 = ct{1530};
t4228 = ct{1531};
t4229 = ct{1532};
t4230 = ct{1533};
t4231 = ct{1534};
t4233 = ct{1535};
t4235 = ct{1536};
t4236 = ct{1537};
t4237 = ct{1538};
t4238 = ct{1539};
t4241 = ct{1540};
t4242 = ct{1541};
t4243 = ct{1542};
t4246 = ct{1543};
t4249 = ct{1544};
t425 = ct{1545};
t4251 = ct{1546};
t4252 = ct{1547};
t4253 = ct{1548};
t4254 = ct{1549};
t4255 = ct{1550};
t4256 = ct{1551};
t4258 = ct{1552};
t4260 = ct{1553};
t4266 = ct{1554};
t4267 = ct{1555};
t4282 = ct{1556};
t4283 = ct{1557};
t4284 = ct{1558};
t4285 = ct{1559};
t4290 = ct{1560};
t4292 = ct{1561};
t4293 = ct{1562};
t4295 = ct{1563};
t4296 = ct{1564};
t4298 = ct{1565};
t4299 = ct{1566};
t4301 = ct{1567};
t4303 = ct{1568};
t4304 = ct{1569};
t4309 = ct{1570};
t431 = ct{1571};
t4311 = ct{1572};
t4312 = ct{1573};
t4317 = ct{1574};
t4319 = ct{1575};
t4321 = ct{1576};
t4324 = ct{1577};
t4325 = ct{1578};
t4327 = ct{1579};
t4328 = ct{1580};
t4330 = ct{1581};
t4331 = ct{1582};
t4332 = ct{1583};
t4333 = ct{1584};
t4335 = ct{1585};
t4336 = ct{1586};
t4337 = ct{1587};
t434 = ct{1588};
t4341 = ct{1589};
t4348 = ct{1590};
t4353 = ct{1591};
t4358 = ct{1592};
t4359 = ct{1593};
t4360 = ct{1594};
t4361 = ct{1595};
t4363 = ct{1596};
t4364 = ct{1597};
t4366 = ct{1598};
t4367 = ct{1599};
t437 = ct{1600};
t4371 = ct{1601};
t4372 = ct{1602};
t4388 = ct{1603};
t4394 = ct{1604};
t4395 = ct{1605};
t4396 = ct{1606};
t4399 = ct{1607};
t4402 = ct{1608};
t4403 = ct{1609};
t4404 = ct{1610};
t4406 = ct{1611};
t4407 = ct{1612};
t4408 = ct{1613};
t441 = ct{1614};
t4410 = ct{1615};
t4411 = ct{1616};
t4413 = ct{1617};
t442 = ct{1618};
t4420 = ct{1619};
t4421 = ct{1620};
t4423 = ct{1621};
t4424 = ct{1622};
t4427 = ct{1623};
t4428 = ct{1624};
t4429 = ct{1625};
t443 = ct{1626};
t4430 = ct{1627};
t4431 = ct{1628};
t4432 = ct{1629};
t4433 = ct{1630};
t4444 = ct{1631};
t4445 = ct{1632};
t4450 = ct{1633};
t4451 = ct{1634};
t4452 = ct{1635};
t4453 = ct{1636};
t4454 = ct{1637};
t4457 = ct{1638};
t4459 = ct{1639};
t446 = ct{1640};
t4460 = ct{1641};
t4461 = ct{1642};
t4464 = ct{1643};
t4467 = ct{1644};
t4468 = ct{1645};
t4470 = ct{1646};
t4473 = ct{1647};
t4474 = ct{1648};
t4475 = ct{1649};
t4476 = ct{1650};
t4479 = ct{1651};
t4480 = ct{1652};
t4483 = ct{1653};
t4487 = ct{1654};
t4488 = ct{1655};
t4491 = ct{1656};
t4493 = ct{1657};
t4494 = ct{1658};
t4500 = ct{1659};
t4503 = ct{1660};
t4506 = ct{1661};
t4508 = ct{1662};
t4509 = ct{1663};
t4514 = ct{1664};
t4515 = ct{1665};
t4517 = ct{1666};
t4519 = ct{1667};
t4526 = ct{1668};
t4528 = ct{1669};
t453 = ct{1670};
t4531 = ct{1671};
t4532 = ct{1672};
t4533 = ct{1673};
t4534 = ct{1674};
t4537 = ct{1675};
t4538 = ct{1676};
t4539 = ct{1677};
t454 = ct{1678};
t4540 = ct{1679};
t4541 = ct{1680};
t4542 = ct{1681};
t4543 = ct{1682};
t4546 = ct{1683};
t4547 = ct{1684};
t4548 = ct{1685};
t4550 = ct{1686};
t4551 = ct{1687};
t4552 = ct{1688};
t4553 = ct{1689};
t4556 = ct{1690};
t4561 = ct{1691};
t4562 = ct{1692};
t4565 = ct{1693};
t4568 = ct{1694};
t4572 = ct{1695};
t4575 = ct{1696};
t4576 = ct{1697};
t4578 = ct{1698};
t4579 = ct{1699};
t4582 = ct{1700};
t4583 = ct{1701};
t4587 = ct{1702};
t4588 = ct{1703};
t459 = ct{1704};
t4591 = ct{1705};
t4595 = ct{1706};
t4596 = ct{1707};
t4599 = ct{1708};
t4604 = ct{1709};
t4606 = ct{1710};
t4607 = ct{1711};
t4608 = ct{1712};
t4611 = ct{1713};
t4612 = ct{1714};
t4621 = ct{1715};
t4622 = ct{1716};
t4623 = ct{1717};
t4626 = ct{1718};
t4627 = ct{1719};
t4631 = ct{1720};
t4633 = ct{1721};
t4634 = ct{1722};
t4635 = ct{1723};
t4636 = ct{1724};
t4640 = ct{1725};
t4641 = ct{1726};
t4642 = ct{1727};
t4645 = ct{1728};
t4646 = ct{1729};
t4647 = ct{1730};
t4648 = ct{1731};
t4650 = ct{1732};
t4652 = ct{1733};
t4654 = ct{1734};
t4655 = ct{1735};
t4659 = ct{1736};
t4664 = ct{1737};
t4665 = ct{1738};
t4666 = ct{1739};
t4668 = ct{1740};
t4670 = ct{1741};
t4672 = ct{1742};
t4673 = ct{1743};
t4675 = ct{1744};
t4677 = ct{1745};
t4678 = ct{1746};
t4679 = ct{1747};
t4681 = ct{1748};
t4684 = ct{1749};
t4685 = ct{1750};
t4686 = ct{1751};
t4694 = ct{1752};
t4695 = ct{1753};
t4699 = ct{1754};
t470 = ct{1755};
t4700 = ct{1756};
t4701 = ct{1757};
t4702 = ct{1758};
t4703 = ct{1759};
t4704 = ct{1760};
t4705 = ct{1761};
t4707 = ct{1762};
t4708 = ct{1763};
t4710 = ct{1764};
t4713 = ct{1765};
t4714 = ct{1766};
t4715 = ct{1767};
t4716 = ct{1768};
t4717 = ct{1769};
t4720 = ct{1770};
t4721 = ct{1771};
t4722 = ct{1772};
t4723 = ct{1773};
t4724 = ct{1774};
t4725 = ct{1775};
t4727 = ct{1776};
t4730 = ct{1777};
t4732 = ct{1778};
t4737 = ct{1779};
t4738 = ct{1780};
t4739 = ct{1781};
t4741 = ct{1782};
t4744 = ct{1783};
t4747 = ct{1784};
t4757 = ct{1785};
t4758 = ct{1786};
t4759 = ct{1787};
t4760 = ct{1788};
t4762 = ct{1789};
t4765 = ct{1790};
t4766 = ct{1791};
t4767 = ct{1792};
t4768 = ct{1793};
t4770 = ct{1794};
t4771 = ct{1795};
t4776 = ct{1796};
t4777 = ct{1797};
t4778 = ct{1798};
t478 = ct{1799};
t4780 = ct{1800};
t4783 = ct{1801};
t4784 = ct{1802};
t4785 = ct{1803};
t4786 = ct{1804};
t4792 = ct{1805};
t4794 = ct{1806};
t4795 = ct{1807};
t4796 = ct{1808};
t4798 = ct{1809};
t48 = ct{1810};
t4807 = ct{1811};
t4810 = ct{1812};
t4813 = ct{1813};
t4815 = ct{1814};
t4817 = ct{1815};
t4822 = ct{1816};
t4825 = ct{1817};
t4828 = ct{1818};
t4829 = ct{1819};
t4830 = ct{1820};
t4831 = ct{1821};
t4836 = ct{1822};
t4837 = ct{1823};
t4838 = ct{1824};
t4840 = ct{1825};
t4841 = ct{1826};
t4843 = ct{1827};
t4845 = ct{1828};
t4846 = ct{1829};
t4849 = ct{1830};
t4851 = ct{1831};
t4855 = ct{1832};
t4856 = ct{1833};
t4858 = ct{1834};
t486 = ct{1835};
t4860 = ct{1836};
t4861 = ct{1837};
t4862 = ct{1838};
t4865 = ct{1839};
t4867 = ct{1840};
t487 = ct{1841};
t4870 = ct{1842};
t4873 = ct{1843};
t4874 = ct{1844};
t4875 = ct{1845};
t4878 = ct{1846};
t488 = ct{1847};
t4881 = ct{1848};
t4883 = ct{1849};
t4887 = ct{1850};
t4888 = ct{1851};
t4889 = ct{1852};
t4890 = ct{1853};
t4891 = ct{1854};
t4895 = ct{1855};
t4896 = ct{1856};
t4898 = ct{1857};
t4915 = ct{1858};
t4917 = ct{1859};
t492 = ct{1860};
t4920 = ct{1861};
t4922 = ct{1862};
t4923 = ct{1863};
t4925 = ct{1864};
t4926 = ct{1865};
t4929 = ct{1866};
t493 = ct{1867};
t4930 = ct{1868};
t4931 = ct{1869};
t4934 = ct{1870};
t4935 = ct{1871};
t4938 = ct{1872};
t494 = ct{1873};
t4941 = ct{1874};
t4942 = ct{1875};
t4943 = ct{1876};
t4946 = ct{1877};
t4949 = ct{1878};
t495 = ct{1879};
t4950 = ct{1880};
t4951 = ct{1881};
t4952 = ct{1882};
t4953 = ct{1883};
t4954 = ct{1884};
t4955 = ct{1885};
t4956 = ct{1886};
t4957 = ct{1887};
t4958 = ct{1888};
t4959 = ct{1889};
t496 = ct{1890};
t4960 = ct{1891};
t4967 = ct{1892};
t497 = ct{1893};
t4970 = ct{1894};
t4975 = ct{1895};
t4979 = ct{1896};
t4981 = ct{1897};
t4984 = ct{1898};
t4985 = ct{1899};
